simulink model "kinovaMicoSimscapeModel"  (R2021b)
(part 15 of 50)

Y2_9_1=(37*dq4*dqr3*sin(q5))/1000 - (37*dq4*dqr2*sin(q5))/1000 + dq5*dqr2*sin(q5)*((117*3^(1/2))/1250 - 37/2000) - dq5*dqr3*sin(q5)*((117*3^(1/2))/1250 - 37/2000) + (37*dq4*dqr2*cos(q4)^2*sin(q5))/500 - (37*dq4*dqr3*cos(q4)^2*sin(q5))/500 + (37*dq5*dqr2*cos(q4)^2*sin(q5))/2000 - (37*dq5*dqr3*cos(q4)^2*sin(q5))/2000 + (117*dq1*dqr1*cos(q4)*sin(q5))/625 - (234*dq1*dqr1*cos(q2)^2*cos(q4)*sin(q5))/625 - (234*dq1*dqr1*cos(q3)^2*cos(q4)*sin(q5))/625 - (29*3^(1/2)*dq1*dqr1*cos(q5)*sin(q3))/200 - (29*3^(1/2)*dq2*dqr3*cos(q5)*sin(q3))/200 - (29*3^(1/2)*dq3*dqr2*cos(q5)*sin(q3))/200 + (29*3^(1/2)*dq3*dqr3*cos(q5)*sin(q3))/200 - (29*3^(1/2)*dq5*dqr2*cos(q3)*sin(q5))/200 + (29*3^(1/2)*dq5*dqr3*cos(q3)*sin(q5))/200 + (29*dq1*dqr1*cos(q3)*cos(q4)*sin(q5))/100 + (29*dq1*dqr1*cos(q3)*cos(q5)*sin(q4))/200 - (37*dq1*dqr4*cos(q2)*cos(q5)*sin(q3))/1000 + (37*dq1*dqr4*cos(q3)*cos(q5)*sin(q2))/1000 - (37*dq4*dqr1*cos(q2)*cos(q5)*sin(q3))/1000 + (37*dq4*dqr1*cos(q3)*cos(q5)*sin(q2))/1000 - (29*dq1*dqr4*cos(q2)*cos(q5)*sin(q4))/200 - (29*dq4*dqr1*cos(q2)*cos(q4)*sin(q5))/100 - (29*dq4*dqr1*cos(q2)*cos(q5)*sin(q4))/200 - (37*dq5*dqr1*cos(q2)*cos(q5)*sin(q3))/1000 + (37*dq5*dqr1*cos(q3)*cos(q5)*sin(q2))/1000 + (29*dq2*dqr3*cos(q3)*cos(q4)*sin(q5))/100 + (29*dq2*dqr3*cos(q3)*cos(q5)*sin(q4))/200 + (29*dq3*dqr2*cos(q3)*cos(q4)*sin(q5))/100 + (29*dq3*dqr2*cos(q3)*cos(q5)*sin(q4))/200 - (29*dq5*dqr1*cos(q2)*cos(q4)*sin(q5))/200 - (29*dq5*dqr1*cos(q2)*cos(q5)*sin(q4))/100 + (29*dq2*dqr4*cos(q4)*cos(q5)*sin(q3))/200 - (29*dq3*dqr3*cos(q3)*cos(q4)*sin(q5))/100 - (29*dq3*dqr3*cos(q3)*cos(q5)*sin(q4))/200 + (29*dq4*dqr2*cos(q4)*cos(q5)*sin(q3))/200 - (29*dq3*dqr4*cos(q4)*cos(q5)*sin(q3))/200 + (37*dq4*dqr2*cos(q4)*cos(q5)*sin(q4))/1000 - (29*dq4*dqr3*cos(q4)*cos(q5)*sin(q3))/200 + (29*dq5*dqr2*cos(q4)*cos(q5)*sin(q3))/100 - (37*dq4*dqr3*cos(q4)*cos(q5)*sin(q4))/1000 + (37*dq5*dqr2*cos(q4)*cos(q5)*sin(q4))/1000 - (29*dq5*dqr3*cos(q4)*cos(q5)*sin(q3))/100 - (37*dq5*dqr3*cos(q4)*cos(q5)*sin(q4))/1000 - (29*dq2*dqr4*sin(q3)*sin(q4)*sin(q5))/100 - (29*dq4*dqr2*sin(q3)*sin(q4)*sin(q5))/100 + (29*dq3*dqr4*sin(q3)*sin(q4)*sin(q5))/100 + (29*dq4*dqr3*sin(q3)*sin(q4)*sin(q5))/100 - (29*dq5*dqr2*sin(q3)*sin(q4)*sin(q5))/200 + (29*dq5*dqr3*sin(q3)*sin(q4)*sin(q5))/200 - dq1*dqr1*cos(q5)*sin(q4)*((37*3^(1/2))/2000 - 117/1250) + dq1*dqr1*cos(q2)^2*cos(q5)*sin(q4)*((37*3^(1/2))/1000 - 117/625) + dq1*dqr1*cos(q3)^2*cos(q5)*sin(q4)*((37*3^(1/2))/1000 - 117/625) + (468*dq1*dqr1*cos(q2)^2*cos(q3)^2*cos(q4)*sin(q5))/625 + (29*3^(1/2)*dq1*dqr1*cos(q2)^2*cos(q5)*sin(q3))/100 + (117*dq4*dqr1*cos(q2)*cos(q3)*cos(q4)*sin(q5))/625 + (117*dq5*dqr1*cos(q2)*cos(q3)*cos(q4)*sin(q5))/1250 + (117*dq5*dqr1*cos(q2)*cos(q3)*cos(q5)*sin(q4))/625 + (117*dq1*dqr4*cos(q4)*sin(q2)*sin(q3)*sin(q5))/625 + (117*dq4*dqr1*cos(q4)*sin(q2)*sin(q3)*sin(q5))/625 + (117*dq5*dqr1*cos(q4)*sin(q2)*sin(q3)*sin(q5))/1250 + (117*dq5*dqr1*cos(q5)*sin(q2)*sin(q3)*sin(q4))/625 - dq1*dqr1*cos(q2)*cos(q5)*sin(q2)*((117*3^(1/2))/625 + 37/1000) + dq1*dqr1*cos(q3)*cos(q5)*sin(q3)*((117*3^(1/2))/625 + 37/1000) + (37*dq1*dqr1*cos(q2)*cos(q4)^2*cos(q5)*sin(q2))/1000 - (29*dq1*dqr1*cos(q2)^2*cos(q3)*cos(q4)*sin(q5))/50 - (29*dq1*dqr1*cos(q2)^2*cos(q3)*cos(q5)*sin(q4))/100 - (37*dq1*dqr1*cos(q3)*cos(q4)^2*cos(q5)*sin(q3))/1000 + (37*dq1*dqr4*cos(q2)*cos(q4)^2*cos(q5)*sin(q3))/1000 - (37*dq1*dqr4*cos(q3)*cos(q4)^2*cos(q5)*sin(q2))/1000 + (37*dq4*dqr1*cos(q2)*cos(q4)^2*cos(q5)*sin(q3))/1000 - (37*dq4*dqr1*cos(q3)*cos(q4)^2*cos(q5)*sin(q2))/1000 + (37*dq5*dqr1*cos(q2)*cos(q4)^2*cos(q5)*sin(q3))/1000 - (37*dq5*dqr1*cos(q3)*cos(q4)^2*cos(q5)*sin(q2))/1000 + dq1*dqr1*cos(q2)*cos(q3)^2*cos(q5)*sin(q2)*((234*3^(1/2))/625 + 37/500) - dq1*dqr1*cos(q2)^2*cos(q3)*cos(q5)*sin(q3)*((234*3^(1/2))/625 + 37/500) - (37*dq1*dqr1*cos(q2)*cos(q3)^2*cos(q4)^2*cos(q5)*sin(q2))/500 + (37*dq1*dqr1*cos(q2)^2*cos(q3)*cos(q4)^2*cos(q5)*sin(q3))/500 - dq1*dqr1*cos(q2)^2*cos(q3)^2*cos(q5)*sin(q4)*((37*3^(1/2))/500 - 234/625) - (29*dq1*dqr1*cos(q2)*cos(q4)*sin(q2)*sin(q3)*sin(q5))/50 - (29*dq1*dqr1*cos(q2)*cos(q5)*sin(q2)*sin(q3)*sin(q4))/100 - (37*dq1*dqr1*cos(q2)*cos(q4)*sin(q2)*sin(q4)*sin(q5))/500 + (37*dq1*dqr1*cos(q3)*cos(q4)*sin(q3)*sin(q4)*sin(q5))/500 - (37*dq1*dqr4*cos(q2)*cos(q4)*sin(q3)*sin(q4)*sin(q5))/500 + (37*dq1*dqr4*cos(q3)*cos(q4)*sin(q2)*sin(q4)*sin(q5))/500 - (37*dq4*dqr1*cos(q2)*cos(q4)*sin(q3)*sin(q4)*sin(q5))/500 + (37*dq4*dqr1*cos(q3)*cos(q4)*sin(q2)*sin(q4)*sin(q5))/500 - (37*dq5*dqr1*cos(q2)*cos(q4)*sin(q3)*sin(q4)*sin(q5))/2000 + (37*dq5*dqr1*cos(q3)*cos(q4)*sin(q2)*sin(q4)*sin(q5))/2000 - dq1*dqr4*cos(q2)*cos(q3)*cos(q5)*sin(q4)*((37*3^(1/2))/2000 - 117/1250) - dq4*dqr1*cos(q2)*cos(q3)*cos(q5)*sin(q4)*((37*3^(1/2))/2000 - 117/1250) - dq1*dqr4*cos(q5)*sin(q2)*sin(q3)*sin(q4)*((37*3^(1/2))/2000 - 117/1250) - dq4*dqr1*cos(q5)*sin(q2)*sin(q3)*sin(q4)*((37*3^(1/2))/2000 - 117/1250) - (29*3^(1/2)*dq1*dqr1*cos(q2)*cos(q3)*cos(q5)*sin(q2))/100 + (468*dq1*dqr1*cos(q2)*cos(q3)*cos(q4)*sin(q2)*sin(q3)*sin(q5))/625 + (37*dq1*dqr1*cos(q2)*cos(q3)^2*cos(q4)*sin(q2)*sin(q4)*sin(q5))/250 - (37*dq1*dqr1*cos(q2)^2*cos(q3)*cos(q4)*sin(q3)*sin(q4)*sin(q5))/250 - dq1*dqr1*cos(q2)*cos(q3)*cos(q5)*sin(q2)*sin(q3)*sin(q4)*((37*3^(1/2))/500 - 234/625);
Y2_9_2=(37*dq3*dqr4*sin(q5))/1000 - (37*dq2*dqr4*sin(q5))/1000 - (117*ddqr5*cos(q4)*cos(q5))/625 + (117*ddqr4*sin(q4)*sin(q5))/625 - ddqr2*cos(q5)*((117*3^(1/2))/625 - 37/1000) + ddqr3*cos(q5)*((117*3^(1/2))/625 - 37/1000) - (37*ddqr2*cos(q4)^2*cos(q5))/1000 + (37*ddqr3*cos(q4)^2*cos(q5))/1000 + dq2*dqr5*sin(q5)*((117*3^(1/2))/1250 - 37/2000) - dq3*dqr5*sin(q5)*((117*3^(1/2))/1250 - 37/2000) + (37*dq2*dqr4*cos(q4)^2*sin(q5))/500 + (37*dq2*dqr5*cos(q4)^2*sin(q5))/2000 - (37*dq3*dqr4*cos(q4)^2*sin(q5))/500 - (37*dq3*dqr5*cos(q4)^2*sin(q5))/2000 + (29*ddqr1*cos(q2)*cos(q4)*cos(q5))/200 + (29*ddqr4*cos(q3)*cos(q4)*cos(q5))/200 + (29*ddqr5*cos(q3)*cos(q4)*cos(q5))/100 - (37*ddqr1*cos(q2)*sin(q3)*sin(q5))/1000 + (37*ddqr1*cos(q3)*sin(q2)*sin(q5))/1000 - (29*ddqr1*cos(q2)*sin(q4)*sin(q5))/100 + (29*ddqr2*cos(q4)*sin(q3)*sin(q5))/50 + (29*ddqr2*cos(q5)*sin(q3)*sin(q4))/100 + (37*ddqr2*cos(q4)*sin(q4)*sin(q5))/500 - (29*ddqr3*cos(q4)*sin(q3)*sin(q5))/100 - (29*ddqr3*cos(q5)*sin(q3)*sin(q4))/200 - (37*ddqr3*cos(q4)*sin(q4)*sin(q5))/500 - (29*ddqr4*cos(q3)*sin(q4)*sin(q5))/100 - (29*ddqr5*cos(q3)*sin(q4)*sin(q5))/200 + ddqr4*cos(q4)*cos(q5)*((37*3^(1/2))/2000 - 117/1250) + ddqr5*sin(q4)*sin(q5)*((37*3^(1/2))/2000 + 117/1250) + (29*3^(1/2)*ddqr2*cos(q3)*cos(q5))/100 - (29*3^(1/2)*ddqr3*cos(q3)*cos(q5))/200 + (117*dq4*dqr4*cos(q4)*sin(q5))/625 + (117*dq4*dqr5*cos(q4)*sin(q5))/1250 + (117*dq4*dqr5*cos(q5)*sin(q4))/625 + (117*dq5*dqr4*cos(q4)*sin(q5))/1250 + (117*dq5*dqr4*cos(q5)*sin(q4))/625 + (117*dq5*dqr5*cos(q4)*sin(q5))/625 + (29*3^(1/2)*ddqr5*sin(q3)*sin(q5))/200 + (117*ddqr1*cos(q2)*cos(q3)*sin(q4)*sin(q5))/625 - (7*ddqr1*cos(q2)*cos(q4)*sin(q3)*sin(q5))/1000 - (7*ddqr1*cos(q2)*cos(q5)*sin(q3)*sin(q4))/2000 + (7*ddqr1*cos(q3)*cos(q4)*sin(q2)*sin(q5))/1000 + (7*ddqr1*cos(q3)*cos(q5)*sin(q2)*sin(q4))/2000 - (29*3^(1/2)*dq2*dqr5*cos(q3)*sin(q5))/200 + (29*3^(1/2)*dq3*dqr5*cos(q3)*sin(q5))/200 + (29*3^(1/2)*dq5*dqr5*cos(q5)*sin(q3))/200 + (117*ddqr1*sin(q2)*sin(q3)*sin(q4)*sin(q5))/625 + (37*ddqr1*cos(q2)*cos(q4)^2*sin(q3)*sin(q5))/500 - (37*ddqr1*cos(q3)*cos(q4)^2*sin(q2)*sin(q5))/500 - (7*3^(1/2)*ddqr1*cos(q2)*cos(q3)*cos(q5))/2000 - (29*dq1*dqr4*cos(q2)*cos(q4)*sin(q5))/100 - (37*dq1*dqr5*cos(q2)*cos(q5)*sin(q3))/1000 + (37*dq1*dqr5*cos(q3)*cos(q5)*sin(q2))/1000 - (29*dq1*dqr5*cos(q2)*cos(q4)*sin(q5))/200 - (29*dq1*dqr5*cos(q2)*cos(q5)*sin(q4))/100 + (37*dq2*dqr4*cos(q4)*cos(q5)*sin(q4))/1000 + (29*dq2*dqr5*cos(q4)*cos(q5)*sin(q3))/100 + (37*dq2*dqr5*cos(q4)*cos(q5)*sin(q4))/1000 - (37*dq3*dqr4*cos(q4)*cos(q5)*sin(q4))/1000 - (29*dq3*dqr5*cos(q4)*cos(q5)*sin(q3))/100 - (29*dq4*dqr4*cos(q3)*cos(q4)*sin(q5))/100 - (29*dq4*dqr4*cos(q3)*cos(q5)*sin(q4))/200 - (37*dq3*dqr5*cos(q4)*cos(q5)*sin(q4))/1000 - (29*dq4*dqr5*cos(q3)*cos(q4)*sin(q5))/200 - (29*dq4*dqr5*cos(q3)*cos(q5)*sin(q4))/100 - (29*dq5*dqr4*cos(q3)*cos(q4)*sin(q5))/200 - (29*dq5*dqr4*cos(q3)*cos(q5)*sin(q4))/100 - (29*dq5*dqr5*cos(q3)*cos(q4)*sin(q5))/100 - (29*dq5*dqr5*cos(q3)*cos(q5)*sin(q4))/200 - (7*3^(1/2)*ddqr1*cos(q5)*sin(q2)*sin(q3))/2000 - (29*dq2*dqr5*sin(q3)*sin(q4)*sin(q5))/200 + (29*dq3*dqr5*sin(q3)*sin(q4)*sin(q5))/200 - dq4*dqr4*cos(q5)*sin(q4)*((37*3^(1/2))/2000 - 117/1250) + dq5*dqr5*cos(q5)*sin(q4)*((37*3^(1/2))/2000 + 117/1250) + (37*ddqr1*cos(q2)*cos(q4)*cos(q5)*sin(q3)*sin(q4))/1000 - (37*ddqr1*cos(q3)*cos(q4)*cos(q5)*sin(q2)*sin(q4))/1000 + ddqr1*cos(q2)*cos(q3)*cos(q4)*cos(q5)*((37*3^(1/2))/2000 - 117/1250) + ddqr1*cos(q4)*cos(q5)*sin(q2)*sin(q3)*((37*3^(1/2))/2000 - 117/1250) + (117*dq1*dqr4*cos(q2)*cos(q3)*cos(q4)*sin(q5))/625 + (117*dq1*dqr5*cos(q2)*cos(q3)*cos(q4)*sin(q5))/1250 + (117*dq1*dqr5*cos(q2)*cos(q3)*cos(q5)*sin(q4))/625 + (117*dq1*dqr5*cos(q4)*sin(q2)*sin(q3)*sin(q5))/1250 + (117*dq1*dqr5*cos(q5)*sin(q2)*sin(q3)*sin(q4))/625 + (37*dq1*dqr5*cos(q2)*cos(q4)^2*cos(q5)*sin(q3))/1000 - (37*dq1*dqr5*cos(q3)*cos(q4)^2*cos(q5)*sin(q2))/1000 - (37*dq1*dqr5*cos(q2)*cos(q4)*sin(q3)*sin(q4)*sin(q5))/2000 + (37*dq1*dqr5*cos(q3)*cos(q4)*sin(q2)*sin(q4)*sin(q5))/2000;
Y2_10_1=dq1*dqr1*cos(q2)*cos(q3)^2*cos(q6)*sin(q2)*((1231*3^(1/2))/10000 - 111/1000) - (2631*dq6*dqr1*cos(q4)*sin(q2)*sin(q3)*sin(q6))/16000 - dq1*dqr1*cos(q2)*cos(q4)^2*cos(q6)*sin(q2)*((1923*3^(1/2))/40000 + 37/400) + (37*3^(1/2)*dq4*dqr1*cos(q4)*sin(q2)*sin(q3)*sin(q6))/2000 + (37*3^(1/2)*dq5*dqr1*cos(q4)*sin(q2)*sin(q3)*sin(q6))/4000 - (37*dq1*dqr1*cos(q2)*cos(q3)^2*cos(q5)^2*cos(q6)*sin(q2))/1000 + (37*dq1*dqr1*cos(q2)*cos(q4)^2*cos(q5)^2*cos(q6)*sin(q2))/800 + (87*dq1*dqr1*cos(q2)*cos(q6)*sin(q2)*sin(q3)*sin(q4))/200 + (37*dq1*dqr1*cos(q2)*cos(q4)*sin(q2)*sin(q4)*sin(q6))/1000 - (37*dq1*dqr1*cos(q2)*cos(q5)*sin(q2)*sin(q5)*sin(q6))/1000 - (37*dq4*dqr1*cos(q3)*cos(q4)*sin(q2)*sin(q4)*sin(q6))/1000 - (877*dq4*dqr1*cos(q4)*cos(q5)*sin(q2)*sin(q3)*sin(q6))/4000 - (1231*dq4*dqr1*cos(q5)*cos(q6)*sin(q2)*sin(q3)*sin(q4))/40000 - (37*dq5*dqr1*cos(q3)*cos(q4)*sin(q2)*sin(q4)*sin(q6))/800 - (37*dq4*dqr1*cos(q3)*cos(q5)*sin(q2)*sin(q5)*sin(q6))/2000 - (877*dq5*dqr1*cos(q4)*cos(q5)*sin(q2)*sin(q3)*sin(q6))/8000 - (37*dq5*dqr1*cos(q3)*cos(q5)*sin(q2)*sin(q5)*sin(q6))/1000 - (877*dq6*dqr1*cos(q4)*cos(q6)*sin(q2)*sin(q3)*sin(q5))/8000 - (877*dq6*dqr1*cos(q5)*cos(q6)*sin(q2)*sin(q3)*sin(q4))/4000 - (37*dq6*dqr1*cos(q3)*cos(q5)*sin(q2)*sin(q5)*sin(q6))/4000 + (877*dq5*dqr1*sin(q2)*sin(q3)*sin(q4)*sin(q5)*sin(q6))/4000 + (877*dq6*dqr1*sin(q2)*sin(q3)*sin(q4)*sin(q5)*sin(q6))/8000 - dq1*dqr1*cos(q2)*sin(q2)*sin(q5)*sin(q6)*((2513*3^(1/2))/10000 + 37/1000) + dq4*dqr1*cos(q3)*sin(q2)*sin(q5)*sin(q6)*((641*3^(1/2))/20000 + 37/1000) + dq5*dqr1*cos(q3)*sin(q2)*sin(q5)*sin(q6)*((641*3^(1/2))/20000 + 37/1000) + dq6*dqr1*cos(q3)*sin(q2)*sin(q5)*sin(q6)*((641*3^(1/2))/40000 + 37/2000) - dq4*dqr1*cos(q6)*sin(q2)*sin(q3)*sin(q4)*((37*3^(1/2))/4000 + 7539/40000) - (29*3^(1/2)*dq1*dqr1*cos(q2)*cos(q3)*cos(q6)*sin(q2))/200 + dq1*dqr1*cos(q2)*cos(q3)^2*cos(q4)^2*cos(q6)*sin(q2)*((1923*3^(1/2))/20000 + 37/200) - (37*3^(1/2)*dq4*dqr1*cos(q4)*cos(q5)^2*sin(q2)*sin(q3)*sin(q6))/1000 - (37*3^(1/2)*dq4*dqr1*cos(q5)^2*cos(q6)*sin(q2)*sin(q3)*sin(q4))/4000 - (37*3^(1/2)*dq5*dqr1*cos(q4)*cos(q5)^2*sin(q2)*sin(q3)*sin(q6))/2000 - (37*3^(1/2)*dq5*dqr1*cos(q5)^2*cos(q6)*sin(q2)*sin(q3)*sin(q4))/2000 - (37*3^(1/2)*dq6*dqr1*cos(q4)*cos(q5)^2*sin(q2)*sin(q3)*sin(q6))/8000 - (37*3^(1/2)*dq6*dqr1*cos(q5)^2*cos(q6)*sin(q2)*sin(q3)*sin(q4))/2000 - (37*dq1*dqr1*cos(q2)*cos(q3)^2*cos(q4)^2*cos(q5)^2*cos(q6)*sin(q2))/400 + (29*dq1*dqr1*cos(q2)*cos(q4)*cos(q5)*sin(q2)*sin(q3)*sin(q6))/50 + (29*dq1*dqr1*cos(q2)*cos(q4)*cos(q6)*sin(q2)*sin(q3)*sin(q5))/100 + (29*dq1*dqr1*cos(q2)*cos(q5)*cos(q6)*sin(q2)*sin(q3)*sin(q4))/200 - (29*dq1*dqr1*cos(q2)*sin(q2)*sin(q3)*sin(q4)*sin(q5)*sin(q6))/100 + dq4*dqr1*cos(q4)*cos(q6)*sin(q2)*sin(q3)*sin(q5)*((37*3^(1/2))/4000 - 877/8000) + dq5*dqr1*cos(q5)*cos(q6)*sin(q2)*sin(q3)*sin(q4)*((37*3^(1/2))/4000 - 877/8000) + dq5*dqr1*cos(q4)*cos(q6)*sin(q2)*sin(q3)*sin(q5)*((37*3^(1/2))/8000 - 877/16000) - dq6*dqr1*cos(q4)*cos(q5)*sin(q2)*sin(q3)*sin(q6)*((111*3^(1/2))/8000 + 877/16000) - dq6*dqr1*cos(q3)*cos(q4)*sin(q2)*sin(q4)*sin(q6)*((1923*3^(1/2))/80000 + 37/800) - (37*dq1*dqr1*cos(q2)*cos(q3)^2*cos(q4)*sin(q2)*sin(q4)*sin(q6))/500 - (37*dq1*dqr1*cos(q2)*cos(q4)*cos(q5)^2*sin(q2)*sin(q4)*sin(q6))/500 + (37*dq1*dqr1*cos(q2)*cos(q3)^2*cos(q5)*sin(q2)*sin(q5)*sin(q6))/500 - (37*dq1*dqr1*cos(q2)*cos(q4)^2*cos(q5)*sin(q2)*sin(q5)*sin(q6))/400 + (37*dq4*dqr1*cos(q3)*cos(q4)*cos(q5)^2*sin(q2)*sin(q4)*sin(q6))/500 + (37*dq4*dqr1*cos(q3)*cos(q4)^2*cos(q5)*sin(q2)*sin(q5)*sin(q6))/400 + (37*dq5*dqr1*cos(q3)*cos(q4)*cos(q5)^2*sin(q2)*sin(q4)*sin(q6))/400 + (37*dq5*dqr1*cos(q3)*cos(q4)^2*cos(q5)*sin(q2)*sin(q5)*sin(q6))/500 + (37*dq6*dqr1*cos(q3)*cos(q4)*cos(q5)^2*sin(q2)*sin(q4)*sin(q6))/1600 + (37*dq6*dqr1*cos(q3)*cos(q4)^2*cos(q5)*sin(q2)*sin(q5)*sin(q6))/2000 - dq4*dqr1*sin(q2)*sin(q3)*sin(q4)*sin(q5)*sin(q6)*((37*3^(1/2))/2000 - 1231/20000) + (29*3^(1/2)*dq1*dqr1*cos(q2)*cos(q3)*cos(q5)*cos(q6)*sin(q2))/200 - dq1*dqr1*cos(q2)*cos(q3)^2*cos(q5)*cos(q6)*sin(q2)*((2513*3^(1/2))/10000 - 37/500) - dq1*dqr1*cos(q2)*cos(q4)^2*cos(q5)*cos(q6)*sin(q2)*((641*3^(1/2))/40000 - 37/4000) - (29*3^(1/2)*dq1*dqr1*cos(q2)*cos(q3)*sin(q2)*sin(q5)*sin(q6))/100 + dq1*dqr1*cos(q2)*cos(q3)^2*sin(q2)*sin(q5)*sin(q6)*((2513*3^(1/2))/5000 + 37/500) + dq1*dqr1*cos(q2)*cos(q4)^2*sin(q2)*sin(q5)*sin(q6)*((641*3^(1/2))/20000 + 37/1000) - dq4*dqr1*cos(q3)*cos(q4)^2*sin(q2)*sin(q5)*sin(q6)*((641*3^(1/2))/20000 + 37/1000) - dq5*dqr1*cos(q3)*cos(q4)^2*sin(q2)*sin(q5)*sin(q6)*((641*3^(1/2))/20000 + 37/1000) - dq6*dqr1*cos(q3)*cos(q4)^2*sin(q2)*sin(q5)*sin(q6)*((641*3^(1/2))/40000 - 37/4000) + dq1*dqr1*cos(q2)*cos(q3)^2*cos(q4)^2*cos(q5)*cos(q6)*sin(q2)*((641*3^(1/2))/20000 - 37/2000) - (877*dq1*dqr1*cos(q2)*cos(q3)*cos(q4)*cos(q5)*sin(q2)*sin(q3)*sin(q6))/1000 - (1231*dq1*dqr1*cos(q2)*cos(q3)*cos(q5)*cos(q6)*sin(q2)*sin(q3)*sin(q4))/10000 - (37*dq1*dqr1*cos(q2)*cos(q4)*cos(q5)*cos(q6)*sin(q2)*sin(q4)*sin(q5))/1000 + (37*dq4*dqr1*cos(q3)*cos(q4)*cos(q5)*cos(q6)*sin(q2)*sin(q4)*sin(q5))/1000 + (37*dq5*dqr1*cos(q3)*cos(q4)*cos(q5)*cos(q6)*sin(q2)*sin(q4)*sin(q5))/800 + (37*dq6*dqr1*cos(q3)*cos(q4)*cos(q5)*cos(q6)*sin(q2)*sin(q4)*sin(q5))/800 - dq1*dqr1*cos(q2)*cos(q3)^2*cos(q4)^2*sin(q2)*sin(q5)*sin(q6)*((641*3^(1/2))/10000 + 37/500) + dq1*dqr1*cos(q2)*cos(q4)*cos(q5)*sin(q2)*sin(q4)*sin(q6)*((641*3^(1/2))/10000 + 37/500) - dq4*dqr1*cos(q3)*cos(q4)*cos(q5)*sin(q2)*sin(q4)*sin(q6)*((641*3^(1/2))/10000 + 37/500) - dq1*dqr1*cos(q2)*cos(q3)*cos(q6)*sin(q2)*sin(q3)*sin(q4)*((37*3^(1/2))/1000 + 7539/10000) + dq1*dqr1*cos(q2)*cos(q4)*cos(q6)*sin(q2)*sin(q4)*sin(q5)*((641*3^(1/2))/20000 - 37/2000) - dq4*dqr1*cos(q3)*cos(q4)*cos(q6)*sin(q2)*sin(q4)*sin(q5)*((641*3^(1/2))/20000 - 37/2000) - dq5*dqr1*cos(q3)*cos(q4)*cos(q5)*sin(q2)*sin(q4)*sin(q6)*((641*3^(1/2))/40000 + 37/2000) - dq6*dqr1*cos(q3)*cos(q4)*cos(q6)*sin(q2)*sin(q4)*sin(q5)*((641*3^(1/2))/40000 + 37/2000) - dq5*dqr1*cos(q3)*cos(q4)*cos(q6)*sin(q2)*sin(q4)*sin(q5)*((641*3^(1/2))/80000 - 37/8000) - dq6*dqr1*cos(q3)*cos(q4)*cos(q5)*sin(q2)*sin(q4)*sin(q6)*((641*3^(1/2))/80000 - 37/8000) + (37*3^(1/2)*dq1*dqr1*cos(q2)*cos(q3)*cos(q4)*sin(q2)*sin(q3)*sin(q6))/500 - (37*3^(1/2)*dq4*dqr1*cos(q4)*cos(q5)*cos(q6)*sin(q2)*sin(q3)*sin(q5))/2000 - (37*3^(1/2)*dq5*dqr1*cos(q4)*cos(q5)*cos(q6)*sin(q2)*sin(q3)*sin(q5))/4000 - (37*3^(1/2)*dq6*dqr1*cos(q4)*cos(q5)*cos(q6)*sin(q2)*sin(q3)*sin(q5))/4000 + (37*3^(1/2)*dq4*dqr1*cos(q5)*sin(q2)*sin(q3)*sin(q4)*sin(q5)*sin(q6))/2000 + (37*3^(1/2)*dq5*dqr1*cos(q5)*sin(q2)*sin(q3)*sin(q4)*sin(q5)*sin(q6))/1000 + (37*3^(1/2)*dq6*dqr1*cos(q5)*sin(q2)*sin(q3)*sin(q4)*sin(q5)*sin(q6))/4000 + (37*dq1*dqr1*cos(q2)*cos(q3)^2*cos(q4)*cos(q5)^2*sin(q2)*sin(q4)*sin(q6))/250 + (37*dq1*dqr1*cos(q2)*cos(q3)^2*cos(q4)^2*cos(q5)*sin(q2)*sin(q5)*sin(q6))/200 + dq1*dqr1*cos(q2)*cos(q3)*cos(q4)*cos(q6)*sin(q2)*sin(q3)*sin(q5)*((37*3^(1/2))/1000 - 877/2000) + (37*dq1*dqr1*cos(q2)*cos(q3)^2*cos(q4)*cos(q5)*cos(q6)*sin(q2)*sin(q4)*sin(q5))/500 - dq1*dqr1*cos(q2)*cos(q3)*sin(q2)*sin(q3)*sin(q4)*sin(q5)*sin(q6)*((37*3^(1/2))/500 - 1231/5000) - dq1*dqr1*cos(q2)*cos(q3)^2*cos(q4)*cos(q5)*sin(q2)*sin(q4)*sin(q6)*((641*3^(1/2))/5000 + 37/250) - dq1*dqr1*cos(q2)*cos(q3)^2*cos(q4)*cos(q6)*sin(q2)*sin(q4)*sin(q5)*((641*3^(1/2))/10000 - 37/1000) - (37*3^(1/2)*dq1*dqr1*cos(q2)*cos(q3)*cos(q4)*cos(q5)^2*sin(q2)*sin(q3)*sin(q6))/250 - (37*3^(1/2)*dq1*dqr1*cos(q2)*cos(q3)*cos(q5)^2*cos(q6)*sin(q2)*sin(q3)*sin(q4))/1000 - (37*3^(1/2)*dq1*dqr1*cos(q2)*cos(q3)*cos(q4)*cos(q5)*cos(q6)*sin(q2)*sin(q3)*sin(q5))/500 + (37*3^(1/2)*dq1*dqr1*cos(q2)*cos(q3)*cos(q5)*sin(q2)*sin(q3)*sin(q4)*sin(q5)*sin(q6))/500;
Y2_10_2=(29*3^(1/2)*dq1*dqr1*cos(q5)*cos(q6)*sin(q3))/400 - (29*3^(1/2)*dq1*dqr1*cos(q6)*sin(q3))/400 - (29*3^(1/2)*dq1*dqr1*sin(q3)*sin(q5)*sin(q6))/200 + (29*3^(1/2)*dq1*dqr1*cos(q2)^2*cos(q6)*sin(q3))/200 - dq1*dqr1*cos(q2)*cos(q6)*sin(q2)*((1231*3^(1/2))/20000 - 111/2000) + dq1*dqr1*cos(q3)*cos(q6)*sin(q3)*((1231*3^(1/2))/20000 - 111/2000) + dq4*dqr1*cos(q2)*cos(q6)*sin(q3)*((1923*3^(1/2))/40000 + 111/2000) - dq4*dqr1*cos(q3)*cos(q6)*sin(q2)*((1923*3^(1/2))/40000 + 111/2000) + (37*dq1*dqr1*cos(q2)*cos(q5)^2*cos(q6)*sin(q2))/2000 - (37*dq1*dqr1*cos(q3)*cos(q5)^2*cos(q6)*sin(q3))/2000 - (37*dq4*dqr1*cos(q2)*cos(q5)^2*cos(q6)*sin(q3))/4000 + (37*dq4*dqr1*cos(q3)*cos(q5)^2*cos(q6)*sin(q2))/4000 - (37*dq5*dqr1*cos(q2)*cos(q4)^2*cos(q6)*sin(q3))/2000 + (37*dq5*dqr1*cos(q3)*cos(q4)^2*cos(q6)*sin(q2))/2000 - (37*dq5*dqr1*cos(q2)*cos(q5)^2*cos(q6)*sin(q3))/2000 + (37*dq5*dqr1*cos(q3)*cos(q5)^2*cos(q6)*sin(q2))/2000 - (37*dq6*dqr1*cos(q2)*cos(q4)^2*cos(q6)*sin(q3))/2000 + (37*dq6*dqr1*cos(q3)*cos(q4)^2*cos(q6)*sin(q2))/2000 - (37*dq6*dqr1*cos(q2)*cos(q5)^2*cos(q6)*sin(q3))/2000 + (37*dq6*dqr1*cos(q3)*cos(q5)^2*cos(q6)*sin(q2))/2000 - dq1*dqr1*cos(q2)^2*cos(q3)*cos(q6)*sin(q3)*((1231*3^(1/2))/10000 - 111/1000) + dq1*dqr1*cos(q3)*cos(q4)^2*cos(q6)*sin(q3)*((1923*3^(1/2))/40000 + 37/400) - dq4*dqr1*cos(q2)*cos(q4)^2*cos(q6)*sin(q3)*((1923*3^(1/2))/40000 + 37/400) + dq4*dqr1*cos(q3)*cos(q4)^2*cos(q6)*sin(q2)*((1923*3^(1/2))/40000 + 37/400) + (37*dq1*dqr1*cos(q2)^2*cos(q3)*cos(q5)^2*cos(q6)*sin(q3))/1000 - (37*dq1*dqr1*cos(q3)*cos(q4)^2*cos(q5)^2*cos(q6)*sin(q3))/800 + (37*dq4*dqr1*cos(q2)*cos(q4)^2*cos(q5)^2*cos(q6)*sin(q3))/800 - (37*dq4*dqr1*cos(q3)*cos(q4)^2*cos(q5)^2*cos(q6)*sin(q2))/800 + (37*dq5*dqr1*cos(q2)*cos(q4)^2*cos(q5)^2*cos(q6)*sin(q3))/1000 - (37*dq5*dqr1*cos(q3)*cos(q4)^2*cos(q5)^2*cos(q6)*sin(q2))/1000 + (37*dq6*dqr1*cos(q2)*cos(q4)^2*cos(q5)^2*cos(q6)*sin(q3))/1000 - (37*dq6*dqr1*cos(q3)*cos(q4)^2*cos(q5)^2*cos(q6)*sin(q2))/1000 - (29*3^(1/2)*dq1*dqr1*cos(q2)^2*cos(q5)*cos(q6)*sin(q3))/200 + (29*3^(1/2)*dq1*dqr1*cos(q2)^2*sin(q3)*sin(q5)*sin(q6))/100 - (37*dq1*dqr1*cos(q3)*cos(q4)*sin(q3)*sin(q4)*sin(q6))/1000 + (37*dq1*dqr1*cos(q3)*cos(q5)*sin(q3)*sin(q5)*sin(q6))/1000 + (37*dq4*dqr1*cos(q2)*cos(q4)*sin(q3)*sin(q4)*sin(q6))/1000 + (37*dq5*dqr1*cos(q2)*cos(q4)*sin(q3)*sin(q4)*sin(q6))/800 + (37*dq4*dqr1*cos(q2)*cos(q5)*sin(q3)*sin(q5)*sin(q6))/2000 + (37*dq5*dqr1*cos(q2)*cos(q5)*sin(q3)*sin(q5)*sin(q6))/1000 + (37*dq6*dqr1*cos(q2)*cos(q5)*sin(q3)*sin(q5)*sin(q6))/4000 + dq6*dqr1*cos(q2)*cos(q5)*cos(q6)*sin(q3)*((641*3^(1/2))/20000 + 37/1000) - dq6*dqr1*cos(q3)*cos(q5)*cos(q6)*sin(q2)*((641*3^(1/2))/20000 + 37/1000) + dq1*dqr1*cos(q2)*cos(q5)*cos(q6)*sin(q2)*((2513*3^(1/2))/20000 - 37/1000) - dq1*dqr1*cos(q3)*cos(q5)*cos(q6)*sin(q3)*((2513*3^(1/2))/20000 - 37/1000) + dq4*dqr1*cos(q2)*cos(q5)*cos(q6)*sin(q3)*((641*3^(1/2))/40000 - 37/4000) - dq4*dqr1*cos(q3)*cos(q5)*cos(q6)*sin(q2)*((641*3^(1/2))/40000 - 37/4000) + dq5*dqr1*cos(q2)*cos(q5)*cos(q6)*sin(q3)*((641*3^(1/2))/40000 - 37/4000) - dq5*dqr1*cos(q3)*cos(q5)*cos(q6)*sin(q2)*((641*3^(1/2))/40000 - 37/4000) + dq1*dqr1*cos(q3)*sin(q3)*sin(q5)*sin(q6)*((2513*3^(1/2))/10000 + 37/1000) - dq4*dqr1*cos(q2)*sin(q3)*sin(q5)*sin(q6)*((641*3^(1/2))/20000 + 37/1000) - dq5*dqr1*cos(q2)*sin(q3)*sin(q5)*sin(q6)*((641*3^(1/2))/20000 + 37/1000) - dq6*dqr1*cos(q2)*sin(q3)*sin(q5)*sin(q6)*((641*3^(1/2))/40000 + 37/2000) - dq1*dqr1*cos(q2)^2*cos(q3)*cos(q4)^2*cos(q6)*sin(q3)*((1923*3^(1/2))/20000 + 37/200) + (37*dq1*dqr1*cos(q2)^2*cos(q3)*cos(q4)^2*cos(q5)^2*cos(q6)*sin(q3))/400 - dq1*dqr1*cos(q2)^2*cos(q3)^2*sin(q4)*sin(q5)*sin(q6)*((37*3^(1/2))/500 - 1231/5000) + dq6*dqr1*cos(q2)*cos(q4)*sin(q3)*sin(q4)*sin(q6)*((1923*3^(1/2))/80000 + 37/800) + (37*dq1*dqr1*cos(q2)^2*cos(q3)*cos(q4)*sin(q3)*sin(q4)*sin(q6))/500 - (37*dq1*dqr1*cos(q2)^2*cos(q3)*cos(q5)*sin(q3)*sin(q5)*sin(q6))/500 + (37*dq1*dqr1*cos(q3)*cos(q4)*cos(q5)^2*sin(q3)*sin(q4)*sin(q6))/500 + (37*dq1*dqr1*cos(q3)*cos(q4)^2*cos(q5)*sin(q3)*sin(q5)*sin(q6))/400 - (37*dq4*dqr1*cos(q2)*cos(q4)*cos(q5)^2*sin(q3)*sin(q4)*sin(q6))/500 - (37*dq4*dqr1*cos(q2)*cos(q4)^2*cos(q5)*sin(q3)*sin(q5)*sin(q6))/400 - (37*dq5*dqr1*cos(q2)*cos(q4)*cos(q5)^2*sin(q3)*sin(q4)*sin(q6))/400 - (37*dq5*dqr1*cos(q2)*cos(q4)^2*cos(q5)*sin(q3)*sin(q5)*sin(q6))/500 - (37*dq6*dqr1*cos(q2)*cos(q4)*cos(q5)^2*sin(q3)*sin(q4)*sin(q6))/1600 - (37*dq6*dqr1*cos(q2)*cos(q4)^2*cos(q5)*sin(q3)*sin(q5)*sin(q6))/2000 + dq1*dqr1*cos(q2)^2*cos(q3)*cos(q5)*cos(q6)*sin(q3)*((2513*3^(1/2))/10000 - 37/500) - dq6*dqr1*cos(q2)*cos(q4)^2*cos(q5)*cos(q6)*sin(q3)*((641*3^(1/2))/20000 + 37/1000) + dq6*dqr1*cos(q3)*cos(q4)^2*cos(q5)*cos(q6)*sin(q2)*((641*3^(1/2))/20000 + 37/1000) + dq1*dqr1*cos(q3)*cos(q4)^2*cos(q5)*cos(q6)*sin(q3)*((641*3^(1/2))/40000 - 37/4000) - dq4*dqr1*cos(q2)*cos(q4)^2*cos(q5)*cos(q6)*sin(q3)*((641*3^(1/2))/40000 - 37/4000) + dq4*dqr1*cos(q3)*cos(q4)^2*cos(q5)*cos(q6)*sin(q2)*((641*3^(1/2))/40000 - 37/4000) - dq5*dqr1*cos(q2)*cos(q4)^2*cos(q5)*cos(q6)*sin(q3)*((641*3^(1/2))/40000 - 37/4000) + dq5*dqr1*cos(q3)*cos(q4)^2*cos(q5)*cos(q6)*sin(q2)*((641*3^(1/2))/40000 - 37/4000) - dq1*dqr1*cos(q2)^2*cos(q3)*sin(q3)*sin(q5)*sin(q6)*((2513*3^(1/2))/5000 + 37/500) - dq1*dqr1*cos(q3)*cos(q4)^2*sin(q3)*sin(q5)*sin(q6)*((641*3^(1/2))/20000 + 37/1000) + dq4*dqr1*cos(q2)*cos(q4)^2*sin(q3)*sin(q5)*sin(q6)*((641*3^(1/2))/20000 + 37/1000) + dq5*dqr1*cos(q2)*cos(q4)^2*sin(q3)*sin(q5)*sin(q6)*((641*3^(1/2))/20000 + 37/1000) + dq6*dqr1*cos(q2)*cos(q4)^2*sin(q3)*sin(q5)*sin(q6)*((641*3^(1/2))/40000 - 37/4000) - dq1*dqr1*cos(q2)^2*cos(q3)*cos(q4)^2*cos(q5)*cos(q6)*sin(q3)*((641*3^(1/2))/20000 - 37/2000) + (37*dq1*dqr1*cos(q3)*cos(q4)*cos(q5)*cos(q6)*sin(q3)*sin(q4)*sin(q5))/1000 - (37*dq4*dqr1*cos(q2)*cos(q4)*cos(q5)*cos(q6)*sin(q3)*sin(q4)*sin(q5))/1000 - (37*dq5*dqr1*cos(q2)*cos(q4)*cos(q5)*cos(q6)*sin(q3)*sin(q4)*sin(q5))/800 - (37*dq6*dqr1*cos(q2)*cos(q4)*cos(q5)*cos(q6)*sin(q3)*sin(q4)*sin(q5))/800 + dq1*dqr1*cos(q2)^2*cos(q3)*cos(q4)^2*sin(q3)*sin(q5)*sin(q6)*((641*3^(1/2))/10000 + 37/500) - dq1*dqr1*cos(q3)*cos(q4)*cos(q5)*sin(q3)*sin(q4)*sin(q6)*((641*3^(1/2))/10000 + 37/500) + dq4*dqr1*cos(q2)*cos(q4)*cos(q5)*sin(q3)*sin(q4)*sin(q6)*((641*3^(1/2))/10000 + 37/500) - dq1*dqr1*cos(q3)*cos(q4)*cos(q6)*sin(q3)*sin(q4)*sin(q5)*((641*3^(1/2))/20000 - 37/2000) + dq4*dqr1*cos(q2)*cos(q4)*cos(q6)*sin(q3)*sin(q4)*sin(q5)*((641*3^(1/2))/20000 - 37/2000) + dq5*dqr1*cos(q2)*cos(q4)*cos(q5)*sin(q3)*sin(q4)*sin(q6)*((641*3^(1/2))/40000 + 37/2000) + dq6*dqr1*cos(q2)*cos(q4)*cos(q6)*sin(q3)*sin(q4)*sin(q5)*((641*3^(1/2))/40000 + 37/2000) + dq5*dqr1*cos(q2)*cos(q4)*cos(q6)*sin(q3)*sin(q4)*sin(q5)*((641*3^(1/2))/80000 - 37/8000) + dq6*dqr1*cos(q2)*cos(q4)*cos(q5)*sin(q3)*sin(q4)*sin(q6)*((641*3^(1/2))/80000 - 37/8000) + (37*3^(1/2)*dq1*dqr1*cos(q2)^2*cos(q3)^2*cos(q5)*sin(q4)*sin(q5)*sin(q6))/500 - (37*dq1*dqr1*cos(q2)^2*cos(q3)*cos(q4)*cos(q5)^2*sin(q3)*sin(q4)*sin(q6))/250 - (37*dq1*dqr1*cos(q2)^2*cos(q3)*cos(q4)^2*cos(q5)*sin(q3)*sin(q5)*sin(q6))/200 - (37*dq1*dqr1*cos(q2)^2*cos(q3)*cos(q4)*cos(q5)*cos(q6)*sin(q3)*sin(q4)*sin(q5))/500 + dq1*dqr1*cos(q2)^2*cos(q3)*cos(q4)*cos(q5)*sin(q3)*sin(q4)*sin(q6)*((641*3^(1/2))/5000 + 37/250) + dq1*dqr1*cos(q2)^2*cos(q3)*cos(q4)*cos(q6)*sin(q3)*sin(q4)*sin(q5)*((641*3^(1/2))/10000 - 37/1000);
Y2_10_3=(37*3^(1/2)*dq1*dqr1*cos(q4)*sin(q6))/2000 - (87*dq1*dqr1*cos(q3)*cos(q6)*sin(q4))/400 - (877*dq1*dqr1*cos(q4)*cos(q5)*sin(q6))/4000 - (1231*dq1*dqr1*cos(q5)*cos(q6)*sin(q4))/40000 + (87*dq4*dqr1*cos(q2)*cos(q6)*sin(q4))/400 + (87*dq6*dqr1*cos(q2)*cos(q4)*sin(q6))/400 + (87*dq6*dqr2*sin(q3)*sin(q4)*sin(q6))/400 - dq1*dqr1*cos(q6)*sin(q4)*((37*3^(1/2))/4000 + 7539/40000) + dq1*dqr1*cos(q2)^2*cos(q6)*sin(q4)*((37*3^(1/2))/2000 + 7539/20000) + dq1*dqr1*cos(q3)^2*cos(q6)*sin(q4)*((37*3^(1/2))/2000 + 7539/20000) - (37*3^(1/2)*dq1*dqr1*cos(q2)^2*cos(q4)*sin(q6))/1000 - (37*3^(1/2)*dq1*dqr1*cos(q3)^2*cos(q4)*sin(q6))/1000 - (37*3^(1/2)*dq1*dqr1*cos(q4)*cos(q5)^2*sin(q6))/1000 - (37*3^(1/2)*dq1*dqr1*cos(q5)^2*cos(q6)*sin(q4))/4000 - (29*dq1*dqr1*cos(q3)*cos(q4)*cos(q5)*sin(q6))/100 - (29*dq1*dqr1*cos(q3)*cos(q4)*cos(q6)*sin(q5))/200 - (29*dq1*dqr1*cos(q3)*cos(q5)*cos(q6)*sin(q4))/400 + (29*dq4*dqr1*cos(q2)*cos(q4)*cos(q5)*sin(q6))/100 + (29*dq4*dqr1*cos(q2)*cos(q4)*cos(q6)*sin(q5))/200 + (29*dq4*dqr1*cos(q2)*cos(q5)*cos(q6)*sin(q4))/400 - (2631*dq6*dqr1*cos(q2)*cos(q3)*cos(q4)*sin(q6))/16000 + (29*dq5*dqr1*cos(q2)*cos(q4)*cos(q5)*sin(q6))/200 + (29*dq5*dqr1*cos(q2)*cos(q4)*cos(q6)*sin(q5))/400 + (29*dq5*dqr1*cos(q2)*cos(q5)*cos(q6)*sin(q4))/200 + (29*dq6*dqr1*cos(q2)*cos(q4)*cos(q5)*sin(q6))/400 + (29*dq6*dqr1*cos(q2)*cos(q4)*cos(q6)*sin(q5))/200 + (29*dq6*dqr1*cos(q2)*cos(q5)*cos(q6)*sin(q4))/100 + (29*dq1*dqr1*cos(q3)*sin(q4)*sin(q5)*sin(q6))/200 - (29*dq4*dqr1*cos(q2)*sin(q4)*sin(q5)*sin(q6))/200 - (29*dq5*dqr1*cos(q2)*sin(q4)*sin(q5)*sin(q6))/100 + (29*dq4*dqr2*cos(q4)*sin(q3)*sin(q5)*sin(q6))/200 + (29*dq4*dqr2*cos(q5)*sin(q3)*sin(q4)*sin(q6))/100 + (29*dq4*dqr2*cos(q6)*sin(q3)*sin(q4)*sin(q5))/200 - (29*dq6*dqr1*cos(q2)*sin(q4)*sin(q5)*sin(q6))/200 + (29*dq5*dqr2*cos(q4)*sin(q3)*sin(q5)*sin(q6))/100 + (29*dq5*dqr2*cos(q5)*sin(q3)*sin(q4)*sin(q6))/200 + (29*dq5*dqr2*cos(q6)*sin(q3)*sin(q4)*sin(q5))/400 + (29*dq6*dqr2*cos(q4)*sin(q3)*sin(q5)*sin(q6))/200 + (29*dq6*dqr2*cos(q5)*sin(q3)*sin(q4)*sin(q6))/400 + (29*dq6*dqr2*cos(q6)*sin(q3)*sin(q4)*sin(q5))/200 + dq1*dqr1*cos(q4)*cos(q6)*sin(q5)*((37*3^(1/2))/4000 - 877/8000) + (87*dq1*dqr1*cos(q2)^2*cos(q3)*cos(q6)*sin(q4))/200 + (877*dq1*dqr1*cos(q2)^2*cos(q4)*cos(q5)*sin(q6))/2000 + (1231*dq1*dqr1*cos(q2)^2*cos(q5)*cos(q6)*sin(q4))/20000 + (877*dq1*dqr1*cos(q3)^2*cos(q4)*cos(q5)*sin(q6))/2000 + (1231*dq1*dqr1*cos(q3)^2*cos(q5)*cos(q6)*sin(q4))/20000 - dq1*dqr1*sin(q4)*sin(q5)*sin(q6)*((37*3^(1/2))/2000 - 1231/20000) - dq1*dqr1*cos(q2)^2*cos(q4)*cos(q6)*sin(q5)*((37*3^(1/2))/2000 - 877/4000) - dq1*dqr1*cos(q3)^2*cos(q4)*cos(q6)*sin(q5)*((37*3^(1/2))/2000 - 877/4000) + (37*3^(1/2)*dq1*dqr1*cos(q5)*sin(q4)*sin(q5)*sin(q6))/2000 - (877*dq1*dqr1*cos(q2)^2*cos(q3)^2*cos(q4)*cos(q5)*sin(q6))/1000 - (1231*dq1*dqr1*cos(q2)^2*cos(q3)^2*cos(q5)*cos(q6)*sin(q4))/10000 + dq1*dqr1*cos(q2)^2*sin(q4)*sin(q5)*sin(q6)*((37*3^(1/2))/1000 - 1231/10000) + dq1*dqr1*cos(q3)^2*sin(q4)*sin(q5)*sin(q6)*((37*3^(1/2))/1000 - 1231/10000) - (877*dq4*dqr1*cos(q2)*cos(q3)*cos(q4)*cos(q5)*sin(q6))/4000 - (1231*dq4*dqr1*cos(q2)*cos(q3)*cos(q5)*cos(q6)*sin(q4))/40000 - (877*dq5*dqr1*cos(q2)*cos(q3)*cos(q4)*cos(q5)*sin(q6))/8000 - (877*dq6*dqr1*cos(q2)*cos(q3)*cos(q4)*cos(q6)*sin(q5))/8000 - (877*dq6*dqr1*cos(q2)*cos(q3)*cos(q5)*cos(q6)*sin(q4))/4000 - dq1*dqr1*cos(q2)^2*cos(q3)^2*cos(q6)*sin(q4)*((37*3^(1/2))/1000 + 7539/10000) + (877*dq5*dqr1*cos(q2)*cos(q3)*sin(q4)*sin(q5)*sin(q6))/4000 + (877*dq6*dqr1*cos(q2)*cos(q3)*sin(q4)*sin(q5)*sin(q6))/8000 - dq4*dqr1*cos(q2)*cos(q3)*cos(q6)*sin(q4)*((37*3^(1/2))/4000 + 7539/40000) + (37*3^(1/2)*dq1*dqr1*cos(q2)^2*cos(q3)^2*cos(q4)*sin(q6))/500 + (37*3^(1/2)*dq1*dqr1*cos(q2)^2*cos(q4)*cos(q5)^2*sin(q6))/500 + (37*3^(1/2)*dq1*dqr1*cos(q2)^2*cos(q5)^2*cos(q6)*sin(q4))/2000 + (37*3^(1/2)*dq1*dqr1*cos(q3)^2*cos(q4)*cos(q5)^2*sin(q6))/500 + (37*3^(1/2)*dq1*dqr1*cos(q3)^2*cos(q5)^2*cos(q6)*sin(q4))/2000 + (29*dq1*dqr1*cos(q2)^2*cos(q3)*cos(q4)*cos(q5)*sin(q6))/50 + (29*dq1*dqr1*cos(q2)^2*cos(q3)*cos(q4)*cos(q6)*sin(q5))/100 + (29*dq1*dqr1*cos(q2)^2*cos(q3)*cos(q5)*cos(q6)*sin(q4))/200 - (29*dq1*dqr1*cos(q2)^2*cos(q3)*sin(q4)*sin(q5)*sin(q6))/100 + (37*3^(1/2)*dq4*dqr1*cos(q2)*cos(q3)*cos(q4)*sin(q6))/2000 + (37*3^(1/2)*dq5*dqr1*cos(q2)*cos(q3)*cos(q4)*sin(q6))/4000 - (37*3^(1/2)*dq1*dqr1*cos(q4)*cos(q5)*cos(q6)*sin(q5))/2000 + (37*3^(1/2)*dq1*dqr1*cos(q2)^2*cos(q4)*cos(q5)*cos(q6)*sin(q5))/1000 + (37*3^(1/2)*dq1*dqr1*cos(q3)^2*cos(q4)*cos(q5)*cos(q6)*sin(q5))/1000 - (37*3^(1/2)*dq4*dqr1*cos(q2)*cos(q3)*cos(q4)*cos(q5)^2*sin(q6))/1000 - (37*3^(1/2)*dq4*dqr1*cos(q2)*cos(q3)*cos(q5)^2*cos(q6)*sin(q4))/4000 - (37*3^(1/2)*dq5*dqr1*cos(q2)*cos(q3)*cos(q4)*cos(q5)^2*sin(q6))/2000 - (37*3^(1/2)*dq5*dqr1*cos(q2)*cos(q3)*cos(q5)^2*cos(q6)*sin(q4))/2000 - (37*3^(1/2)*dq6*dqr1*cos(q2)*cos(q3)*cos(q4)*cos(q5)^2*sin(q6))/8000 - (37*3^(1/2)*dq6*dqr1*cos(q2)*cos(q3)*cos(q5)^2*cos(q6)*sin(q4))/2000 + dq1*dqr1*cos(q2)^2*cos(q3)^2*cos(q4)*cos(q6)*sin(q5)*((37*3^(1/2))/1000 - 877/2000) - (37*3^(1/2)*dq1*dqr1*cos(q2)^2*cos(q5)*sin(q4)*sin(q5)*sin(q6))/1000 - (37*3^(1/2)*dq1*dqr1*cos(q3)^2*cos(q5)*sin(q4)*sin(q5)*sin(q6))/1000 + dq4*dqr1*cos(q2)*cos(q3)*cos(q4)*cos(q6)*sin(q5)*((37*3^(1/2))/4000 - 877/8000) + dq5*dqr1*cos(q2)*cos(q3)*cos(q5)*cos(q6)*sin(q4)*((37*3^(1/2))/4000 - 877/8000) + dq5*dqr1*cos(q2)*cos(q3)*cos(q4)*cos(q6)*sin(q5)*((37*3^(1/2))/8000 - 877/16000) - dq6*dqr1*cos(q2)*cos(q3)*cos(q4)*cos(q5)*sin(q6)*((111*3^(1/2))/8000 + 877/16000) - dq4*dqr1*cos(q2)*cos(q3)*sin(q4)*sin(q5)*sin(q6)*((37*3^(1/2))/2000 - 1231/20000) - (37*3^(1/2)*dq1*dqr1*cos(q2)^2*cos(q3)^2*cos(q4)*cos(q5)^2*sin(q6))/250 - (37*3^(1/2)*dq1*dqr1*cos(q2)^2*cos(q3)^2*cos(q5)^2*cos(q6)*sin(q4))/1000 - (37*3^(1/2)*dq1*dqr1*cos(q2)^2*cos(q3)^2*cos(q4)*cos(q5)*cos(q6)*sin(q5))/500 - (37*3^(1/2)*dq4*dqr1*cos(q2)*cos(q3)*cos(q4)*cos(q5)*cos(q6)*sin(q5))/2000 - (37*3^(1/2)*dq5*dqr1*cos(q2)*cos(q3)*cos(q4)*cos(q5)*cos(q6)*sin(q5))/4000 - (37*3^(1/2)*dq6*dqr1*cos(q2)*cos(q3)*cos(q4)*cos(q5)*cos(q6)*sin(q5))/4000 + (37*3^(1/2)*dq4*dqr1*cos(q2)*cos(q3)*cos(q5)*sin(q4)*sin(q5)*sin(q6))/2000 + (37*3^(1/2)*dq5*dqr1*cos(q2)*cos(q3)*cos(q5)*sin(q4)*sin(q5)*sin(q6))/1000 + (37*3^(1/2)*dq6*dqr1*cos(q2)*cos(q3)*cos(q5)*sin(q4)*sin(q5)*sin(q6))/4000;
Y2_10_4=(37*dq4*dqr2*sin(q6))/2000 + (37*dq5*dqr2*sin(q6))/1000 + dq6*dqr2*sin(q6)*((1577*3^(1/2))/20000 + 111/4000) - (37*dq4*dqr2*cos(q4)^2*sin(q6))/1000 - (37*dq4*dqr2*cos(q5)^2*sin(q6))/1000 - (37*dq5*dqr2*cos(q4)^2*sin(q6))/800 - (37*dq5*dqr2*cos(q5)^2*sin(q6))/500 - (37*dq6*dqr2*cos(q5)^2*sin(q6))/2000 - (29*3^(1/2)*dq2*dqr3*cos(q6)*sin(q3))/400 - (29*3^(1/2)*dq3*dqr2*cos(q6)*sin(q3))/400 + (29*3^(1/2)*dq3*dqr3*cos(q6)*sin(q3))/400 - (29*3^(1/2)*dq6*dqr2*cos(q3)*sin(q6))/400 - dq6*dqr2*cos(q4)^2*sin(q6)*((1923*3^(1/2))/80000 + 37/800) + (37*dq4*dqr2*cos(q4)^2*cos(q5)^2*sin(q6))/500 + (37*dq5*dqr2*cos(q4)^2*cos(q5)^2*sin(q6))/400 + (37*dq6*dqr2*cos(q4)^2*cos(q5)^2*sin(q6))/1600 - (87*dq2*dqr3*cos(q3)*cos(q6)*sin(q4))/400 - (87*dq3*dqr2*cos(q3)*cos(q6)*sin(q4))/400 + (87*dq3*dqr3*cos(q3)*cos(q6)*sin(q4))/400 - (87*dq4*dqr2*cos(q4)*cos(q6)*sin(q3))/400 + (87*dq4*dqr3*cos(q4)*cos(q6)*sin(q3))/400 - (37*dq5*dqr2*cos(q4)*cos(q6)*sin(q4))/2000 - (37*dq4*dqr2*cos(q5)*cos(q6)*sin(q5))/2000 - (37*dq6*dqr2*cos(q4)*cos(q6)*sin(q4))/2000 - (37*dq5*dqr2*cos(q5)*cos(q6)*sin(q5))/1000 - (37*dq6*dqr2*cos(q5)*cos(q6)*sin(q5))/1000 - (87*dq6*dqr3*sin(q3)*sin(q4)*sin(q6))/400 - dq5*dqr2*cos(q5)*sin(q6)*((117*3^(1/2))/1250 - 37/2000) - dq6*dqr2*cos(q6)*sin(q5)*((117*3^(1/2))/1250 - 37/2000) - dq5*dqr2*cos(q6)*sin(q5)*((117*3^(1/2))/2500 - 37/4000) - dq6*dqr2*cos(q5)*sin(q6)*((117*3^(1/2))/2500 - 37/4000) + dq4*dqr2*cos(q5)*sin(q6)*((641*3^(1/2))/20000 + 37/1000) + dq4*dqr2*cos(q6)*sin(q5)*((641*3^(1/2))/40000 - 37/4000) + (29*3^(1/2)*dq2*dqr3*cos(q5)*cos(q6)*sin(q3))/400 + (29*3^(1/2)*dq3*dqr2*cos(q5)*cos(q6)*sin(q3))/400 - (29*3^(1/2)*dq3*dqr3*cos(q5)*cos(q6)*sin(q3))/400 + (29*3^(1/2)*dq5*dqr2*cos(q3)*cos(q5)*sin(q6))/200 + (29*3^(1/2)*dq5*dqr2*cos(q3)*cos(q6)*sin(q5))/400 + (29*3^(1/2)*dq6*dqr2*cos(q3)*cos(q5)*sin(q6))/400 + (29*3^(1/2)*dq6*dqr2*cos(q3)*cos(q6)*sin(q5))/200 - dq4*dqr2*cos(q4)^2*cos(q5)*sin(q6)*((641*3^(1/2))/10000 + 37/500) - dq4*dqr2*cos(q4)^2*cos(q6)*sin(q5)*((641*3^(1/2))/20000 - 37/2000) - dq5*dqr2*cos(q4)^2*cos(q5)*sin(q6)*((641*3^(1/2))/40000 + 37/2000) - dq6*dqr2*cos(q4)^2*cos(q6)*sin(q5)*((641*3^(1/2))/40000 + 37/2000) - dq5*dqr2*cos(q4)^2*cos(q6)*sin(q5)*((641*3^(1/2))/80000 - 37/8000) - dq6*dqr2*cos(q4)^2*cos(q5)*sin(q6)*((641*3^(1/2))/80000 - 37/8000) - (29*3^(1/2)*dq2*dqr3*sin(q3)*sin(q5)*sin(q6))/200 - (29*3^(1/2)*dq3*dqr2*sin(q3)*sin(q5)*sin(q6))/200 + (29*3^(1/2)*dq3*dqr3*sin(q3)*sin(q5)*sin(q6))/200 - (29*dq2*dqr3*cos(q3)*cos(q5)*cos(q6)*sin(q4))/400 - (29*dq3*dqr2*cos(q3)*cos(q4)*cos(q5)*sin(q6))/100 - (29*dq3*dqr2*cos(q3)*cos(q4)*cos(q6)*sin(q5))/200 - (29*dq3*dqr2*cos(q3)*cos(q5)*cos(q6)*sin(q4))/400 + (29*dq3*dqr3*cos(q3)*cos(q5)*cos(q6)*sin(q4))/400 - (29*dq4*dqr2*cos(q4)*cos(q5)*cos(q6)*sin(q3))/400 + (29*dq4*dqr3*cos(q4)*cos(q5)*cos(q6)*sin(q3))/400 - (29*dq5*dqr2*cos(q4)*cos(q5)*cos(q6)*sin(q3))/200 + (29*dq5*dqr3*cos(q4)*cos(q5)*cos(q6)*sin(q3))/200 - (29*dq6*dqr2*cos(q4)*cos(q5)*cos(q6)*sin(q3))/100 + (29*dq6*dqr3*cos(q4)*cos(q5)*cos(q6)*sin(q3))/100 + (29*dq2*dqr3*cos(q3)*sin(q4)*sin(q5)*sin(q6))/200 + (29*dq3*dqr2*cos(q3)*sin(q4)*sin(q5)*sin(q6))/200 - (29*dq3*dqr3*cos(q3)*sin(q4)*sin(q5)*sin(q6))/200 - (29*dq4*dqr3*cos(q4)*sin(q3)*sin(q5)*sin(q6))/200 - (29*dq4*dqr3*cos(q5)*sin(q3)*sin(q4)*sin(q6))/100 - (29*dq4*dqr3*cos(q6)*sin(q3)*sin(q4)*sin(q5))/200 - (29*dq5*dqr3*cos(q4)*sin(q3)*sin(q5)*sin(q6))/100 - (29*dq5*dqr3*cos(q5)*sin(q3)*sin(q4)*sin(q6))/200 - (29*dq5*dqr3*cos(q6)*sin(q3)*sin(q4)*sin(q5))/400 - (29*dq6*dqr3*cos(q4)*sin(q3)*sin(q5)*sin(q6))/200 - (29*dq6*dqr3*cos(q5)*sin(q3)*sin(q4)*sin(q6))/400 - (29*dq6*dqr3*cos(q6)*sin(q3)*sin(q4)*sin(q5))/200 - dq4*dqr2*cos(q4)*cos(q6)*sin(q4)*((1923*3^(1/2))/40000 + 37/400) + (37*dq4*dqr2*cos(q4)*cos(q5)^2*cos(q6)*sin(q4))/800 + (37*dq4*dqr2*cos(q4)^2*cos(q5)*cos(q6)*sin(q5))/1000 - (37*dq4*dqr3*cos(q4)*cos(q5)^2*cos(q6)*sin(q4))/800 + (37*dq5*dqr2*cos(q4)*cos(q5)^2*cos(q6)*sin(q4))/1000 + (37*dq5*dqr2*cos(q4)^2*cos(q5)*cos(q6)*sin(q5))/800 - (37*dq5*dqr3*cos(q4)*cos(q5)^2*cos(q6)*sin(q4))/1000 + (37*dq6*dqr2*cos(q4)*cos(q5)^2*cos(q6)*sin(q4))/1000 + (37*dq6*dqr2*cos(q4)^2*cos(q5)*cos(q6)*sin(q5))/800 - (37*dq6*dqr3*cos(q4)*cos(q5)^2*cos(q6)*sin(q4))/1000 - (37*dq4*dqr2*cos(q4)*cos(q5)*sin(q4)*sin(q5)*sin(q6))/400 + (37*dq4*dqr3*cos(q4)*cos(q5)*sin(q4)*sin(q5)*sin(q6))/400 - (37*dq5*dqr2*cos(q4)*cos(q5)*sin(q4)*sin(q5)*sin(q6))/500 + (37*dq5*dqr3*cos(q4)*cos(q5)*sin(q4)*sin(q5)*sin(q6))/500 - (37*dq6*dqr2*cos(q4)*cos(q5)*sin(q4)*sin(q5)*sin(q6))/2000 + (37*dq6*dqr3*cos(q4)*cos(q5)*sin(q4)*sin(q5)*sin(q6))/2000 - dq6*dqr2*cos(q4)*cos(q5)*cos(q6)*sin(q4)*((641*3^(1/2))/20000 + 37/1000) + dq6*dqr3*cos(q4)*cos(q5)*cos(q6)*sin(q4)*((641*3^(1/2))/20000 + 37/1000) - dq4*dqr2*cos(q4)*cos(q5)*cos(q6)*sin(q4)*((641*3^(1/2))/40000 - 37/4000) + dq4*dqr3*cos(q4)*cos(q5)*cos(q6)*sin(q4)*((641*3^(1/2))/40000 - 37/4000) - dq5*dqr2*cos(q4)*cos(q5)*cos(q6)*sin(q4)*((641*3^(1/2))/40000 - 37/4000) + dq5*dqr3*cos(q4)*cos(q5)*cos(q6)*sin(q4)*((641*3^(1/2))/40000 - 37/4000) + dq4*dqr2*cos(q4)*sin(q4)*sin(q5)*sin(q6)*((641*3^(1/2))/20000 + 37/1000) - dq4*dqr3*cos(q4)*sin(q4)*sin(q5)*sin(q6)*((641*3^(1/2))/20000 + 37/1000) + dq5*dqr2*cos(q4)*sin(q4)*sin(q5)*sin(q6)*((641*3^(1/2))/20000 + 37/1000) - dq5*dqr3*cos(q4)*sin(q4)*sin(q5)*sin(q6)*((641*3^(1/2))/20000 + 37/1000) + dq6*dqr2*cos(q4)*sin(q4)*sin(q5)*sin(q6)*((641*3^(1/2))/40000 - 37/4000) - dq6*dqr3*cos(q4)*sin(q4)*sin(q5)*sin(q6)*((641*3^(1/2))/40000 - 37/4000);
Y2_10_5=(37*dq4*dqr3*cos(q4)^2*sin(q6))/1000 - (37*dq5*dqr3*sin(q6))/1000 - dq6*dqr3*sin(q6)*((1577*3^(1/2))/20000 + 111/4000) - (37*dq4*dqr3*sin(q6))/2000 + (37*dq4*dqr3*cos(q5)^2*sin(q6))/1000 + (37*dq5*dqr3*cos(q4)^2*sin(q6))/800 + (37*dq5*dqr3*cos(q5)^2*sin(q6))/500 + (37*dq6*dqr3*cos(q5)^2*sin(q6))/2000 + (29*3^(1/2)*dq6*dqr3*cos(q3)*sin(q6))/400 + dq6*dqr3*cos(q4)^2*sin(q6)*((1923*3^(1/2))/80000 + 37/800) - (37*dq4*dqr3*cos(q4)^2*cos(q5)^2*sin(q6))/500 - (37*dq5*dqr3*cos(q4)^2*cos(q5)^2*sin(q6))/400 - (37*dq6*dqr3*cos(q4)^2*cos(q5)^2*sin(q6))/1600 - (87*dq2*dqr4*cos(q4)*cos(q6)*sin(q3))/400 + (87*dq3*dqr4*cos(q4)*cos(q6)*sin(q3))/400 + (37*dq5*dqr3*cos(q4)*cos(q6)*sin(q4))/2000 + (37*dq4*dqr3*cos(q5)*cos(q6)*sin(q5))/2000 + (37*dq6*dqr3*cos(q4)*cos(q6)*sin(q4))/2000 + (37*dq5*dqr3*cos(q5)*cos(q6)*sin(q5))/1000 + (37*dq6*dqr3*cos(q5)*cos(q6)*sin(q5))/1000 + dq5*dqr3*cos(q5)*sin(q6)*((117*3^(1/2))/1250 - 37/2000) + dq6*dqr3*cos(q6)*sin(q5)*((117*3^(1/2))/1250 - 37/2000) + dq5*dqr3*cos(q6)*sin(q5)*((117*3^(1/2))/2500 - 37/4000) + dq6*dqr3*cos(q5)*sin(q6)*((117*3^(1/2))/2500 - 37/4000) - dq4*dqr3*cos(q5)*sin(q6)*((641*3^(1/2))/20000 + 37/1000) - dq4*dqr3*cos(q6)*sin(q5)*((641*3^(1/2))/40000 - 37/4000) - (29*3^(1/2)*dq5*dqr3*cos(q3)*cos(q5)*sin(q6))/200 - (29*3^(1/2)*dq5*dqr3*cos(q3)*cos(q6)*sin(q5))/400 - (29*3^(1/2)*dq6*dqr3*cos(q3)*cos(q5)*sin(q6))/400 - (29*3^(1/2)*dq6*dqr3*cos(q3)*cos(q6)*sin(q5))/200 + dq4*dqr3*cos(q4)^2*cos(q5)*sin(q6)*((641*3^(1/2))/10000 + 37/500) + dq4*dqr3*cos(q4)^2*cos(q6)*sin(q5)*((641*3^(1/2))/20000 - 37/2000) + dq5*dqr3*cos(q4)^2*cos(q5)*sin(q6)*((641*3^(1/2))/40000 + 37/2000) + dq6*dqr3*cos(q4)^2*cos(q6)*sin(q5)*((641*3^(1/2))/40000 + 37/2000) + dq5*dqr3*cos(q4)^2*cos(q6)*sin(q5)*((641*3^(1/2))/80000 - 37/8000) + dq6*dqr3*cos(q4)^2*cos(q5)*sin(q6)*((641*3^(1/2))/80000 - 37/8000) - (29*dq2*dqr3*cos(q3)*cos(q4)*cos(q5)*sin(q6))/100 - (29*dq2*dqr3*cos(q3)*cos(q4)*cos(q6)*sin(q5))/200 - (29*dq2*dqr4*cos(q4)*cos(q5)*cos(q6)*sin(q3))/400 + (29*dq3*dqr3*cos(q3)*cos(q4)*cos(q5)*sin(q6))/100 + (29*dq3*dqr3*cos(q3)*cos(q4)*cos(q6)*sin(q5))/200 + (29*dq3*dqr4*cos(q4)*cos(q5)*cos(q6)*sin(q3))/400 - (29*dq1*dqr4*cos(q2)*sin(q4)*sin(q5)*sin(q6))/200 + (29*dq2*dqr4*cos(q4)*sin(q3)*sin(q5)*sin(q6))/200 + (29*dq2*dqr4*cos(q5)*sin(q3)*sin(q4)*sin(q6))/100 + (29*dq2*dqr4*cos(q6)*sin(q3)*sin(q4)*sin(q5))/200 - (29*dq3*dqr4*cos(q4)*sin(q3)*sin(q5)*sin(q6))/200 - (29*dq3*dqr4*cos(q5)*sin(q3)*sin(q4)*sin(q6))/100 - (29*dq3*dqr4*cos(q6)*sin(q3)*sin(q4)*sin(q5))/200 - (29*dq4*dqr4*cos(q3)*sin(q4)*sin(q5)*sin(q6))/200 - (29*dq5*dqr4*cos(q3)*sin(q4)*sin(q5)*sin(q6))/100 - (29*dq6*dqr4*cos(q3)*sin(q4)*sin(q5)*sin(q6))/200 + dq4*dqr3*cos(q4)*cos(q6)*sin(q4)*((1923*3^(1/2))/40000 + 37/400) + dq1*dqr4*cos(q2)*cos(q6)*sin(q3)*((1923*3^(1/2))/40000 + 111/2000) - dq1*dqr4*cos(q3)*cos(q6)*sin(q2)*((1923*3^(1/2))/40000 + 111/2000) - (37*dq1*dqr4*cos(q2)*cos(q5)^2*cos(q6)*sin(q3))/4000 + (37*dq1*dqr4*cos(q3)*cos(q5)^2*cos(q6)*sin(q2))/4000 - (37*dq4*dqr3*cos(q4)^2*cos(q5)*cos(q6)*sin(q5))/1000 - (37*dq5*dqr3*cos(q4)^2*cos(q5)*cos(q6)*sin(q5))/800 - (37*dq6*dqr3*cos(q4)^2*cos(q5)*cos(q6)*sin(q5))/800 - dq1*dqr4*cos(q2)*cos(q4)^2*cos(q6)*sin(q3)*((1923*3^(1/2))/40000 + 37/400) + dq1*dqr4*cos(q3)*cos(q4)^2*cos(q6)*sin(q2)*((1923*3^(1/2))/40000 + 37/400) + (37*3^(1/2)*dq1*dqr4*cos(q4)*sin(q2)*sin(q3)*sin(q6))/2000 + (37*dq1*dqr4*cos(q2)*cos(q4)^2*cos(q5)^2*cos(q6)*sin(q3))/800 - (37*dq1*dqr4*cos(q3)*cos(q4)^2*cos(q5)^2*cos(q6)*sin(q2))/800 + (37*dq1*dqr4*cos(q2)*cos(q4)*sin(q3)*sin(q4)*sin(q6))/1000 - (37*dq1*dqr4*cos(q3)*cos(q4)*sin(q2)*sin(q4)*sin(q6))/1000 - (877*dq1*dqr4*cos(q4)*cos(q5)*sin(q2)*sin(q3)*sin(q6))/4000 - (1231*dq1*dqr4*cos(q5)*cos(q6)*sin(q2)*sin(q3)*sin(q4))/40000 + (37*dq1*dqr4*cos(q2)*cos(q5)*sin(q3)*sin(q5)*sin(q6))/2000 - (37*dq1*dqr4*cos(q3)*cos(q5)*sin(q2)*sin(q5)*sin(q6))/2000 - (37*dq2*dqr4*cos(q4)*cos(q5)*sin(q4)*sin(q5)*sin(q6))/400 + (37*dq3*dqr4*cos(q4)*cos(q5)*sin(q4)*sin(q5)*sin(q6))/400 + dq1*dqr4*cos(q2)*cos(q5)*cos(q6)*sin(q3)*((641*3^(1/2))/40000 - 37/4000) - dq1*dqr4*cos(q3)*cos(q5)*cos(q6)*sin(q2)*((641*3^(1/2))/40000 - 37/4000) - dq1*dqr4*cos(q2)*sin(q3)*sin(q5)*sin(q6)*((641*3^(1/2))/20000 + 37/1000) + dq1*dqr4*cos(q3)*sin(q2)*sin(q5)*sin(q6)*((641*3^(1/2))/20000 + 37/1000) - dq1*dqr4*cos(q6)*sin(q2)*sin(q3)*sin(q4)*((37*3^(1/2))/4000 + 7539/40000) - (37*3^(1/2)*dq1*dqr4*cos(q4)*cos(q5)^2*sin(q2)*sin(q3)*sin(q6))/1000 - (37*3^(1/2)*dq1*dqr4*cos(q5)^2*cos(q6)*sin(q2)*sin(q3)*sin(q4))/4000 + dq1*dqr4*cos(q4)*cos(q6)*sin(q2)*sin(q3)*sin(q5)*((37*3^(1/2))/4000 - 877/8000) - dq1*dqr4*cos(q2)*cos(q3)*sin(q4)*sin(q5)*sin(q6)*((37*3^(1/2))/2000 - 1231/20000) - (37*dq1*dqr4*cos(q2)*cos(q4)*cos(q5)^2*sin(q3)*sin(q4)*sin(q6))/500 + (37*dq1*dqr4*cos(q3)*cos(q4)*cos(q5)^2*sin(q2)*sin(q4)*sin(q6))/500 - (37*dq1*dqr4*cos(q2)*cos(q4)^2*cos(q5)*sin(q3)*sin(q5)*sin(q6))/400 + (37*dq1*dqr4*cos(q3)*cos(q4)^2*cos(q5)*sin(q2)*sin(q5)*sin(q6))/400 - dq1*dqr4*sin(q2)*sin(q3)*sin(q4)*sin(q5)*sin(q6)*((37*3^(1/2))/2000 - 1231/20000) - dq1*dqr4*cos(q2)*cos(q4)^2*cos(q5)*cos(q6)*sin(q3)*((641*3^(1/2))/40000 - 37/4000) + dq1*dqr4*cos(q3)*cos(q4)^2*cos(q5)*cos(q6)*sin(q2)*((641*3^(1/2))/40000 - 37/4000) + dq1*dqr4*cos(q2)*cos(q4)^2*sin(q3)*sin(q5)*sin(q6)*((641*3^(1/2))/20000 + 37/1000) - dq1*dqr4*cos(q3)*cos(q4)^2*sin(q2)*sin(q5)*sin(q6)*((641*3^(1/2))/20000 + 37/1000) - (37*dq1*dqr4*cos(q2)*cos(q4)*cos(q5)*cos(q6)*sin(q3)*sin(q4)*sin(q5))/1000 + (37*dq1*dqr4*cos(q3)*cos(q4)*cos(q5)*cos(q6)*sin(q2)*sin(q4)*sin(q5))/1000 + dq1*dqr4*cos(q2)*cos(q4)*cos(q5)*sin(q3)*sin(q4)*sin(q6)*((641*3^(1/2))/10000 + 37/500) - dq1*dqr4*cos(q3)*cos(q4)*cos(q5)*sin(q2)*sin(q4)*sin(q6)*((641*3^(1/2))/10000 + 37/500) + dq1*dqr4*cos(q2)*cos(q4)*cos(q6)*sin(q3)*sin(q4)*sin(q5)*((641*3^(1/2))/20000 - 37/2000) - dq1*dqr4*cos(q3)*cos(q4)*cos(q6)*sin(q2)*sin(q4)*sin(q5)*((641*3^(1/2))/20000 - 37/2000) + (37*3^(1/2)*dq1*dqr4*cos(q2)*cos(q3)*cos(q5)*sin(q4)*sin(q5)*sin(q6))/2000 - (37*3^(1/2)*dq1*dqr4*cos(q4)*cos(q5)*cos(q6)*sin(q2)*sin(q3)*sin(q5))/2000 + (37*3^(1/2)*dq1*dqr4*cos(q5)*sin(q2)*sin(q3)*sin(q4)*sin(q5)*sin(q6))/2000;
Y2_10_6=(37*dq2*dqr4*sin(q6))/2000 - (37*dq3*dqr4*sin(q6))/2000 - (37*dq2*dqr4*cos(q4)^2*sin(q6))/1000 - (37*dq2*dqr4*cos(q5)^2*sin(q6))/1000 + (37*dq3*dqr4*cos(q4)^2*sin(q6))/1000 + (37*dq3*dqr4*cos(q5)^2*sin(q6))/1000 - (2631*dq6*dqr4*cos(q4)*sin(q6))/16000 + (37*3^(1/2)*dq4*dqr4*cos(q4)*sin(q6))/2000 + (37*3^(1/2)*dq5*dqr4*cos(q4)*sin(q6))/4000 + (37*dq2*dqr4*cos(q4)^2*cos(q5)^2*sin(q6))/500 - (37*dq3*dqr4*cos(q4)^2*cos(q5)^2*sin(q6))/500 + (87*dq1*dqr4*cos(q2)*cos(q6)*sin(q4))/400 + (87*dq4*dqr4*cos(q3)*cos(q6)*sin(q4))/400 - (37*dq2*dqr4*cos(q5)*cos(q6)*sin(q5))/2000 + (37*dq3*dqr4*cos(q5)*cos(q6)*sin(q5))/2000 - (877*dq4*dqr4*cos(q4)*cos(q5)*sin(q6))/4000 - (1231*dq4*dqr4*cos(q5)*cos(q6)*sin(q4))/40000 + (87*dq6*dqr4*cos(q3)*cos(q4)*sin(q6))/400 - (877*dq5*dqr4*cos(q4)*cos(q5)*sin(q6))/8000 - (877*dq6*dqr4*cos(q4)*cos(q6)*sin(q5))/8000 - (877*dq6*dqr4*cos(q5)*cos(q6)*sin(q4))/4000 + (877*dq5*dqr4*sin(q4)*sin(q5)*sin(q6))/4000 + (877*dq6*dqr4*sin(q4)*sin(q5)*sin(q6))/8000 + dq2*dqr4*cos(q5)*sin(q6)*((641*3^(1/2))/20000 + 37/1000) - dq3*dqr4*cos(q5)*sin(q6)*((641*3^(1/2))/20000 + 37/1000) + dq2*dqr4*cos(q6)*sin(q5)*((641*3^(1/2))/40000 - 37/4000) - dq3*dqr4*cos(q6)*sin(q5)*((641*3^(1/2))/40000 - 37/4000) - dq4*dqr4*cos(q6)*sin(q4)*((37*3^(1/2))/4000 + 7539/40000) - dq2*dqr4*cos(q4)^2*cos(q5)*sin(q6)*((641*3^(1/2))/10000 + 37/500) + dq3*dqr4*cos(q4)^2*cos(q5)*sin(q6)*((641*3^(1/2))/10000 + 37/500) - dq2*dqr4*cos(q4)^2*cos(q6)*sin(q5)*((641*3^(1/2))/20000 - 37/2000) + dq3*dqr4*cos(q4)^2*cos(q6)*sin(q5)*((641*3^(1/2))/20000 - 37/2000) - (37*3^(1/2)*dq4*dqr4*cos(q4)*cos(q5)^2*sin(q6))/1000 - (37*3^(1/2)*dq4*dqr4*cos(q5)^2*cos(q6)*sin(q4))/4000 - (37*3^(1/2)*dq5*dqr4*cos(q4)*cos(q5)^2*sin(q6))/2000 - (37*3^(1/2)*dq5*dqr4*cos(q5)^2*cos(q6)*sin(q4))/2000 - (37*3^(1/2)*dq6*dqr4*cos(q4)*cos(q5)^2*sin(q6))/8000 - (37*3^(1/2)*dq6*dqr4*cos(q5)^2*cos(q6)*sin(q4))/2000 + (29*dq1*dqr4*cos(q2)*cos(q4)*cos(q5)*sin(q6))/100 + (29*dq1*dqr4*cos(q2)*cos(q4)*cos(q6)*sin(q5))/200 + (29*dq1*dqr4*cos(q2)*cos(q5)*cos(q6)*sin(q4))/400 + (29*dq4*dqr4*cos(q3)*cos(q4)*cos(q5)*sin(q6))/100 + (29*dq4*dqr4*cos(q3)*cos(q4)*cos(q6)*sin(q5))/200 + (29*dq4*dqr4*cos(q3)*cos(q5)*cos(q6)*sin(q4))/400 + (29*dq5*dqr4*cos(q3)*cos(q4)*cos(q5)*sin(q6))/200 + (29*dq5*dqr4*cos(q3)*cos(q4)*cos(q6)*sin(q5))/400 + (29*dq5*dqr4*cos(q3)*cos(q5)*cos(q6)*sin(q4))/200 + (29*dq6*dqr4*cos(q3)*cos(q4)*cos(q5)*sin(q6))/400 + (29*dq6*dqr4*cos(q3)*cos(q4)*cos(q6)*sin(q5))/200 + (29*dq6*dqr4*cos(q3)*cos(q5)*cos(q6)*sin(q4))/100 + dq4*dqr4*cos(q4)*cos(q6)*sin(q5)*((37*3^(1/2))/4000 - 877/8000) + dq5*dqr4*cos(q5)*cos(q6)*sin(q4)*((37*3^(1/2))/4000 - 877/8000) + dq5*dqr4*cos(q4)*cos(q6)*sin(q5)*((37*3^(1/2))/8000 - 877/16000) - dq6*dqr4*cos(q4)*cos(q5)*sin(q6)*((111*3^(1/2))/8000 + 877/16000) - dq2*dqr4*cos(q4)*cos(q6)*sin(q4)*((1923*3^(1/2))/40000 + 37/400) + dq3*dqr4*cos(q4)*cos(q6)*sin(q4)*((1923*3^(1/2))/40000 + 37/400) + (37*dq1*dqr5*cos(q3)*cos(q4)^2*cos(q6)*sin(q2))/2000 + (37*dq2*dqr4*cos(q4)*cos(q5)^2*cos(q6)*sin(q4))/800 + (37*dq2*dqr4*cos(q4)^2*cos(q5)*cos(q6)*sin(q5))/1000 - (37*dq3*dqr4*cos(q4)*cos(q5)^2*cos(q6)*sin(q4))/800 - (37*dq3*dqr4*cos(q4)^2*cos(q5)*cos(q6)*sin(q5))/1000 - dq4*dqr4*sin(q4)*sin(q5)*sin(q6)*((37*3^(1/2))/2000 - 1231/20000) + (37*3^(1/2)*dq1*dqr5*cos(q4)*sin(q2)*sin(q3)*sin(q6))/4000 + (37*3^(1/2)*dq4*dqr4*cos(q5)*sin(q4)*sin(q5)*sin(q6))/2000 + (37*3^(1/2)*dq5*dqr4*cos(q5)*sin(q4)*sin(q5)*sin(q6))/1000 + (37*3^(1/2)*dq6*dqr4*cos(q5)*sin(q4)*sin(q5)*sin(q6))/4000 - (37*dq1*dqr5*cos(q3)*cos(q4)^2*cos(q5)^2*cos(q6)*sin(q2))/1000 - (877*dq1*dqr4*cos(q2)*cos(q3)*cos(q4)*cos(q5)*sin(q6))/4000 - (1231*dq1*dqr4*cos(q2)*cos(q3)*cos(q5)*cos(q6)*sin(q4))/40000 - (37*dq1*dqr5*cos(q3)*cos(q4)*sin(q2)*sin(q4)*sin(q6))/800 - (877*dq1*dqr5*cos(q4)*cos(q5)*sin(q2)*sin(q3)*sin(q6))/8000 - (37*dq1*dqr5*cos(q3)*cos(q5)*sin(q2)*sin(q5)*sin(q6))/1000 + (877*dq1*dqr5*sin(q2)*sin(q3)*sin(q4)*sin(q5)*sin(q6))/4000 - dq2*dqr4*cos(q4)*cos(q5)*cos(q6)*sin(q4)*((641*3^(1/2))/40000 - 37/4000) + dq3*dqr4*cos(q4)*cos(q5)*cos(q6)*sin(q4)*((641*3^(1/2))/40000 - 37/4000) - dq1*dqr4*cos(q2)*cos(q3)*cos(q6)*sin(q4)*((37*3^(1/2))/4000 + 7539/40000) + dq1*dqr5*cos(q3)*sin(q2)*sin(q5)*sin(q6)*((641*3^(1/2))/20000 + 37/1000) + dq2*dqr4*cos(q4)*sin(q4)*sin(q5)*sin(q6)*((641*3^(1/2))/20000 + 37/1000) - dq3*dqr4*cos(q4)*sin(q4)*sin(q5)*sin(q6)*((641*3^(1/2))/20000 + 37/1000) + (37*3^(1/2)*dq1*dqr4*cos(q2)*cos(q3)*cos(q4)*sin(q6))/2000 - (37*3^(1/2)*dq4*dqr4*cos(q4)*cos(q5)*cos(q6)*sin(q5))/2000 - (37*3^(1/2)*dq5*dqr4*cos(q4)*cos(q5)*cos(q6)*sin(q5))/4000 - (37*3^(1/2)*dq6*dqr4*cos(q4)*cos(q5)*cos(q6)*sin(q5))/4000 - (37*3^(1/2)*dq1*dqr4*cos(q2)*cos(q3)*cos(q4)*cos(q5)^2*sin(q6))/1000 - (37*3^(1/2)*dq1*dqr4*cos(q2)*cos(q3)*cos(q5)^2*cos(q6)*sin(q4))/4000 - (37*3^(1/2)*dq1*dqr5*cos(q4)*cos(q5)^2*sin(q2)*sin(q3)*sin(q6))/2000 - (37*3^(1/2)*dq1*dqr5*cos(q5)^2*cos(q6)*sin(q2)*sin(q3)*sin(q4))/2000 + dq1*dqr4*cos(q2)*cos(q3)*cos(q4)*cos(q6)*sin(q5)*((37*3^(1/2))/4000 - 877/8000) + dq1*dqr5*cos(q5)*cos(q6)*sin(q2)*sin(q3)*sin(q4)*((37*3^(1/2))/4000 - 877/8000) + dq1*dqr5*cos(q4)*cos(q6)*sin(q2)*sin(q3)*sin(q5)*((37*3^(1/2))/8000 - 877/16000) + (37*dq1*dqr5*cos(q3)*cos(q4)*cos(q5)^2*sin(q2)*sin(q4)*sin(q6))/400 + (37*dq1*dqr5*cos(q3)*cos(q4)^2*cos(q5)*sin(q2)*sin(q5)*sin(q6))/500 + dq1*dqr5*cos(q3)*cos(q4)^2*cos(q5)*cos(q6)*sin(q2)*((641*3^(1/2))/40000 - 37/4000) - dq1*dqr5*cos(q3)*cos(q4)^2*sin(q2)*sin(q5)*sin(q6)*((641*3^(1/2))/20000 + 37/1000) + (37*dq1*dqr5*cos(q3)*cos(q4)*cos(q5)*cos(q6)*sin(q2)*sin(q4)*sin(q5))/800 - dq1*dqr5*cos(q3)*cos(q4)*cos(q5)*sin(q2)*sin(q4)*sin(q6)*((641*3^(1/2))/40000 + 37/2000) - dq1*dqr5*cos(q3)*cos(q4)*cos(q6)*sin(q2)*sin(q4)*sin(q5)*((641*3^(1/2))/80000 - 37/8000) - (37*3^(1/2)*dq1*dqr4*cos(q2)*cos(q3)*cos(q4)*cos(q5)*cos(q6)*sin(q5))/2000 - (37*3^(1/2)*dq1*dqr5*cos(q4)*cos(q5)*cos(q6)*sin(q2)*sin(q3)*sin(q5))/4000 + (37*3^(1/2)*dq1*dqr5*cos(q5)*sin(q2)*sin(q3)*sin(q4)*sin(q5)*sin(q6))/1000;
Y2_10_7=(37*dq3*dqr5*cos(q4)^2*sin(q6))/800 - (37*dq2*dqr5*cos(q5)^2*sin(q6))/500 - (37*dq2*dqr5*cos(q4)^2*sin(q6))/800 + (37*3^(1/2)*dq4*dqr5*cos(q4)*sin(q6))/4000 - (37*3^(1/2)*dq6*dqr5*cos(q4)*sin(q6))/4000 + (37*dq2*dqr5*cos(q4)^2*cos(q5)^2*sin(q6))/400 - (37*dq3*dqr5*cos(q4)^2*cos(q5)^2*sin(q6))/400 - (37*dq2*dqr5*cos(q4)*cos(q6)*sin(q4))/2000 + (37*dq3*dqr5*cos(q4)*cos(q6)*sin(q4))/2000 - (37*dq2*dqr5*cos(q5)*cos(q6)*sin(q5))/1000 + (37*dq3*dqr5*cos(q5)*cos(q6)*sin(q5))/1000 - (877*dq4*dqr5*cos(q4)*cos(q5)*sin(q6))/8000 - (877*dq5*dqr5*cos(q4)*cos(q5)*sin(q6))/4000 - (877*dq6*dqr5*cos(q4)*cos(q5)*sin(q6))/8000 - (877*dq6*dqr5*cos(q4)*cos(q6)*sin(q5))/4000 + (877*dq4*dqr5*sin(q4)*sin(q5)*sin(q6))/4000 - dq2*dqr5*cos(q6)*sin(q5)*((117*3^(1/2))/2500 - 37/4000) + dq3*dqr5*cos(q6)*sin(q5)*((117*3^(1/2))/2500 - 37/4000) + (29*3^(1/2)*dq2*dqr5*cos(q3)*cos(q5)*sin(q6))/200 + (29*3^(1/2)*dq2*dqr5*cos(q3)*cos(q6)*sin(q5))/400 - (29*3^(1/2)*dq3*dqr5*cos(q3)*cos(q5)*sin(q6))/200 - (29*3^(1/2)*dq3*dqr5*cos(q3)*cos(q6)*sin(q5))/400 - (29*3^(1/2)*dq5*dqr5*cos(q5)*cos(q6)*sin(q3))/400 - (29*3^(1/2)*dq6*dqr5*cos(q5)*cos(q6)*sin(q3))/200 - dq2*dqr5*cos(q4)^2*cos(q5)*sin(q6)*((641*3^(1/2))/40000 + 37/2000) + dq3*dqr5*cos(q4)^2*cos(q5)*sin(q6)*((641*3^(1/2))/40000 + 37/2000) - dq2*dqr5*cos(q4)^2*cos(q6)*sin(q5)*((641*3^(1/2))/80000 - 37/8000) + dq3*dqr5*cos(q4)^2*cos(q6)*sin(q5)*((641*3^(1/2))/80000 - 37/8000) + (29*3^(1/2)*dq5*dqr5*sin(q3)*sin(q5)*sin(q6))/200 + (29*3^(1/2)*dq6*dqr5*sin(q3)*sin(q5)*sin(q6))/400 - (37*3^(1/2)*dq4*dqr5*cos(q4)*cos(q5)^2*sin(q6))/2000 - (37*3^(1/2)*dq4*dqr5*cos(q5)^2*cos(q6)*sin(q4))/2000 + (29*dq1*dqr5*cos(q2)*cos(q4)*cos(q5)*sin(q6))/200 + (29*dq1*dqr5*cos(q2)*cos(q4)*cos(q6)*sin(q5))/400 + (29*dq1*dqr5*cos(q2)*cos(q5)*cos(q6)*sin(q4))/200 - (29*dq2*dqr5*cos(q4)*cos(q5)*cos(q6)*sin(q3))/200 + (29*dq3*dqr5*cos(q4)*cos(q5)*cos(q6)*sin(q3))/200 + (29*dq4*dqr5*cos(q3)*cos(q4)*cos(q5)*sin(q6))/200 + (29*dq4*dqr5*cos(q3)*cos(q4)*cos(q6)*sin(q5))/400 + (29*dq4*dqr5*cos(q3)*cos(q5)*cos(q6)*sin(q4))/200 + (29*dq5*dqr5*cos(q3)*cos(q4)*cos(q5)*sin(q6))/100 + (29*dq5*dqr5*cos(q3)*cos(q4)*cos(q6)*sin(q5))/200 + (29*dq5*dqr5*cos(q3)*cos(q5)*cos(q6)*sin(q4))/400 + (29*dq6*dqr5*cos(q3)*cos(q4)*cos(q5)*sin(q6))/200 + (29*dq6*dqr5*cos(q3)*cos(q4)*cos(q6)*sin(q5))/100 + (29*dq6*dqr5*cos(q3)*cos(q5)*cos(q6)*sin(q4))/200 - (29*dq1*dqr5*cos(q2)*sin(q4)*sin(q5)*sin(q6))/100 + (29*dq2*dqr5*cos(q4)*sin(q3)*sin(q5)*sin(q6))/100 + (29*dq2*dqr5*cos(q5)*sin(q3)*sin(q4)*sin(q6))/200 + (29*dq2*dqr5*cos(q6)*sin(q3)*sin(q4)*sin(q5))/400 - (29*dq3*dqr5*cos(q4)*sin(q3)*sin(q5)*sin(q6))/100 - (29*dq3*dqr5*cos(q5)*sin(q3)*sin(q4)*sin(q6))/200 - (29*dq3*dqr5*cos(q6)*sin(q3)*sin(q4)*sin(q5))/400 - (29*dq4*dqr5*cos(q3)*sin(q4)*sin(q5)*sin(q6))/100 - (29*dq5*dqr5*cos(q3)*sin(q4)*sin(q5)*sin(q6))/200 - (29*dq6*dqr5*cos(q3)*sin(q4)*sin(q5)*sin(q6))/400 + dq4*dqr5*cos(q5)*cos(q6)*sin(q4)*((37*3^(1/2))/4000 - 877/8000) + dq5*dqr5*cos(q4)*cos(q6)*sin(q5)*((37*3^(1/2))/4000 - 877/8000) - dq6*dqr5*cos(q5)*cos(q6)*sin(q4)*((37*3^(1/2))/2000 + 1577/10000) + dq4*dqr5*cos(q4)*cos(q6)*sin(q5)*((37*3^(1/2))/8000 - 877/16000) + dq5*dqr5*cos(q5)*cos(q6)*sin(q4)*((37*3^(1/2))/4000 - 1577/20000) - (37*dq1*dqr5*cos(q2)*cos(q4)^2*cos(q6)*sin(q3))/2000 - (37*dq1*dqr5*cos(q2)*cos(q5)^2*cos(q6)*sin(q3))/2000 + (37*dq1*dqr5*cos(q3)*cos(q5)^2*cos(q6)*sin(q2))/2000 + (37*dq2*dqr5*cos(q4)*cos(q5)^2*cos(q6)*sin(q4))/1000 + (37*dq2*dqr5*cos(q4)^2*cos(q5)*cos(q6)*sin(q5))/800 - (37*dq3*dqr5*cos(q4)*cos(q5)^2*cos(q6)*sin(q4))/1000 - (37*dq3*dqr5*cos(q4)^2*cos(q5)*cos(q6)*sin(q5))/800 + dq5*dqr5*sin(q4)*sin(q5)*sin(q6)*((37*3^(1/2))/2000 + 1577/10000) + dq6*dqr5*sin(q4)*sin(q5)*sin(q6)*((37*3^(1/2))/4000 + 1577/20000) + (37*3^(1/2)*dq4*dqr5*cos(q5)*sin(q4)*sin(q5)*sin(q6))/1000 + (37*dq1*dqr5*cos(q2)*cos(q4)^2*cos(q5)^2*cos(q6)*sin(q3))/1000 - (877*dq1*dqr5*cos(q2)*cos(q3)*cos(q4)*cos(q5)*sin(q6))/8000 + (37*dq1*dqr5*cos(q2)*cos(q4)*sin(q3)*sin(q4)*sin(q6))/800 + (877*dq1*dqr5*cos(q2)*cos(q3)*sin(q4)*sin(q5)*sin(q6))/4000 + (37*dq1*dqr5*cos(q2)*cos(q5)*sin(q3)*sin(q5)*sin(q6))/1000 - (37*dq2*dqr5*cos(q4)*cos(q5)*sin(q4)*sin(q5)*sin(q6))/500 + (37*dq3*dqr5*cos(q4)*cos(q5)*sin(q4)*sin(q5)*sin(q6))/500 + dq1*dqr5*cos(q2)*cos(q5)*cos(q6)*sin(q3)*((641*3^(1/2))/40000 - 37/4000) - dq1*dqr5*cos(q3)*cos(q5)*cos(q6)*sin(q2)*((641*3^(1/2))/40000 - 37/4000) - dq2*dqr5*cos(q4)*cos(q5)*cos(q6)*sin(q4)*((641*3^(1/2))/40000 - 37/4000) + dq3*dqr5*cos(q4)*cos(q5)*cos(q6)*sin(q4)*((641*3^(1/2))/40000 - 37/4000) - dq1*dqr5*cos(q2)*sin(q3)*sin(q5)*sin(q6)*((641*3^(1/2))/20000 + 37/1000) + dq2*dqr5*cos(q4)*sin(q4)*sin(q5)*sin(q6)*((641*3^(1/2))/20000 + 37/1000) - dq3*dqr5*cos(q4)*sin(q4)*sin(q5)*sin(q6)*((641*3^(1/2))/20000 + 37/1000) + (37*3^(1/2)*dq1*dqr5*cos(q2)*cos(q3)*cos(q4)*sin(q6))/4000 - (37*3^(1/2)*dq4*dqr5*cos(q4)*cos(q5)*cos(q6)*sin(q5))/4000 - (37*3^(1/2)*dq1*dqr5*cos(q2)*cos(q3)*cos(q4)*cos(q5)^2*sin(q6))/2000 - (37*3^(1/2)*dq1*dqr5*cos(q2)*cos(q3)*cos(q5)^2*cos(q6)*sin(q4))/2000 + dq1*dqr5*cos(q2)*cos(q3)*cos(q5)*cos(q6)*sin(q4)*((37*3^(1/2))/4000 - 877/8000) + dq1*dqr5*cos(q2)*cos(q3)*cos(q4)*cos(q6)*sin(q5)*((37*3^(1/2))/8000 - 877/16000) - (37*dq1*dqr5*cos(q2)*cos(q4)*cos(q5)^2*sin(q3)*sin(q4)*sin(q6))/400 - (37*dq1*dqr5*cos(q2)*cos(q4)^2*cos(q5)*sin(q3)*sin(q5)*sin(q6))/500 - dq1*dqr5*cos(q2)*cos(q4)^2*cos(q5)*cos(q6)*sin(q3)*((641*3^(1/2))/40000 - 37/4000) + dq1*dqr5*cos(q2)*cos(q4)^2*sin(q3)*sin(q5)*sin(q6)*((641*3^(1/2))/20000 + 37/1000) - (37*dq1*dqr5*cos(q2)*cos(q4)*cos(q5)*cos(q6)*sin(q3)*sin(q4)*sin(q5))/800 + dq1*dqr5*cos(q2)*cos(q4)*cos(q5)*sin(q3)*sin(q4)*sin(q6)*((641*3^(1/2))/40000 + 37/2000) + dq1*dqr5*cos(q2)*cos(q4)*cos(q6)*sin(q3)*sin(q4)*sin(q5)*((641*3^(1/2))/80000 - 37/8000) - (37*3^(1/2)*dq1*dqr5*cos(q2)*cos(q3)*cos(q4)*cos(q5)*cos(q6)*sin(q5))/4000 + (37*3^(1/2)*dq1*dqr5*cos(q2)*cos(q3)*cos(q5)*sin(q4)*sin(q5)*sin(q6))/1000;
Y2_10_8=(37*dq2*dqr5*sin(q6))/1000 - (37*dq3*dqr5*sin(q6))/1000 + (37*dq3*dqr5*cos(q5)^2*sin(q6))/500 + (29*3^(1/2)*dq6*dqr6*cos(q6)*sin(q3))/400 - (37*dq2*dqr6*cos(q4)*cos(q6)*sin(q4))/2000 + (37*dq3*dqr6*cos(q4)*cos(q6)*sin(q4))/2000 - (877*dq4*dqr6*cos(q5)*cos(q6)*sin(q4))/4000 + (87*dq6*dqr6*cos(q3)*cos(q6)*sin(q4))/400 + (87*dq2*dqr6*sin(q3)*sin(q4)*sin(q6))/400 - (87*dq3*dqr6*sin(q3)*sin(q4)*sin(q6))/400 + (877*dq4*dqr6*sin(q4)*sin(q5)*sin(q6))/8000 - dq2*dqr5*cos(q5)*sin(q6)*((117*3^(1/2))/1250 - 37/2000) + dq3*dqr5*cos(q5)*sin(q6)*((117*3^(1/2))/1250 - 37/2000) + dq6*dqr6*cos(q6)*sin(q4)*((37*3^(1/2))/4000 - 351/2500) + (29*3^(1/2)*dq2*dqr6*cos(q3)*cos(q6)*sin(q5))/200 - (29*3^(1/2)*dq3*dqr6*cos(q3)*cos(q6)*sin(q5))/200 - (29*3^(1/2)*dq5*dqr6*cos(q5)*cos(q6)*sin(q3))/200 - (29*3^(1/2)*dq6*dqr6*cos(q5)*cos(q6)*sin(q3))/400 - dq2*dqr6*cos(q4)^2*cos(q6)*sin(q5)*((641*3^(1/2))/40000 + 37/2000) + (29*3^(1/2)*dq5*dqr6*sin(q3)*sin(q5)*sin(q6))/400 + (29*3^(1/2)*dq6*dqr6*sin(q3)*sin(q5)*sin(q6))/200 - (37*3^(1/2)*dq4*dqr6*cos(q5)^2*cos(q6)*sin(q4))/2000 + (29*dq1*dqr6*cos(q2)*cos(q4)*cos(q6)*sin(q5))/200 + (29*dq1*dqr6*cos(q2)*cos(q5)*cos(q6)*sin(q4))/100 - (29*dq2*dqr6*cos(q4)*cos(q5)*cos(q6)*sin(q3))/100 + (29*dq3*dqr6*cos(q4)*cos(q5)*cos(q6)*sin(q3))/100 + (29*dq4*dqr6*cos(q3)*cos(q4)*cos(q6)*sin(q5))/200 + (29*dq4*dqr6*cos(q3)*cos(q5)*cos(q6)*sin(q4))/100 + (29*dq5*dqr6*cos(q3)*cos(q4)*cos(q6)*sin(q5))/100 + (29*dq5*dqr6*cos(q3)*cos(q5)*cos(q6)*sin(q4))/200 + (29*dq6*dqr6*cos(q3)*cos(q4)*cos(q6)*sin(q5))/200 + (29*dq6*dqr6*cos(q3)*cos(q5)*cos(q6)*sin(q4))/400 - (2631*dq1*dqr6*cos(q4)*sin(q2)*sin(q3)*sin(q6))/16000 - (29*dq1*dqr6*cos(q2)*sin(q4)*sin(q5)*sin(q6))/200 + (29*dq2*dqr6*cos(q4)*sin(q3)*sin(q5)*sin(q6))/200 + (29*dq2*dqr6*cos(q5)*sin(q3)*sin(q4)*sin(q6))/400 + (29*dq2*dqr6*cos(q6)*sin(q3)*sin(q4)*sin(q5))/200 - (29*dq3*dqr6*cos(q4)*sin(q3)*sin(q5)*sin(q6))/200 - (29*dq3*dqr6*cos(q5)*sin(q3)*sin(q4)*sin(q6))/400 - (29*dq3*dqr6*cos(q6)*sin(q3)*sin(q4)*sin(q5))/200 - (29*dq4*dqr6*cos(q3)*sin(q4)*sin(q5)*sin(q6))/200 - (29*dq5*dqr6*cos(q3)*sin(q4)*sin(q5)*sin(q6))/400 - (29*dq6*dqr6*cos(q3)*sin(q4)*sin(q5)*sin(q6))/200 - dq5*dqr6*cos(q5)*cos(q6)*sin(q4)*((37*3^(1/2))/2000 + 1577/10000) - dq6*dqr6*cos(q5)*cos(q6)*sin(q4)*((111*3^(1/2))/4000 + 1577/20000) - (37*dq1*dqr6*cos(q2)*cos(q4)^2*cos(q6)*sin(q3))/2000 + (37*dq1*dqr6*cos(q3)*cos(q4)^2*cos(q6)*sin(q2))/2000 - (37*dq1*dqr6*cos(q2)*cos(q5)^2*cos(q6)*sin(q3))/2000 + (37*dq1*dqr6*cos(q3)*cos(q5)^2*cos(q6)*sin(q2))/2000 + (37*dq2*dqr6*cos(q4)*cos(q5)^2*cos(q6)*sin(q4))/1000 + (37*dq2*dqr6*cos(q4)^2*cos(q5)*cos(q6)*sin(q5))/800 - (37*dq3*dqr6*cos(q4)*cos(q5)^2*cos(q6)*sin(q4))/1000 - (37*dq3*dqr6*cos(q4)^2*cos(q5)*cos(q6)*sin(q5))/800 + dq6*dqr6*sin(q4)*sin(q5)*sin(q6)*((37*3^(1/2))/2000 + 1577/10000) + dq5*dqr6*sin(q4)*sin(q5)*sin(q6)*((37*3^(1/2))/4000 + 1577/20000) + (37*3^(1/2)*dq4*dqr6*cos(q5)*sin(q4)*sin(q5)*sin(q6))/4000 + (37*dq1*dqr6*cos(q2)*cos(q4)^2*cos(q5)^2*cos(q6)*sin(q3))/1000 - (37*dq1*dqr6*cos(q3)*cos(q4)^2*cos(q5)^2*cos(q6)*sin(q2))/1000 - (877*dq1*dqr6*cos(q2)*cos(q3)*cos(q4)*cos(q6)*sin(q5))/8000 - (877*dq1*dqr6*cos(q2)*cos(q3)*cos(q5)*cos(q6)*sin(q4))/4000 + (877*dq1*dqr6*cos(q2)*cos(q3)*sin(q4)*sin(q5)*sin(q6))/8000 - (877*dq1*dqr6*cos(q4)*cos(q6)*sin(q2)*sin(q3)*sin(q5))/8000 - (877*dq1*dqr6*cos(q5)*cos(q6)*sin(q2)*sin(q3)*sin(q4))/4000 + (37*dq1*dqr6*cos(q2)*cos(q5)*sin(q3)*sin(q5)*sin(q6))/4000 - (37*dq1*dqr6*cos(q3)*cos(q5)*sin(q2)*sin(q5)*sin(q6))/4000 - (37*dq2*dqr6*cos(q4)*cos(q5)*sin(q4)*sin(q5)*sin(q6))/2000 + (37*dq3*dqr6*cos(q4)*cos(q5)*sin(q4)*sin(q5)*sin(q6))/2000 + (877*dq1*dqr6*sin(q2)*sin(q3)*sin(q4)*sin(q5)*sin(q6))/8000 + dq1*dqr6*cos(q2)*cos(q5)*cos(q6)*sin(q3)*((641*3^(1/2))/20000 + 37/1000) - dq1*dqr6*cos(q3)*cos(q5)*cos(q6)*sin(q2)*((641*3^(1/2))/20000 + 37/1000) - dq2*dqr6*cos(q4)*cos(q5)*cos(q6)*sin(q4)*((641*3^(1/2))/20000 + 37/1000) + dq3*dqr6*cos(q4)*cos(q5)*cos(q6)*sin(q4)*((641*3^(1/2))/20000 + 37/1000) - dq1*dqr6*cos(q2)*sin(q3)*sin(q5)*sin(q6)*((641*3^(1/2))/40000 + 37/2000) + dq1*dqr6*cos(q3)*sin(q2)*sin(q5)*sin(q6)*((641*3^(1/2))/40000 + 37/2000) + dq2*dqr6*cos(q4)*sin(q4)*sin(q5)*sin(q6)*((641*3^(1/2))/40000 - 37/4000) - dq3*dqr6*cos(q4)*sin(q4)*sin(q5)*sin(q6)*((641*3^(1/2))/40000 - 37/4000) - (37*3^(1/2)*dq1*dqr6*cos(q2)*cos(q3)*cos(q5)^2*cos(q6)*sin(q4))/2000 - (37*3^(1/2)*dq1*dqr6*cos(q4)*cos(q5)^2*sin(q2)*sin(q3)*sin(q6))/8000 - (37*3^(1/2)*dq1*dqr6*cos(q5)^2*cos(q6)*sin(q2)*sin(q3)*sin(q4))/2000 - dq1*dqr6*cos(q4)*cos(q5)*sin(q2)*sin(q3)*sin(q6)*((111*3^(1/2))/8000 + 877/16000) + dq1*dqr6*cos(q2)*cos(q4)*sin(q3)*sin(q4)*sin(q6)*((1923*3^(1/2))/80000 + 37/800) - dq1*dqr6*cos(q3)*cos(q4)*sin(q2)*sin(q4)*sin(q6)*((1923*3^(1/2))/80000 + 37/800) - (37*dq1*dqr6*cos(q2)*cos(q4)*cos(q5)^2*sin(q3)*sin(q4)*sin(q6))/1600 + (37*dq1*dqr6*cos(q3)*cos(q4)*cos(q5)^2*sin(q2)*sin(q4)*sin(q6))/1600 - (37*dq1*dqr6*cos(q2)*cos(q4)^2*cos(q5)*sin(q3)*sin(q5)*sin(q6))/2000 + (37*dq1*dqr6*cos(q3)*cos(q4)^2*cos(q5)*sin(q2)*sin(q5)*sin(q6))/2000 - dq1*dqr6*cos(q2)*cos(q4)^2*cos(q5)*cos(q6)*sin(q3)*((641*3^(1/2))/20000 + 37/1000) + dq1*dqr6*cos(q3)*cos(q4)^2*cos(q5)*cos(q6)*sin(q2)*((641*3^(1/2))/20000 + 37/1000) + dq1*dqr6*cos(q2)*cos(q4)^2*sin(q3)*sin(q5)*sin(q6)*((641*3^(1/2))/40000 - 37/4000) - dq1*dqr6*cos(q3)*cos(q4)^2*sin(q2)*sin(q5)*sin(q6)*((641*3^(1/2))/40000 - 37/4000) - (37*dq1*dqr6*cos(q2)*cos(q4)*cos(q5)*cos(q6)*sin(q3)*sin(q4)*sin(q5))/800 + (37*dq1*dqr6*cos(q3)*cos(q4)*cos(q5)*cos(q6)*sin(q2)*sin(q4)*sin(q5))/800 + dq1*dqr6*cos(q2)*cos(q4)*cos(q6)*sin(q3)*sin(q4)*sin(q5)*((641*3^(1/2))/40000 + 37/2000) - dq1*dqr6*cos(q3)*cos(q4)*cos(q6)*sin(q2)*sin(q4)*sin(q5)*((641*3^(1/2))/40000 + 37/2000) + dq1*dqr6*cos(q2)*cos(q4)*cos(q5)*sin(q3)*sin(q4)*sin(q6)*((641*3^(1/2))/80000 - 37/8000) - dq1*dqr6*cos(q3)*cos(q4)*cos(q5)*sin(q2)*sin(q4)*sin(q6)*((641*3^(1/2))/80000 - 37/8000) - (37*3^(1/2)*dq1*dqr6*cos(q2)*cos(q3)*cos(q4)*cos(q5)*cos(q6)*sin(q5))/4000 + (37*3^(1/2)*dq1*dqr6*cos(q2)*cos(q3)*cos(q5)*sin(q4)*sin(q5)*sin(q6))/4000 - (37*3^(1/2)*dq1*dqr6*cos(q4)*cos(q5)*cos(q6)*sin(q2)*sin(q3)*sin(q5))/4000 + (37*3^(1/2)*dq1*dqr6*cos(q5)*sin(q2)*sin(q3)*sin(q4)*sin(q5)*sin(q6))/4000;
Y2_10_9=dq2*dqr6*sin(q6)*((1577*3^(1/2))/20000 + 111/4000) - dq3*dqr6*sin(q6)*((1577*3^(1/2))/20000 + 111/4000) - (37*dq2*dqr6*cos(q5)^2*sin(q6))/2000 + (37*dq3*dqr6*cos(q5)^2*sin(q6))/2000 - (37*ddqr1*cos(q3)*sin(q2)*sin(q6))/2000 - (87*ddqr2*cos(q6)*sin(q3)*sin(q4))/200 + (87*ddqr3*cos(q6)*sin(q3)*sin(q4))/400 - (2631*dq4*dqr6*cos(q4)*sin(q6))/16000 + (21*ddqr1*cos(q2)*cos(q6)*sin(q3)*sin(q4))/4000 - (21*ddqr1*cos(q3)*cos(q6)*sin(q2)*sin(q4))/4000 - (29*ddqr2*cos(q4)*cos(q6)*sin(q3)*sin(q5))/100 - (29*ddqr2*cos(q5)*cos(q6)*sin(q3)*sin(q4))/200 + (29*ddqr3*cos(q4)*cos(q6)*sin(q3)*sin(q5))/200 + (29*ddqr3*cos(q5)*cos(q6)*sin(q3)*sin(q4))/400 - (29*3^(1/2)*dq2*dqr6*cos(q3)*sin(q6))/400 + (29*3^(1/2)*dq3*dqr6*cos(q3)*sin(q6))/400 - (37*3^(1/2)*dq5*dqr6*cos(q4)*sin(q6))/4000 - (37*3^(1/2)*dq6*dqr6*cos(q4)*sin(q6))/2000 + (29*ddqr2*sin(q3)*sin(q4)*sin(q5)*sin(q6))/100 - (29*ddqr3*sin(q3)*sin(q4)*sin(q5)*sin(q6))/200 - dq2*dqr6*cos(q4)^2*sin(q6)*((1923*3^(1/2))/80000 + 37/800) + dq3*dqr6*cos(q4)^2*sin(q6)*((1923*3^(1/2))/80000 + 37/800) + (37*dq2*dqr6*cos(q4)^2*cos(q5)^2*sin(q6))/1600 - (37*dq3*dqr6*cos(q4)^2*cos(q5)^2*sin(q6))/1600 - (37*ddqr1*cos(q2)*cos(q4)^2*sin(q3)*sin(q6))/1000 + (37*ddqr1*cos(q3)*cos(q4)^2*sin(q2)*sin(q6))/1000 + (37*ddqr1*cos(q3)*cos(q5)^2*sin(q2)*sin(q6))/1000 + (87*dq1*dqr6*cos(q2)*cos(q4)*sin(q6))/400 + (87*dq4*dqr6*cos(q3)*cos(q4)*sin(q6))/400 - (37*dq2*dqr6*cos(q5)*cos(q6)*sin(q5))/1000 + (37*dq3*dqr6*cos(q5)*cos(q6)*sin(q5))/1000 - (877*dq4*dqr6*cos(q4)*cos(q6)*sin(q5))/8000 - (877*dq5*dqr6*cos(q4)*cos(q5)*sin(q6))/8000 - (877*dq5*dqr6*cos(q4)*cos(q6)*sin(q5))/4000 - (877*dq6*dqr6*cos(q4)*cos(q5)*sin(q6))/4000 - (7*3^(1/2)*ddqr1*cos(q6)*sin(q2)*sin(q3))/4000 - (29*3^(1/2)*ddqr5*cos(q6)*sin(q3)*sin(q5))/400 - (29*3^(1/2)*ddqr6*cos(q6)*sin(q3)*sin(q5))/200 - dq2*dqr6*cos(q6)*sin(q5)*((117*3^(1/2))/1250 - 37/2000) + dq3*dqr6*cos(q6)*sin(q5)*((117*3^(1/2))/1250 - 37/2000) - dq2*dqr6*cos(q5)*sin(q6)*((117*3^(1/2))/2500 - 37/4000) + dq3*dqr6*cos(q5)*sin(q6)*((117*3^(1/2))/2500 - 37/4000) + (7*ddqr1*cos(q2)*cos(q4)*cos(q6)*sin(q3)*sin(q5))/2000 + (7*ddqr1*cos(q2)*cos(q5)*cos(q6)*sin(q3)*sin(q4))/4000 - (7*ddqr1*cos(q3)*cos(q4)*cos(q5)*sin(q2)*sin(q6))/1000 - (7*ddqr1*cos(q3)*cos(q4)*cos(q6)*sin(q2)*sin(q5))/2000 - (7*ddqr1*cos(q3)*cos(q5)*cos(q6)*sin(q2)*sin(q4))/4000 + (1231*ddqr1*cos(q4)*cos(q5)*cos(q6)*sin(q2)*sin(q3))/40000 - (37*ddqr1*cos(q2)*cos(q5)*cos(q6)*sin(q3)*sin(q5))/2000 + (37*ddqr1*cos(q3)*cos(q5)*cos(q6)*sin(q2)*sin(q5))/2000 + (29*3^(1/2)*dq2*dqr6*cos(q3)*cos(q5)*sin(q6))/400 - (29*3^(1/2)*dq3*dqr6*cos(q3)*cos(q5)*sin(q6))/400 - (7*ddqr1*cos(q2)*sin(q3)*sin(q4)*sin(q5)*sin(q6))/2000 + (7*ddqr1*cos(q3)*sin(q2)*sin(q4)*sin(q5)*sin(q6))/2000 - (877*ddqr1*cos(q5)*sin(q2)*sin(q3)*sin(q4)*sin(q6))/4000 + dq3*dqr6*cos(q4)^2*cos(q6)*sin(q5)*((641*3^(1/2))/40000 + 37/2000) - dq2*dqr6*cos(q4)^2*cos(q5)*sin(q6)*((641*3^(1/2))/80000 - 37/8000) + dq3*dqr6*cos(q4)^2*cos(q5)*sin(q6)*((641*3^(1/2))/80000 - 37/8000) - ddqr1*cos(q3)*cos(q5)*sin(q2)*sin(q6)*((641*3^(1/2))/20000 + 37/1000) + ddqr1*cos(q2)*cos(q6)*sin(q3)*sin(q5)*((641*3^(1/2))/40000 - 37/4000) - ddqr1*cos(q3)*cos(q6)*sin(q2)*sin(q5)*((641*3^(1/2))/40000 - 37/4000) + ddqr1*cos(q4)*cos(q6)*sin(q2)*sin(q3)*((37*3^(1/2))/4000 + 7539/40000) - (37*3^(1/2)*dq4*dqr6*cos(q4)*cos(q5)^2*sin(q6))/8000 - (2631*dq1*dqr6*cos(q2)*cos(q3)*cos(q4)*sin(q6))/16000 + (29*dq1*dqr6*cos(q2)*cos(q4)*cos(q5)*sin(q6))/400 + (29*dq4*dqr6*cos(q3)*cos(q4)*cos(q5)*sin(q6))/400 + (29*dq5*dqr6*cos(q3)*cos(q4)*cos(q5)*sin(q6))/200 + (29*dq6*dqr6*cos(q3)*cos(q4)*cos(q5)*sin(q6))/100 + (7*3^(1/2)*ddqr1*cos(q5)*cos(q6)*sin(q2)*sin(q3))/4000 + (37*3^(1/2)*ddqr1*sin(q2)*sin(q3)*sin(q4)*sin(q6))/2000 - (7*3^(1/2)*ddqr1*sin(q2)*sin(q3)*sin(q5)*sin(q6))/2000 + (37*ddqr1*cos(q2)*cos(q4)^2*cos(q5)^2*sin(q3)*sin(q6))/500 - (37*ddqr1*cos(q3)*cos(q4)^2*cos(q5)^2*sin(q2)*sin(q6))/500 - dq6*dqr6*cos(q4)*cos(q6)*sin(q5)*((37*3^(1/2))/4000 + 877/8000) - dq4*dqr6*cos(q4)*cos(q5)*sin(q6)*((111*3^(1/2))/8000 + 877/16000) - ddqr1*cos(q2)*cos(q4)*cos(q6)*sin(q3)*sin(q4)*((1923*3^(1/2))/40000 + 37/400) + ddqr1*cos(q3)*cos(q4)*cos(q6)*sin(q2)*sin(q4)*((1923*3^(1/2))/40000 + 37/400) + (37*ddqr1*cos(q2)*cos(q4)*cos(q5)^2*cos(q6)*sin(q3)*sin(q4))/800 - (37*ddqr1*cos(q3)*cos(q4)*cos(q5)^2*cos(q6)*sin(q2)*sin(q4))/800 + (37*ddqr1*cos(q2)*cos(q4)^2*cos(q5)*cos(q6)*sin(q3)*sin(q5))/1000 - (37*ddqr1*cos(q3)*cos(q4)^2*cos(q5)*cos(q6)*sin(q2)*sin(q5))/1000 + ddqr1*cos(q6)*sin(q2)*sin(q3)*sin(q4)*sin(q5)*((37*3^(1/2))/4000 - 877/8000) + ddqr1*cos(q4)*sin(q2)*sin(q3)*sin(q5)*sin(q6)*((37*3^(1/2))/2000 - 1231/20000) - ddqr1*cos(q2)*cos(q4)^2*cos(q5)*sin(q3)*sin(q6)*((641*3^(1/2))/10000 + 37/500) + ddqr1*cos(q3)*cos(q4)^2*cos(q5)*sin(q2)*sin(q6)*((641*3^(1/2))/10000 + 37/500) - ddqr1*cos(q2)*cos(q4)^2*cos(q6)*sin(q3)*sin(q5)*((641*3^(1/2))/20000 - 37/2000) + ddqr1*cos(q3)*cos(q4)^2*cos(q6)*sin(q2)*sin(q5)*((641*3^(1/2))/20000 - 37/2000) + (37*3^(1/2)*ddqr1*cos(q4)*cos(q5)^2*cos(q6)*sin(q2)*sin(q3))/4000 - (37*3^(1/2)*ddqr1*cos(q5)^2*sin(q2)*sin(q3)*sin(q4)*sin(q6))/1000 - (37*3^(1/2)*dq4*dqr6*cos(q4)*cos(q5)*cos(q6)*sin(q5))/4000 + ddqr1*cos(q2)*cos(q4)*sin(q3)*sin(q4)*sin(q5)*sin(q6)*((641*3^(1/2))/20000 + 37/1000) - ddqr1*cos(q3)*cos(q4)*sin(q2)*sin(q4)*sin(q5)*sin(q6)*((641*3^(1/2))/20000 + 37/1000) - (37*3^(1/2)*dq1*dqr6*cos(q2)*cos(q3)*cos(q4)*cos(q5)^2*sin(q6))/8000 - (37*3^(1/2)*ddqr1*cos(q4)*cos(q5)*sin(q2)*sin(q3)*sin(q5)*sin(q6))/2000 - (37*3^(1/2)*ddqr1*cos(q5)*cos(q6)*sin(q2)*sin(q3)*sin(q4)*sin(q5))/2000 - dq1*dqr6*cos(q2)*cos(q3)*cos(q4)*cos(q5)*sin(q6)*((111*3^(1/2))/8000 + 877/16000) - (37*ddqr1*cos(q2)*cos(q4)*cos(q5)*sin(q3)*sin(q4)*sin(q5)*sin(q6))/400 + (37*ddqr1*cos(q3)*cos(q4)*cos(q5)*sin(q2)*sin(q4)*sin(q5)*sin(q6))/400 - ddqr1*cos(q2)*cos(q4)*cos(q5)*cos(q6)*sin(q3)*sin(q4)*((641*3^(1/2))/40000 - 37/4000) + ddqr1*cos(q3)*cos(q4)*cos(q5)*cos(q6)*sin(q2)*sin(q4)*((641*3^(1/2))/40000 - 37/4000);
Y2_10_10=ddqr3*cos(q6)*((1577*3^(1/2))/10000 + 111/2000) - ddqr2*cos(q6)*((1577*3^(1/2))/10000 + 111/2000) + (37*ddqr2*cos(q5)^2*cos(q6))/1000 - (37*ddqr3*cos(q5)^2*cos(q6))/1000 - (37*ddqr2*cos(q4)^2*cos(q5)^2*cos(q6))/800 + (37*ddqr3*cos(q4)^2*cos(q5)^2*cos(q6))/800 - (87*ddqr1*cos(q2)*cos(q4)*cos(q6))/400 - (87*ddqr4*cos(q3)*cos(q4)*cos(q6))/400 + (1231*ddqr4*cos(q4)*cos(q5)*cos(q6))/40000 + (877*ddqr6*cos(q4)*cos(q5)*cos(q6))/4000 + (37*ddqr1*cos(q2)*sin(q3)*sin(q6))/2000 - (37*ddqr2*cos(q4)*sin(q4)*sin(q6))/1000 + (37*ddqr3*cos(q4)*sin(q4)*sin(q6))/1000 - (37*ddqr2*cos(q5)*sin(q5)*sin(q6))/500 + (37*ddqr3*cos(q5)*sin(q5)*sin(q6))/500 - (877*ddqr4*cos(q5)*sin(q4)*sin(q6))/4000 + (87*ddqr6*cos(q3)*sin(q4)*sin(q6))/400 - (877*ddqr5*cos(q4)*sin(q5)*sin(q6))/4000 + ddqr2*cos(q5)*cos(q6)*((117*3^(1/2))/1250 - 37/2000) - ddqr3*cos(q5)*cos(q6)*((117*3^(1/2))/1250 - 37/2000) + ddqr4*cos(q4)*cos(q6)*((37*3^(1/2))/4000 + 7539/40000) - ddqr2*sin(q5)*sin(q6)*((117*3^(1/2))/625 - 37/1000) + ddqr3*sin(q5)*sin(q6)*((117*3^(1/2))/625 - 37/1000) + ddqr6*sin(q4)*sin(q6)*((37*3^(1/2))/4000 - 351/2500) + (29*3^(1/2)*ddqr2*cos(q3)*cos(q6))/200 - (29*3^(1/2)*ddqr3*cos(q3)*cos(q6))/400 + (37*3^(1/2)*ddqr5*cos(q4)*cos(q6))/2000 + (37*3^(1/2)*ddqr6*cos(q4)*cos(q6))/2000 + ddqr2*cos(q4)^2*cos(q6)*((1923*3^(1/2))/40000 + 37/400) - ddqr3*cos(q4)^2*cos(q6)*((1923*3^(1/2))/40000 + 37/400) + (37*3^(1/2)*ddqr4*sin(q4)*sin(q6))/2000 + (29*3^(1/2)*ddqr6*sin(q3)*sin(q6))/400 + (37*3^(1/2)*ddqr4*cos(q4)*cos(q5)^2*cos(q6))/4000 - (29*ddqr1*cos(q2)*cos(q4)*cos(q5)*cos(q6))/400 - (29*ddqr4*cos(q3)*cos(q4)*cos(q5)*cos(q6))/400 - (29*ddqr5*cos(q3)*cos(q4)*cos(q5)*cos(q6))/200 - (29*ddqr6*cos(q3)*cos(q4)*cos(q5)*cos(q6))/100 - (37*3^(1/2)*ddqr4*cos(q5)^2*sin(q4)*sin(q6))/1000 + (29*ddqr1*cos(q2)*cos(q4)*sin(q5)*sin(q6))/200 + (29*ddqr1*cos(q2)*cos(q5)*sin(q4)*sin(q6))/100 + (29*ddqr1*cos(q2)*cos(q6)*sin(q4)*sin(q5))/200 - (29*ddqr2*cos(q4)*cos(q5)*sin(q3)*sin(q6))/50 + (29*ddqr3*cos(q4)*cos(q5)*sin(q3)*sin(q6))/100 + (29*ddqr4*cos(q3)*cos(q4)*sin(q5)*sin(q6))/200 + (29*ddqr4*cos(q3)*cos(q5)*sin(q4)*sin(q6))/100 + (29*ddqr4*cos(q3)*cos(q6)*sin(q4)*sin(q5))/200 + (29*ddqr5*cos(q3)*cos(q4)*sin(q5)*sin(q6))/100 + (29*ddqr5*cos(q3)*cos(q5)*sin(q4)*sin(q6))/200 + (29*ddqr5*cos(q3)*cos(q6)*sin(q4)*sin(q5))/400 + (29*ddqr6*cos(q3)*cos(q4)*sin(q5)*sin(q6))/200 + (29*ddqr6*cos(q3)*cos(q5)*sin(q4)*sin(q6))/400 + (29*ddqr6*cos(q3)*cos(q6)*sin(q4)*sin(q5))/200 - ddqr5*cos(q4)*cos(q5)*cos(q6)*((37*3^(1/2))/4000 - 877/8000) + ddqr4*cos(q6)*sin(q4)*sin(q5)*((37*3^(1/2))/4000 - 877/8000) - ddqr6*cos(q4)*sin(q5)*sin(q6)*((37*3^(1/2))/4000 + 877/8000) - ddqr5*cos(q5)*sin(q4)*sin(q6)*((37*3^(1/2))/2000 + 1577/10000) - ddqr6*cos(q6)*sin(q4)*sin(q5)*((37*3^(1/2))/2000 + 1577/10000) + ddqr4*cos(q4)*sin(q5)*sin(q6)*((37*3^(1/2))/2000 - 1231/20000) + ddqr5*cos(q6)*sin(q4)*sin(q5)*((37*3^(1/2))/4000 - 1577/20000) - ddqr6*cos(q5)*sin(q4)*sin(q6)*((111*3^(1/2))/4000 + 1577/20000) - (37*ddqr1*cos(q2)*cos(q5)^2*sin(q3)*sin(q6))/1000 + (37*ddqr2*cos(q4)*cos(q5)^2*sin(q4)*sin(q6))/500 + (37*ddqr2*cos(q4)^2*cos(q5)*sin(q5)*sin(q6))/400 - (37*ddqr3*cos(q4)*cos(q5)^2*sin(q4)*sin(q6))/500 - (37*ddqr3*cos(q4)^2*cos(q5)*sin(q5)*sin(q6))/400 - (7*3^(1/2)*ddqr1*cos(q2)*cos(q3)*cos(q6))/4000 - (29*3^(1/2)*ddqr2*cos(q3)*cos(q5)*cos(q6))/200 + (29*3^(1/2)*ddqr3*cos(q3)*cos(q5)*cos(q6))/400 + ddqr2*cos(q4)^2*cos(q5)*cos(q6)*((641*3^(1/2))/40000 - 37/4000) - ddqr3*cos(q4)^2*cos(q5)*cos(q6)*((641*3^(1/2))/40000 - 37/4000) + (29*3^(1/2)*ddqr2*cos(q3)*sin(q5)*sin(q6))/100 - (29*3^(1/2)*ddqr3*cos(q3)*sin(q5)*sin(q6))/200 - (29*3^(1/2)*ddqr5*cos(q5)*sin(q3)*sin(q6))/200 - (29*3^(1/2)*ddqr6*cos(q5)*sin(q3)*sin(q6))/400 - ddqr2*cos(q4)^2*sin(q5)*sin(q6)*((641*3^(1/2))/20000 + 37/1000) + ddqr3*cos(q4)^2*sin(q5)*sin(q6)*((641*3^(1/2))/20000 + 37/1000) - (877*ddqr1*cos(q2)*cos(q3)*cos(q5)*sin(q4)*sin(q6))/4000 + (7*ddqr1*cos(q2)*cos(q4)*cos(q5)*sin(q3)*sin(q6))/1000 + (37*ddqr2*cos(q4)*cos(q5)*cos(q6)*sin(q4)*sin(q5))/1000 - (37*ddqr3*cos(q4)*cos(q5)*cos(q6)*sin(q4)*sin(q5))/1000 + ddqr1*cos(q2)*cos(q3)*cos(q4)*cos(q6)*((37*3^(1/2))/4000 + 7539/40000) - ddqr2*cos(q4)*cos(q5)*sin(q4)*sin(q6)*((641*3^(1/2))/10000 + 37/500) + ddqr3*cos(q4)*cos(q5)*sin(q4)*sin(q6)*((641*3^(1/2))/10000 + 37/500) + ddqr1*cos(q2)*cos(q5)*sin(q3)*sin(q6)*((641*3^(1/2))/20000 + 37/1000) - ddqr2*cos(q4)*cos(q6)*sin(q4)*sin(q5)*((641*3^(1/2))/20000 - 37/2000) + ddqr3*cos(q4)*cos(q6)*sin(q4)*sin(q5)*((641*3^(1/2))/20000 - 37/2000) + (7*3^(1/2)*ddqr1*cos(q2)*cos(q3)*cos(q5)*cos(q6))/4000 + (37*3^(1/2)*ddqr1*cos(q2)*cos(q3)*sin(q4)*sin(q6))/2000 - (7*3^(1/2)*ddqr1*cos(q2)*cos(q3)*sin(q5)*sin(q6))/2000 - (37*3^(1/2)*ddqr4*cos(q4)*cos(q5)*sin(q5)*sin(q6))/2000 - (37*3^(1/2)*ddqr4*cos(q5)*cos(q6)*sin(q4)*sin(q5))/2000 + (1231*ddqr1*cos(q2)*cos(q3)*cos(q4)*cos(q5)*cos(q6))/40000 + ddqr1*cos(q2)*cos(q3)*cos(q6)*sin(q4)*sin(q5)*((37*3^(1/2))/4000 - 877/8000) + ddqr1*cos(q2)*cos(q3)*cos(q4)*sin(q5)*sin(q6)*((37*3^(1/2))/2000 - 1231/20000) + (37*3^(1/2)*ddqr1*cos(q2)*cos(q3)*cos(q4)*cos(q5)^2*cos(q6))/4000 - (37*3^(1/2)*ddqr1*cos(q2)*cos(q3)*cos(q5)^2*sin(q4)*sin(q6))/1000 - (37*3^(1/2)*ddqr1*cos(q2)*cos(q3)*cos(q4)*cos(q5)*sin(q5)*sin(q6))/2000 - (37*3^(1/2)*ddqr1*cos(q2)*cos(q3)*cos(q5)*cos(q6)*sin(q4)*sin(q5))/2000;
Y2_11_1=(29*sin(q2))/100;
Y2_12_1=(29*sin(q2))/100 + (1231*cos(q2)*sin(q3))/10000 - (1231*cos(q3)*sin(q2))/10000;
Y2_13_1=(29*sin(q2))/100 + (117*cos(q2)*sin(q3))/625 - (117*cos(q3)*sin(q2))/625 + (37*sin(q2)*sin(q3)*sin(q4))/1000 + (37*cos(q2)*cos(q3)*sin(q4))/1000;
Y2_14_1=(29*sin(q2))/100 + (877*cos(q2)*sin(q3))/4000 - (877*cos(q3)*sin(q2))/4000 + cos(q2)*cos(q3)*sin(q4)*((641*3^(1/2))/20000 + 37/1000) + sin(q2)*sin(q3)*sin(q4)*((641*3^(1/2))/20000 + 37/1000) + (37*3^(1/2)*cos(q2)*cos(q5)*sin(q3))/2000 - (37*3^(1/2)*cos(q3)*cos(q5)*sin(q2))/2000 - (37*cos(q2)*cos(q3)*cos(q4)*sin(q5))/1000 - (37*cos(q2)*cos(q3)*cos(q5)*sin(q4))/2000 - (37*cos(q4)*sin(q2)*sin(q3)*sin(q5))/1000 - (37*cos(q5)*sin(q2)*sin(q3)*sin(q4))/2000;
Y2_16_1=ddqr2 - (dq1*dqr1*sin(2*q2))/2;
Y2_17_1=ddqr2 - ddqr3 + (dq1*dqr1*sin(2*q2))/2 - (dq1*dqr1*sin(2*q3))/2 - 2*dq1*dqr1*cos(q2)*cos(q3)^2*sin(q2) + 2*dq1*dqr1*cos(q2)^2*cos(q3)*sin(q3);
Y2_18_1=ddqr2 - ddqr3 - ddqr2*cos(q4)^2 + ddqr3*cos(q4)^2 - (dq1*dqr1*sin(2*q2))/2 + (dq1*dqr1*sin(2*q3))/2 + (dq2*dqr4*sin(2*q4))/2 + (dq4*dqr2*sin(2*q4))/2 - (dq3*dqr4*sin(2*q4))/2 - (dq4*dqr3*sin(2*q4))/2 - dq1*dqr4*cos(q2)*sin(q3) + dq1*dqr4*cos(q3)*sin(q2) - dq4*dqr1*cos(q2)*sin(q3) + dq4*dqr1*cos(q3)*sin(q2) + 2*dq1*dqr1*cos(q2)*cos(q3)^2*sin(q2) + dq1*dqr1*cos(q2)*cos(q4)^2*sin(q2) - 2*dq1*dqr1*cos(q2)^2*cos(q3)*sin(q3) - dq1*dqr1*cos(q3)*cos(q4)^2*sin(q3) + dq1*dqr4*cos(q2)*cos(q4)^2*sin(q3) - dq1*dqr4*cos(q3)*cos(q4)^2*sin(q2) + dq4*dqr1*cos(q2)*cos(q4)^2*sin(q3) - dq4*dqr1*cos(q3)*cos(q4)^2*sin(q2) + ddqr1*cos(q2)*cos(q4)*sin(q3)*sin(q4) - ddqr1*cos(q3)*cos(q4)*sin(q2)*sin(q4) - 2*dq1*dqr1*cos(q2)*cos(q3)^2*cos(q4)^2*sin(q2) + 2*dq1*dqr1*cos(q2)^2*cos(q3)*cos(q4)^2*sin(q3);
Y2_19_1=(dq3*dqr4*sin(2*q4))/2 - (dq4*dqr2*sin(2*q4))/2 - (dq2*dqr4*sin(2*q5))/4 - (dq2*dqr4*sin(2*q4))/2 - (dq4*dqr2*sin(2*q5))/4 + (dq4*dqr3*sin(2*q4))/2 - (dq5*dqr2*sin(2*q4))/4 + (dq3*dqr4*sin(2*q5))/4 + (dq4*dqr3*sin(2*q5))/4 - (dq5*dqr2*sin(2*q5))/2 + (dq5*dqr3*sin(2*q4))/4 + (dq5*dqr3*sin(2*q5))/2 - dq1*dqr1*cos(q2)*cos(q4)^2*sin(q2) + (dq1*dqr1*cos(q2)*cos(q5)^2*sin(q2))/2 + dq1*dqr1*cos(q3)*cos(q4)^2*sin(q3) - (dq1*dqr1*cos(q3)*cos(q5)^2*sin(q3))/2 - dq1*dqr4*cos(q2)*cos(q4)^2*sin(q3) + dq1*dqr4*cos(q3)*cos(q4)^2*sin(q2) - dq4*dqr1*cos(q2)*cos(q4)^2*sin(q3) + dq4*dqr1*cos(q3)*cos(q4)^2*sin(q2) - (dq1*dqr4*cos(q2)*cos(q5)^2*sin(q3))/4 + (dq1*dqr4*cos(q3)*cos(q5)^2*sin(q2))/4 - (dq1*dqr5*cos(q2)*cos(q4)^2*sin(q3))/2 + (dq1*dqr5*cos(q3)*cos(q4)^2*sin(q2))/2 - (dq4*dqr1*cos(q2)*cos(q5)^2*sin(q3))/4 + (dq4*dqr1*cos(q3)*cos(q5)^2*sin(q2))/4 - (dq5*dqr1*cos(q2)*cos(q4)^2*sin(q3))/2 + (dq5*dqr1*cos(q3)*cos(q4)^2*sin(q2))/2 - (dq1*dqr5*cos(q2)*cos(q5)^2*sin(q3))/2 + (dq1*dqr5*cos(q3)*cos(q5)^2*sin(q2))/2 - (dq5*dqr1*cos(q2)*cos(q5)^2*sin(q3))/2 + (dq5*dqr1*cos(q3)*cos(q5)^2*sin(q2))/2 + (5*dq2*dqr4*cos(q4)*cos(q5)^2*sin(q4))/4 + (5*dq4*dqr2*cos(q4)*cos(q5)^2*sin(q4))/4 + dq2*dqr4*cos(q4)^2*cos(q5)*sin(q5) - (5*dq3*dqr4*cos(q4)*cos(q5)^2*sin(q4))/4 + dq4*dqr2*cos(q4)^2*cos(q5)*sin(q5) - (5*dq4*dqr3*cos(q4)*cos(q5)^2*sin(q4))/4 + dq5*dqr2*cos(q4)*cos(q5)^2*sin(q4) - dq3*dqr4*cos(q4)^2*cos(q5)*sin(q5) - dq4*dqr3*cos(q4)^2*cos(q5)*sin(q5) + (5*dq5*dqr2*cos(q4)^2*cos(q5)*sin(q5))/4 - dq5*dqr3*cos(q4)*cos(q5)^2*sin(q4) - (5*dq5*dqr3*cos(q4)^2*cos(q5)*sin(q5))/4 - (3^(1/2)*dq1*dqr1*cos(q5)^2*sin(q4))/4 - (3^(1/2)*dq4*dqr4*cos(q5)^2*sin(q4))/4 - (3^(1/2)*dq5*dqr4*cos(q5)^2*sin(q4))/2 - (3^(1/2)*dq1*dqr1*cos(q4)*cos(q5)*sin(q5))/2 - (3^(1/2)*dq4*dqr4*cos(q4)*cos(q5)*sin(q5))/2 - (3^(1/2)*dq5*dqr4*cos(q4)*cos(q5)*sin(q5))/4 + 2*dq1*dqr1*cos(q2)*cos(q3)^2*cos(q4)^2*sin(q2) - dq1*dqr1*cos(q2)*cos(q3)^2*cos(q5)^2*sin(q2) - 2*dq1*dqr1*cos(q2)^2*cos(q3)*cos(q4)^2*sin(q3) + (5*dq1*dqr1*cos(q2)*cos(q4)^2*cos(q5)^2*sin(q2))/4 + dq1*dqr1*cos(q2)^2*cos(q3)*cos(q5)^2*sin(q3) - (5*dq1*dqr1*cos(q3)*cos(q4)^2*cos(q5)^2*sin(q3))/4 + (5*dq1*dqr4*cos(q2)*cos(q4)^2*cos(q5)^2*sin(q3))/4 - (5*dq1*dqr4*cos(q3)*cos(q4)^2*cos(q5)^2*sin(q2))/4 + (5*dq4*dqr1*cos(q2)*cos(q4)^2*cos(q5)^2*sin(q3))/4 - (5*dq4*dqr1*cos(q3)*cos(q4)^2*cos(q5)^2*sin(q2))/4 + dq1*dqr5*cos(q2)*cos(q4)^2*cos(q5)^2*sin(q3) - dq1*dqr5*cos(q3)*cos(q4)^2*cos(q5)^2*sin(q2) + dq5*dqr1*cos(q2)*cos(q4)^2*cos(q5)^2*sin(q3) - dq5*dqr1*cos(q3)*cos(q4)^2*cos(q5)^2*sin(q2) + (3^(1/2)*dq1*dqr1*cos(q2)^2*cos(q5)^2*sin(q4))/2 + (3^(1/2)*dq1*dqr1*cos(q3)^2*cos(q5)^2*sin(q4))/2 - 3^(1/2)*dq1*dqr1*cos(q2)^2*cos(q3)^2*cos(q5)^2*sin(q4) + 3^(1/2)*dq1*dqr1*cos(q2)^2*cos(q4)*cos(q5)*sin(q5) + 3^(1/2)*dq1*dqr1*cos(q3)^2*cos(q4)*cos(q5)*sin(q5) - (3^(1/2)*dq1*dqr4*cos(q2)*cos(q3)*cos(q5)^2*sin(q4))/4 - (3^(1/2)*dq4*dqr1*cos(q2)*cos(q3)*cos(q5)^2*sin(q4))/4 - (3^(1/2)*dq5*dqr1*cos(q2)*cos(q3)*cos(q5)^2*sin(q4))/2 - (3^(1/2)*dq1*dqr4*cos(q5)^2*sin(q2)*sin(q3)*sin(q4))/4 - (3^(1/2)*dq4*dqr1*cos(q5)^2*sin(q2)*sin(q3)*sin(q4))/4 - (3^(1/2)*dq1*dqr5*cos(q5)^2*sin(q2)*sin(q3)*sin(q4))/2 - (3^(1/2)*dq5*dqr1*cos(q5)^2*sin(q2)*sin(q3)*sin(q4))/2 - (5*dq1*dqr1*cos(q2)*cos(q3)^2*cos(q4)^2*cos(q5)^2*sin(q2))/2 + (5*dq1*dqr1*cos(q2)^2*cos(q3)*cos(q4)^2*cos(q5)^2*sin(q3))/2 - dq1*dqr1*cos(q2)*cos(q4)*cos(q5)*sin(q2)*sin(q4)*sin(q5) + dq1*dqr1*cos(q3)*cos(q4)*cos(q5)*sin(q3)*sin(q4)*sin(q5) - dq1*dqr4*cos(q2)*cos(q4)*cos(q5)*sin(q3)*sin(q4)*sin(q5) + dq1*dqr4*cos(q3)*cos(q4)*cos(q5)*sin(q2)*sin(q4)*sin(q5) - dq4*dqr1*cos(q2)*cos(q4)*cos(q5)*sin(q3)*sin(q4)*sin(q5) + dq4*dqr1*cos(q3)*cos(q4)*cos(q5)*sin(q2)*sin(q4)*sin(q5) - (5*dq1*dqr5*cos(q2)*cos(q4)*cos(q5)*sin(q3)*sin(q4)*sin(q5))/4 + (5*dq1*dqr5*cos(q3)*cos(q4)*cos(q5)*sin(q2)*sin(q4)*sin(q5))/4 - (5*dq5*dqr1*cos(q2)*cos(q4)*cos(q5)*sin(q3)*sin(q4)*sin(q5))/4 + (5*dq5*dqr1*cos(q3)*cos(q4)*cos(q5)*sin(q2)*sin(q4)*sin(q5))/4 - 2*3^(1/2)*dq1*dqr1*cos(q2)^2*cos(q3)^2*cos(q4)*cos(q5)*sin(q5) - (3^(1/2)*dq1*dqr4*cos(q2)*cos(q3)*cos(q4)*cos(q5)*sin(q5))/2 - (3^(1/2)*dq4*dqr1*cos(q2)*cos(q3)*cos(q4)*cos(q5)*sin(q5))/2 - (3^(1/2)*dq5*dqr1*cos(q2)*cos(q3)*cos(q4)*cos(q5)*sin(q5))/4 - (3^(1/2)*dq1*dqr4*cos(q4)*cos(q5)*sin(q2)*sin(q3)*sin(q5))/2 - (3^(1/2)*dq4*dqr1*cos(q4)*cos(q5)*sin(q2)*sin(q3)*sin(q5))/2 - (3^(1/2)*dq1*dqr5*cos(q4)*cos(q5)*sin(q2)*sin(q3)*sin(q5))/4 - (3^(1/2)*dq5*dqr1*cos(q4)*cos(q5)*sin(q2)*sin(q3)*sin(q5))/4 - 3^(1/2)*dq1*dqr1*cos(q2)*cos(q3)*cos(q5)^2*sin(q2)*sin(q3)*sin(q4) + 2*dq1*dqr1*cos(q2)*cos(q3)^2*cos(q4)*cos(q5)*sin(q2)*sin(q4)*sin(q5) - 2*dq1*dqr1*cos(q2)^2*cos(q3)*cos(q4)*cos(q5)*sin(q3)*sin(q4)*sin(q5) - 2*3^(1/2)*dq1*dqr1*cos(q2)*cos(q3)*cos(q4)*cos(q5)*sin(q2)*sin(q3)*sin(q5);
Y2_19_2=ddqr2*cos(q4)^2 + ddqr2*cos(q5)^2 - ddqr3*cos(q4)^2 - ddqr3*cos(q5)^2 - (5*ddqr2*cos(q4)^2*cos(q5)^2)/4 + (5*ddqr3*cos(q4)^2*cos(q5)^2)/4 - (dq2*dqr5*sin(2*q4))/4 - (dq2*dqr5*sin(2*q5))/2 + (dq3*dqr5*sin(2*q4))/4 + (dq3*dqr5*sin(2*q5))/2 + (3^(1/2)*ddqr5*cos(q4))/2 + (3^(1/2)*ddqr4*cos(q4)*cos(q5)^2)/4 + dq2*dqr5*cos(q4)*cos(q5)^2*sin(q4) + (5*dq2*dqr5*cos(q4)^2*cos(q5)*sin(q5))/4 - dq3*dqr5*cos(q4)*cos(q5)^2*sin(q4) - (5*dq3*dqr5*cos(q4)^2*cos(q5)*sin(q5))/4 - ddqr1*cos(q2)*cos(q4)*sin(q3)*sin(q4) + ddqr1*cos(q3)*cos(q4)*sin(q2)*sin(q4) - (ddqr1*cos(q2)*cos(q5)*sin(q3)*sin(q5))/2 + (ddqr1*cos(q3)*cos(q5)*sin(q2)*sin(q5))/2 + ddqr2*cos(q4)*cos(q5)*sin(q4)*sin(q5) - ddqr3*cos(q4)*cos(q5)*sin(q4)*sin(q5) - (3^(1/2)*dq4*dqr5*cos(q5)^2*sin(q4))/2 - (3^(1/2)*ddqr4*cos(q5)*sin(q4)*sin(q5))/2 - (3^(1/2)*dq4*dqr5*cos(q4)*cos(q5)*sin(q5))/4 + (5*ddqr1*cos(q2)*cos(q4)*cos(q5)^2*sin(q3)*sin(q4))/4 - (5*ddqr1*cos(q3)*cos(q4)*cos(q5)^2*sin(q2)*sin(q4))/4 + ddqr1*cos(q2)*cos(q4)^2*cos(q5)*sin(q3)*sin(q5) - ddqr1*cos(q3)*cos(q4)^2*cos(q5)*sin(q2)*sin(q5) + (3^(1/2)*ddqr1*cos(q2)*cos(q3)*cos(q4)*cos(q5)^2)/4 + (3^(1/2)*ddqr1*cos(q4)*cos(q5)^2*sin(q2)*sin(q3))/4 - (3^(1/2)*dq1*dqr5*cos(q2)*cos(q3)*cos(q5)^2*sin(q4))/2 - (3^(1/2)*ddqr1*cos(q2)*cos(q3)*cos(q5)*sin(q4)*sin(q5))/2 - (3^(1/2)*ddqr1*cos(q5)*sin(q2)*sin(q3)*sin(q4)*sin(q5))/2 - (3^(1/2)*dq1*dqr5*cos(q2)*cos(q3)*cos(q4)*cos(q5)*sin(q5))/4;
Y2_20_1=(3*3^(1/2)*dq6*dqr1*cos(q4)*sin(q2)*sin(q3)*sin(q5))/8 - (3^(1/2)*dq5*dqr1*sin(q2)*sin(q3)*sin(q4))/2 - (3^(1/2)*dq6*dqr1*sin(q2)*sin(q3)*sin(q4))/4 - (3^(1/2)*dq4*dqr1*sin(q2)*sin(q3)*sin(q4))/4 + (3^(1/2)*dq4*dqr1*cos(q5)^2*sin(q2)*sin(q3)*sin(q4))/4 + (7*3^(1/2)*dq4*dqr1*cos(q6)^2*sin(q2)*sin(q3)*sin(q4))/16 + (3^(1/2)*dq5*dqr1*cos(q5)^2*sin(q2)*sin(q3)*sin(q4))/2 + (3^(1/2)*dq5*dqr1*cos(q6)^2*sin(q2)*sin(q3)*sin(q4))/2 + (3^(1/2)*dq6*dqr1*cos(q5)^2*sin(q2)*sin(q3)*sin(q4))/4 + (3^(1/2)*dq6*dqr1*cos(q6)^2*sin(q2)*sin(q3)*sin(q4))/4 + (3*dq1*dqr1*cos(q2)*cos(q6)*sin(q2)*sin(q5)*sin(q6))/2 - (3*dq6*dqr1*cos(q3)*cos(q4)*sin(q2)*sin(q4)*sin(q5))/8 + (3^(1/2)*dq4*dqr1*cos(q4)*cos(q6)^2*sin(q2)*sin(q3)*sin(q5))/8 - (3^(1/2)*dq4*dqr1*cos(q5)*cos(q6)^2*sin(q2)*sin(q3)*sin(q4))/8 + (3^(1/2)*dq5*dqr1*cos(q4)*cos(q6)^2*sin(q2)*sin(q3)*sin(q5))/16 + (3^(1/2)*dq5*dqr1*cos(q5)*cos(q6)^2*sin(q2)*sin(q3)*sin(q4))/8 - (3^(1/2)*dq6*dqr1*cos(q4)*cos(q6)^2*sin(q2)*sin(q3)*sin(q5))/4 + (3^(1/2)*dq6*dqr1*cos(q5)*cos(q6)^2*sin(q2)*sin(q3)*sin(q4))/4 + dq1*dqr1*cos(q2)*cos(q4)*cos(q5)*sin(q2)*sin(q4)*sin(q5) + (dq1*dqr1*cos(q2)*cos(q4)*cos(q6)*sin(q2)*sin(q4)*sin(q6))/2 - (dq1*dqr1*cos(q2)*cos(q5)*cos(q6)*sin(q2)*sin(q5)*sin(q6))/2 - dq4*dqr1*cos(q3)*cos(q4)*cos(q5)*sin(q2)*sin(q4)*sin(q5) - (5*dq5*dqr1*cos(q3)*cos(q4)*cos(q5)*sin(q2)*sin(q4)*sin(q5))/4 - (dq4*dqr1*cos(q3)*cos(q4)*cos(q6)*sin(q2)*sin(q4)*sin(q6))/2 - (5*dq6*dqr1*cos(q3)*cos(q4)*cos(q5)*sin(q2)*sin(q4)*sin(q5))/8 - (5*dq5*dqr1*cos(q3)*cos(q4)*cos(q6)*sin(q2)*sin(q4)*sin(q6))/8 - (dq4*dqr1*cos(q3)*cos(q5)*cos(q6)*sin(q2)*sin(q5)*sin(q6))/4 + (dq6*dqr1*cos(q3)*cos(q4)*cos(q6)*sin(q2)*sin(q4)*sin(q6))/16 - (dq5*dqr1*cos(q3)*cos(q5)*cos(q6)*sin(q2)*sin(q5)*sin(q6))/2 - (5*3^(1/2)*dq4*dqr1*cos(q5)^2*cos(q6)^2*sin(q2)*sin(q3)*sin(q4))/16 - (5*3^(1/2)*dq5*dqr1*cos(q5)^2*cos(q6)^2*sin(q2)*sin(q3)*sin(q4))/8 - (3^(1/2)*dq6*dqr1*cos(q5)^2*cos(q6)^2*sin(q2)*sin(q3)*sin(q4))/2 - (3*dq1*dqr1*cos(q2)*cos(q4)*cos(q6)^2*sin(q2)*sin(q4)*sin(q5))/4 - 3*dq1*dqr1*cos(q2)*cos(q3)^2*cos(q6)*sin(q2)*sin(q5)*sin(q6) - (3*dq1*dqr1*cos(q2)*cos(q4)^2*cos(q6)*sin(q2)*sin(q5)*sin(q6))/4 + (3*dq4*dqr1*cos(q3)*cos(q4)*cos(q6)^2*sin(q2)*sin(q4)*sin(q5))/4 + (3*dq5*dqr1*cos(q3)*cos(q4)*cos(q6)^2*sin(q2)*sin(q4)*sin(q5))/16 + (3*dq4*dqr1*cos(q3)*cos(q4)^2*cos(q6)*sin(q2)*sin(q5)*sin(q6))/4 + (3*dq6*dqr1*cos(q3)*cos(q4)*cos(q6)^2*sin(q2)*sin(q4)*sin(q5))/4 + (3*dq5*dqr1*cos(q3)*cos(q4)^2*cos(q6)*sin(q2)*sin(q5)*sin(q6))/4 + (3*dq6*dqr1*cos(q3)*cos(q4)^2*cos(q6)*sin(q2)*sin(q5)*sin(q6))/4 - 3^(1/2)*dq1*dqr1*cos(q2)*cos(q3)*sin(q2)*sin(q3)*sin(q4) + (3^(1/2)*dq4*dqr1*cos(q4)*cos(q5)*sin(q2)*sin(q3)*sin(q5))/2 + (3^(1/2)*dq5*dqr1*cos(q4)*cos(q5)*sin(q2)*sin(q3)*sin(q5))/4 + (3^(1/2)*dq4*dqr1*cos(q4)*cos(q6)*sin(q2)*sin(q3)*sin(q6))/4 + (3^(1/2)*dq6*dqr1*cos(q4)*cos(q5)*sin(q2)*sin(q3)*sin(q5))/8 + (3^(1/2)*dq5*dqr1*cos(q4)*cos(q6)*sin(q2)*sin(q3)*sin(q6))/8 + (7*3^(1/2)*dq6*dqr1*cos(q4)*cos(q6)*sin(q2)*sin(q3)*sin(q6))/16 + 3^(1/2)*dq1*dqr1*cos(q2)*cos(q3)*cos(q5)^2*sin(q2)*sin(q3)*sin(q4) + (7*3^(1/2)*dq1*dqr1*cos(q2)*cos(q3)*cos(q6)^2*sin(q2)*sin(q3)*sin(q4))/4 - (5*3^(1/2)*dq4*dqr1*cos(q4)*cos(q5)*cos(q6)^2*sin(q2)*sin(q3)*sin(q5))/8 - (3^(1/2)*dq4*dqr1*cos(q4)*cos(q5)^2*cos(q6)*sin(q2)*sin(q3)*sin(q6))/2 - (5*3^(1/2)*dq5*dqr1*cos(q4)*cos(q5)*cos(q6)^2*sin(q2)*sin(q3)*sin(q5))/16 - (3^(1/2)*dq5*dqr1*cos(q4)*cos(q5)^2*cos(q6)*sin(q2)*sin(q3)*sin(q6))/4 - (3^(1/2)*dq6*dqr1*cos(q4)*cos(q5)*cos(q6)^2*sin(q2)*sin(q3)*sin(q5))/4 - (5*3^(1/2)*dq6*dqr1*cos(q4)*cos(q5)^2*cos(q6)*sin(q2)*sin(q3)*sin(q6))/16 - (3*dq1*dqr1*cos(q2)*cos(q4)*cos(q5)*cos(q6)*sin(q2)*sin(q4)*sin(q6))/2 + (3*dq4*dqr1*cos(q3)*cos(q4)*cos(q5)*cos(q6)*sin(q2)*sin(q4)*sin(q6))/2 + (3*dq5*dqr1*cos(q3)*cos(q4)*cos(q5)*cos(q6)*sin(q2)*sin(q4)*sin(q6))/8 + (3*dq6*dqr1*cos(q3)*cos(q4)*cos(q5)*cos(q6)*sin(q2)*sin(q4)*sin(q6))/8 - 2*dq1*dqr1*cos(q2)*cos(q3)^2*cos(q4)*cos(q5)*sin(q2)*sin(q4)*sin(q5) - dq1*dqr1*cos(q2)*cos(q3)^2*cos(q4)*cos(q6)*sin(q2)*sin(q4)*sin(q6) - (5*dq1*dqr1*cos(q2)*cos(q4)*cos(q5)*cos(q6)^2*sin(q2)*sin(q4)*sin(q5))/4 - dq1*dqr1*cos(q2)*cos(q4)*cos(q5)^2*cos(q6)*sin(q2)*sin(q4)*sin(q6) + dq1*dqr1*cos(q2)*cos(q3)^2*cos(q5)*cos(q6)*sin(q2)*sin(q5)*sin(q6) - (5*dq1*dqr1*cos(q2)*cos(q4)^2*cos(q5)*cos(q6)*sin(q2)*sin(q5)*sin(q6))/4 + (5*dq4*dqr1*cos(q3)*cos(q4)*cos(q5)*cos(q6)^2*sin(q2)*sin(q4)*sin(q5))/4 + dq4*dqr1*cos(q3)*cos(q4)*cos(q5)^2*cos(q6)*sin(q2)*sin(q4)*sin(q6) + (25*dq5*dqr1*cos(q3)*cos(q4)*cos(q5)*cos(q6)^2*sin(q2)*sin(q4)*sin(q5))/16 + (5*dq4*dqr1*cos(q3)*cos(q4)^2*cos(q5)*cos(q6)*sin(q2)*sin(q5)*sin(q6))/4 + (5*dq5*dqr1*cos(q3)*cos(q4)*cos(q5)^2*cos(q6)*sin(q2)*sin(q4)*sin(q6))/4 + (5*dq6*dqr1*cos(q3)*cos(q4)*cos(q5)*cos(q6)^2*sin(q2)*sin(q4)*sin(q5))/4 + dq5*dqr1*cos(q3)*cos(q4)^2*cos(q5)*cos(q6)*sin(q2)*sin(q5)*sin(q6) + (25*dq6*dqr1*cos(q3)*cos(q4)*cos(q5)^2*cos(q6)*sin(q2)*sin(q4)*sin(q6))/16 + (5*dq6*dqr1*cos(q3)*cos(q4)^2*cos(q5)*cos(q6)*sin(q2)*sin(q5)*sin(q6))/4 + (3^(1/2)*dq4*dqr1*cos(q4)*cos(q5)*cos(q6)*sin(q2)*sin(q3)*sin(q6))/4 + (3^(1/2)*dq5*dqr1*cos(q4)*cos(q5)*cos(q6)*sin(q2)*sin(q3)*sin(q6))/8 - (3^(1/2)*dq6*dqr1*cos(q4)*cos(q5)*cos(q6)*sin(q2)*sin(q3)*sin(q6))/8 + (3^(1/2)*dq4*dqr1*cos(q6)*sin(q2)*sin(q3)*sin(q4)*sin(q5)*sin(q6))/4 - (3^(1/2)*dq5*dqr1*cos(q6)*sin(q2)*sin(q3)*sin(q4)*sin(q5)*sin(q6))/4 - (3^(1/2)*dq6*dqr1*cos(q6)*sin(q2)*sin(q3)*sin(q4)*sin(q5)*sin(q6))/8 + (3*dq1*dqr1*cos(q2)*cos(q3)^2*cos(q4)*cos(q6)^2*sin(q2)*sin(q4)*sin(q5))/2 + (3*dq1*dqr1*cos(q2)*cos(q3)^2*cos(q4)^2*cos(q6)*sin(q2)*sin(q5)*sin(q6))/2 - (5*3^(1/2)*dq1*dqr1*cos(q2)*cos(q3)*cos(q5)^2*cos(q6)^2*sin(q2)*sin(q3)*sin(q4))/4 + 3*dq1*dqr1*cos(q2)*cos(q3)^2*cos(q4)*cos(q5)*cos(q6)*sin(q2)*sin(q4)*sin(q6) + 2*3^(1/2)*dq1*dqr1*cos(q2)*cos(q3)*cos(q4)*cos(q5)*sin(q2)*sin(q3)*sin(q5) + 3^(1/2)*dq1*dqr1*cos(q2)*cos(q3)*cos(q4)*cos(q6)*sin(q2)*sin(q3)*sin(q6) + (3^(1/2)*dq4*dqr1*cos(q5)*cos(q6)*sin(q2)*sin(q3)*sin(q4)*sin(q5)*sin(q6))/4 + (3^(1/2)*dq5*dqr1*cos(q5)*cos(q6)*sin(q2)*sin(q3)*sin(q4)*sin(q5)*sin(q6))/2 + (5*3^(1/2)*dq6*dqr1*cos(q5)*cos(q6)*sin(q2)*sin(q3)*sin(q4)*sin(q5)*sin(q6))/8 + (5*dq1*dqr1*cos(q2)*cos(q3)^2*cos(q4)*cos(q5)*cos(q6)^2*sin(q2)*sin(q4)*sin(q5))/2 + 2*dq1*dqr1*cos(q2)*cos(q3)^2*cos(q4)*cos(q5)^2*cos(q6)*sin(q2)*sin(q4)*sin(q6) + (5*dq1*dqr1*cos(q2)*cos(q3)^2*cos(q4)^2*cos(q5)*cos(q6)*sin(q2)*sin(q5)*sin(q6))/2 + (3^(1/2)*dq1*dqr1*cos(q2)*cos(q3)*cos(q4)*cos(q6)^2*sin(q2)*sin(q3)*sin(q5))/2 - (3^(1/2)*dq1*dqr1*cos(q2)*cos(q3)*cos(q5)*cos(q6)^2*sin(q2)*sin(q3)*sin(q4))/2 + 3^(1/2)*dq1*dqr1*cos(q2)*cos(q3)*cos(q4)*cos(q5)*cos(q6)*sin(q2)*sin(q3)*sin(q6) + 3^(1/2)*dq1*dqr1*cos(q2)*cos(q3)*cos(q6)*sin(q2)*sin(q3)*sin(q4)*sin(q5)*sin(q6) - (5*3^(1/2)*dq1*dqr1*cos(q2)*cos(q3)*cos(q4)*cos(q5)*cos(q6)^2*sin(q2)*sin(q3)*sin(q5))/2 - 2*3^(1/2)*dq1*dqr1*cos(q2)*cos(q3)*cos(q4)*cos(q5)^2*cos(q6)*sin(q2)*sin(q3)*sin(q6) + 3^(1/2)*dq1*dqr1*cos(q2)*cos(q3)*cos(q5)*cos(q6)*sin(q2)*sin(q3)*sin(q4)*sin(q5)*sin(q6);
Y2_20_2=(dq4*dqr1*cos(q3)*sin(q2))/4 + (dq5*dqr1*cos(q3)*sin(q2))/2 + (dq6*dqr1*cos(q3)*sin(q2))/4 - dq1*dqr1*cos(q2)*cos(q3)^2*sin(q2) + (dq1*dqr1*cos(q2)*cos(q4)^2*sin(q2))/4 - (dq1*dqr1*cos(q2)*cos(q5)^2*sin(q2))/2 - (7*dq1*dqr1*cos(q2)*cos(q6)^2*sin(q2))/8 - (dq4*dqr1*cos(q3)*cos(q4)^2*sin(q2))/4 - (dq4*dqr1*cos(q3)*cos(q5)^2*sin(q2))/4 - (dq5*dqr1*cos(q3)*cos(q4)^2*sin(q2))/2 + (5*dq4*dqr1*cos(q3)*cos(q6)^2*sin(q2))/16 - (dq5*dqr1*cos(q3)*cos(q5)^2*sin(q2))/2 - (dq6*dqr1*cos(q3)*cos(q4)^2*sin(q2))/4 - (dq5*dqr1*cos(q3)*cos(q6)^2*sin(q2))/2 - (dq6*dqr1*cos(q3)*cos(q5)^2*sin(q2))/4 - (dq6*dqr1*cos(q3)*cos(q6)^2*sin(q2))/4 - (dq1*dqr1*cos(q2)*cos(q3)^2*cos(q4)^2*sin(q2))/2 + dq1*dqr1*cos(q2)*cos(q3)^2*cos(q5)^2*sin(q2) + (7*dq1*dqr1*cos(q2)*cos(q3)^2*cos(q6)^2*sin(q2))/4 - (5*dq1*dqr1*cos(q2)*cos(q4)^2*cos(q5)^2*sin(q2))/4 + (dq1*dqr1*cos(q2)*cos(q4)^2*cos(q6)^2*sin(q2))/16 + (5*dq1*dqr1*cos(q2)*cos(q5)^2*cos(q6)^2*sin(q2))/8 + (5*dq4*dqr1*cos(q3)*cos(q4)^2*cos(q5)^2*sin(q2))/4 - (dq4*dqr1*cos(q3)*cos(q4)^2*cos(q6)^2*sin(q2))/16 + dq5*dqr1*cos(q3)*cos(q4)^2*cos(q5)^2*sin(q2) + (5*dq4*dqr1*cos(q3)*cos(q5)^2*cos(q6)^2*sin(q2))/16 + (5*dq5*dqr1*cos(q3)*cos(q4)^2*cos(q6)^2*sin(q2))/8 + (dq6*dqr1*cos(q3)*cos(q4)^2*cos(q5)^2*sin(q2))/2 + (5*dq5*dqr1*cos(q3)*cos(q5)^2*cos(q6)^2*sin(q2))/8 + (dq6*dqr1*cos(q3)*cos(q4)^2*cos(q6)^2*sin(q2))/2 + (dq6*dqr1*cos(q3)*cos(q5)^2*cos(q6)^2*sin(q2))/2 - (3*dq1*dqr1*cos(q2)*cos(q5)*cos(q6)^2*sin(q2))/4 + (3*dq4*dqr1*cos(q3)*cos(q5)*cos(q6)^2*sin(q2))/8 + (3*dq6*dqr1*cos(q3)*cos(q4)^2*cos(q5)*sin(q2))/4 + (3*dq5*dqr1*cos(q3)*cos(q5)*cos(q6)^2*sin(q2))/8 + (3*dq6*dqr1*cos(q3)*cos(q5)*cos(q6)^2*sin(q2))/4 + (3*dq1*dqr1*cos(q2)*cos(q3)^2*cos(q5)*cos(q6)^2*sin(q2))/2 + (3*dq1*dqr1*cos(q2)*cos(q4)^2*cos(q5)*cos(q6)^2*sin(q2))/8 - (3*dq4*dqr1*cos(q3)*cos(q4)^2*cos(q5)*cos(q6)^2*sin(q2))/8 - (3*dq5*dqr1*cos(q3)*cos(q4)^2*cos(q5)*cos(q6)^2*sin(q2))/8 - (3*dq6*dqr1*cos(q3)*cos(q4)^2*cos(q5)*cos(q6)^2*sin(q2))/2 + (5*dq1*dqr1*cos(q2)*cos(q3)^2*cos(q4)^2*cos(q5)^2*sin(q2))/2 - (dq1*dqr1*cos(q2)*cos(q3)^2*cos(q4)^2*cos(q6)^2*sin(q2))/8 - (5*dq1*dqr1*cos(q2)*cos(q3)^2*cos(q5)^2*cos(q6)^2*sin(q2))/4 + (25*dq1*dqr1*cos(q2)*cos(q4)^2*cos(q5)^2*cos(q6)^2*sin(q2))/16 - (25*dq4*dqr1*cos(q3)*cos(q4)^2*cos(q5)^2*cos(q6)^2*sin(q2))/16 - (5*dq5*dqr1*cos(q3)*cos(q4)^2*cos(q5)^2*cos(q6)^2*sin(q2))/4 - dq6*dqr1*cos(q3)*cos(q4)^2*cos(q5)^2*cos(q6)^2*sin(q2) + (3*dq6*dqr1*cos(q2)*cos(q4)*sin(q3)*sin(q4)*sin(q5))/8 + (3*dq4*dqr1*cos(q2)*cos(q6)*sin(q3)*sin(q5)*sin(q6))/4 - (3*dq4*dqr1*cos(q3)*cos(q6)*sin(q2)*sin(q5)*sin(q6))/4 + (3*dq5*dqr1*cos(q2)*cos(q6)*sin(q3)*sin(q5)*sin(q6))/4 - (3*dq5*dqr1*cos(q3)*cos(q6)*sin(q2)*sin(q5)*sin(q6))/4 - (3*dq6*dqr1*cos(q3)*cos(q6)*sin(q2)*sin(q5)*sin(q6))/8 - (3*dq1*dqr1*cos(q2)*cos(q3)^2*cos(q4)^2*cos(q5)*cos(q6)^2*sin(q2))/4 - dq1*dqr1*cos(q3)*cos(q4)*cos(q5)*sin(q3)*sin(q4)*sin(q5) - (dq1*dqr1*cos(q3)*cos(q4)*cos(q6)*sin(q3)*sin(q4)*sin(q6))/2 + dq4*dqr1*cos(q2)*cos(q4)*cos(q5)*sin(q3)*sin(q4)*sin(q5) + (5*dq5*dqr1*cos(q2)*cos(q4)*cos(q5)*sin(q3)*sin(q4)*sin(q5))/4 + (dq4*dqr1*cos(q2)*cos(q4)*cos(q6)*sin(q3)*sin(q4)*sin(q6))/2 + (5*dq6*dqr1*cos(q2)*cos(q4)*cos(q5)*sin(q3)*sin(q4)*sin(q5))/8 + (5*dq5*dqr1*cos(q2)*cos(q4)*cos(q6)*sin(q3)*sin(q4)*sin(q6))/8 + (dq4*dqr1*cos(q2)*cos(q5)*cos(q6)*sin(q3)*sin(q5)*sin(q6))/4 - (dq6*dqr1*cos(q2)*cos(q4)*cos(q6)*sin(q3)*sin(q4)*sin(q6))/16 + (dq5*dqr1*cos(q2)*cos(q5)*cos(q6)*sin(q3)*sin(q5)*sin(q6))/2 + (5*dq6*dqr1*cos(q2)*cos(q5)*cos(q6)*sin(q3)*sin(q5)*sin(q6))/8 - (5*dq6*dqr1*cos(q3)*cos(q5)*cos(q6)*sin(q2)*sin(q5)*sin(q6))/8 - (25*dq1*dqr1*cos(q2)*cos(q3)^2*cos(q4)^2*cos(q5)^2*cos(q6)^2*sin(q2))/8 + (3*dq1*dqr1*cos(q3)*cos(q4)*cos(q6)^2*sin(q3)*sin(q4)*sin(q5))/4 + 3*dq1*dqr1*cos(q2)^2*cos(q3)*cos(q6)*sin(q3)*sin(q5)*sin(q6) - (3*dq4*dqr1*cos(q2)*cos(q4)*cos(q6)^2*sin(q3)*sin(q4)*sin(q5))/4 - (3*dq5*dqr1*cos(q2)*cos(q4)*cos(q6)^2*sin(q3)*sin(q4)*sin(q5))/16 - (3*dq4*dqr1*cos(q2)*cos(q4)^2*cos(q6)*sin(q3)*sin(q5)*sin(q6))/4 - (3*dq6*dqr1*cos(q2)*cos(q4)*cos(q6)^2*sin(q3)*sin(q4)*sin(q5))/4 - (3*dq5*dqr1*cos(q2)*cos(q4)^2*cos(q6)*sin(q3)*sin(q5)*sin(q6))/4 - (3*dq6*dqr1*cos(q2)*cos(q4)^2*cos(q6)*sin(q3)*sin(q5)*sin(q6))/4 + (3*dq1*dqr1*cos(q3)*cos(q4)*cos(q5)*cos(q6)*sin(q3)*sin(q4)*sin(q6))/2 - (3*dq4*dqr1*cos(q2)*cos(q4)*cos(q5)*cos(q6)*sin(q3)*sin(q4)*sin(q6))/2 - (3*dq5*dqr1*cos(q2)*cos(q4)*cos(q5)*cos(q6)*sin(q3)*sin(q4)*sin(q6))/8 - (3*dq6*dqr1*cos(q2)*cos(q4)*cos(q5)*cos(q6)*sin(q3)*sin(q4)*sin(q6))/8 + 2*dq1*dqr1*cos(q2)^2*cos(q3)*cos(q4)*cos(q5)*sin(q3)*sin(q4)*sin(q5) + dq1*dqr1*cos(q2)^2*cos(q3)*cos(q4)*cos(q6)*sin(q3)*sin(q4)*sin(q6) + (5*dq1*dqr1*cos(q3)*cos(q4)*cos(q5)*cos(q6)^2*sin(q3)*sin(q4)*sin(q5))/4 - dq1*dqr1*cos(q2)^2*cos(q3)*cos(q5)*cos(q6)*sin(q3)*sin(q5)*sin(q6) + dq1*dqr1*cos(q3)*cos(q4)*cos(q5)^2*cos(q6)*sin(q3)*sin(q4)*sin(q6) - (5*dq4*dqr1*cos(q2)*cos(q4)*cos(q5)*cos(q6)^2*sin(q3)*sin(q4)*sin(q5))/4 - dq4*dqr1*cos(q2)*cos(q4)*cos(q5)^2*cos(q6)*sin(q3)*sin(q4)*sin(q6) - (25*dq5*dqr1*cos(q2)*cos(q4)*cos(q5)*cos(q6)^2*sin(q3)*sin(q4)*sin(q5))/16 - (5*dq4*dqr1*cos(q2)*cos(q4)^2*cos(q5)*cos(q6)*sin(q3)*sin(q5)*sin(q6))/4 - (5*dq5*dqr1*cos(q2)*cos(q4)*cos(q5)^2*cos(q6)*sin(q3)*sin(q4)*sin(q6))/4 - (5*dq6*dqr1*cos(q2)*cos(q4)*cos(q5)*cos(q6)^2*sin(q3)*sin(q4)*sin(q5))/4 - dq5*dqr1*cos(q2)*cos(q4)^2*cos(q5)*cos(q6)*sin(q3)*sin(q5)*sin(q6) - (25*dq6*dqr1*cos(q2)*cos(q4)*cos(q5)^2*cos(q6)*sin(q3)*sin(q4)*sin(q6))/16 - (5*dq6*dqr1*cos(q2)*cos(q4)^2*cos(q5)*cos(q6)*sin(q3)*sin(q5)*sin(q6))/4 - (3*dq1*dqr1*cos(q2)^2*cos(q3)*cos(q4)*cos(q6)^2*sin(q3)*sin(q4)*sin(q5))/2 - (3*dq1*dqr1*cos(q2)^2*cos(q3)*cos(q4)^2*cos(q6)*sin(q3)*sin(q5)*sin(q6))/2 - 3*dq1*dqr1*cos(q2)^2*cos(q3)*cos(q4)*cos(q5)*cos(q6)*sin(q3)*sin(q4)*sin(q6) - (5*dq1*dqr1*cos(q2)^2*cos(q3)*cos(q4)*cos(q5)*cos(q6)^2*sin(q3)*sin(q4)*sin(q5))/2 - 2*dq1*dqr1*cos(q2)^2*cos(q3)*cos(q4)*cos(q5)^2*cos(q6)*sin(q3)*sin(q4)*sin(q6) - (5*dq1*dqr1*cos(q2)^2*cos(q3)*cos(q4)^2*cos(q5)*cos(q6)*sin(q3)*sin(q5)*sin(q6))/2;
Y2_20_3=dq1*dqr1*cos(q2)^2*cos(q3)*sin(q3) - (dq5*dqr1*cos(q2)*sin(q3))/2 - (dq6*dqr1*cos(q2)*sin(q3))/4 - (dq4*dqr1*cos(q2)*sin(q3))/4 - (dq1*dqr1*cos(q3)*cos(q4)^2*sin(q3))/4 + (dq1*dqr1*cos(q3)*cos(q5)^2*sin(q3))/2 + (7*dq1*dqr1*cos(q3)*cos(q6)^2*sin(q3))/8 + (dq4*dqr1*cos(q2)*cos(q4)^2*sin(q3))/4 + (dq4*dqr1*cos(q2)*cos(q5)^2*sin(q3))/4 + (dq5*dqr1*cos(q2)*cos(q4)^2*sin(q3))/2 - (5*dq4*dqr1*cos(q2)*cos(q6)^2*sin(q3))/16 + (dq5*dqr1*cos(q2)*cos(q5)^2*sin(q3))/2 + (dq6*dqr1*cos(q2)*cos(q4)^2*sin(q3))/4 + (dq5*dqr1*cos(q2)*cos(q6)^2*sin(q3))/2 + (dq6*dqr1*cos(q2)*cos(q5)^2*sin(q3))/4 + (dq6*dqr1*cos(q2)*cos(q6)^2*sin(q3))/4 + (3^(1/2)*dq1*dqr1*cos(q2)^2*sin(q4))/2 + (3^(1/2)*dq1*dqr1*cos(q3)^2*sin(q4))/2 - (3^(1/2)*dq4*dqr1*cos(q2)*cos(q3)*sin(q4))/4 - (3^(1/2)*dq5*dqr1*cos(q2)*cos(q3)*sin(q4))/2 - (3^(1/2)*dq6*dqr1*cos(q2)*cos(q3)*sin(q4))/4 + (dq1*dqr1*cos(q2)^2*cos(q3)*cos(q4)^2*sin(q3))/2 - dq1*dqr1*cos(q2)^2*cos(q3)*cos(q5)^2*sin(q3) - (7*dq1*dqr1*cos(q2)^2*cos(q3)*cos(q6)^2*sin(q3))/4 + (5*dq1*dqr1*cos(q3)*cos(q4)^2*cos(q5)^2*sin(q3))/4 - (dq1*dqr1*cos(q3)*cos(q4)^2*cos(q6)^2*sin(q3))/16 - (5*dq1*dqr1*cos(q3)*cos(q5)^2*cos(q6)^2*sin(q3))/8 - (5*dq4*dqr1*cos(q2)*cos(q4)^2*cos(q5)^2*sin(q3))/4 + (dq4*dqr1*cos(q2)*cos(q4)^2*cos(q6)^2*sin(q3))/16 - dq5*dqr1*cos(q2)*cos(q4)^2*cos(q5)^2*sin(q3) - (5*dq4*dqr1*cos(q2)*cos(q5)^2*cos(q6)^2*sin(q3))/16 - (5*dq5*dqr1*cos(q2)*cos(q4)^2*cos(q6)^2*sin(q3))/8 - (dq6*dqr1*cos(q2)*cos(q4)^2*cos(q5)^2*sin(q3))/2 - (5*dq5*dqr1*cos(q2)*cos(q5)^2*cos(q6)^2*sin(q3))/8 - (dq6*dqr1*cos(q2)*cos(q4)^2*cos(q6)^2*sin(q3))/2 - (dq6*dqr1*cos(q2)*cos(q5)^2*cos(q6)^2*sin(q3))/2 - 3^(1/2)*dq1*dqr1*cos(q2)^2*cos(q3)^2*sin(q4) - (3^(1/2)*dq1*dqr1*cos(q2)^2*cos(q5)^2*sin(q4))/2 - (7*3^(1/2)*dq1*dqr1*cos(q2)^2*cos(q6)^2*sin(q4))/8 - (3^(1/2)*dq1*dqr1*cos(q3)^2*cos(q5)^2*sin(q4))/2 - (7*3^(1/2)*dq1*dqr1*cos(q3)^2*cos(q6)^2*sin(q4))/8 - (5*3^(1/2)*dq1*dqr1*cos(q5)^2*cos(q6)^2*sin(q4))/16 + (3*dq1*dqr1*cos(q3)*cos(q5)*cos(q6)^2*sin(q3))/4 - (3*dq4*dqr1*cos(q2)*cos(q5)*cos(q6)^2*sin(q3))/8 - (3*dq6*dqr1*cos(q2)*cos(q4)^2*cos(q5)*sin(q3))/4 - (3*dq5*dqr1*cos(q2)*cos(q5)*cos(q6)^2*sin(q3))/8 - (3*dq6*dqr1*cos(q2)*cos(q5)*cos(q6)^2*sin(q3))/4 + 3^(1/2)*dq1*dqr1*cos(q2)^2*cos(q3)^2*cos(q5)^2*sin(q4) + (7*3^(1/2)*dq1*dqr1*cos(q2)^2*cos(q3)^2*cos(q6)^2*sin(q4))/4 + (5*3^(1/2)*dq1*dqr1*cos(q2)^2*cos(q5)^2*cos(q6)^2*sin(q4))/8 + (5*3^(1/2)*dq1*dqr1*cos(q3)^2*cos(q5)^2*cos(q6)^2*sin(q4))/8 + (3^(1/2)*dq1*dqr1*cos(q6)*sin(q4)*sin(q5)*sin(q6))/4 - (3*dq1*dqr1*cos(q2)^2*cos(q3)*cos(q5)*cos(q6)^2*sin(q3))/2 - (3*dq1*dqr1*cos(q3)*cos(q4)^2*cos(q5)*cos(q6)^2*sin(q3))/8 + (3*dq4*dqr1*cos(q2)*cos(q4)^2*cos(q5)*cos(q6)^2*sin(q3))/8 + (3*dq5*dqr1*cos(q2)*cos(q4)^2*cos(q5)*cos(q6)^2*sin(q3))/8 + (3*dq6*dqr1*cos(q2)*cos(q4)^2*cos(q5)*cos(q6)^2*sin(q3))/2 + (3^(1/2)*dq4*dqr1*cos(q2)*cos(q3)*cos(q5)^2*sin(q4))/4 + (7*3^(1/2)*dq4*dqr1*cos(q2)*cos(q3)*cos(q6)^2*sin(q4))/16 + (3^(1/2)*dq5*dqr1*cos(q2)*cos(q3)*cos(q5)^2*sin(q4))/2 + (3^(1/2)*dq5*dqr1*cos(q2)*cos(q3)*cos(q6)^2*sin(q4))/2 + (3^(1/2)*dq6*dqr1*cos(q2)*cos(q3)*cos(q5)^2*sin(q4))/4 + (3^(1/2)*dq6*dqr1*cos(q2)*cos(q3)*cos(q6)^2*sin(q4))/4 - (5*dq1*dqr1*cos(q2)^2*cos(q3)*cos(q4)^2*cos(q5)^2*sin(q3))/2 + (dq1*dqr1*cos(q2)^2*cos(q3)*cos(q4)^2*cos(q6)^2*sin(q3))/8 + (5*dq1*dqr1*cos(q2)^2*cos(q3)*cos(q5)^2*cos(q6)^2*sin(q3))/4 - (25*dq1*dqr1*cos(q3)*cos(q4)^2*cos(q5)^2*cos(q6)^2*sin(q3))/16 + (25*dq4*dqr1*cos(q2)*cos(q4)^2*cos(q5)^2*cos(q6)^2*sin(q3))/16 + (5*dq5*dqr1*cos(q2)*cos(q4)^2*cos(q5)^2*cos(q6)^2*sin(q3))/4 + dq6*dqr1*cos(q2)*cos(q4)^2*cos(q5)^2*cos(q6)^2*sin(q3) - (3*dq1*dqr1*cos(q3)*cos(q6)*sin(q3)*sin(q5)*sin(q6))/2 + (3*dq6*dqr1*cos(q2)*cos(q6)*sin(q3)*sin(q5)*sin(q6))/8 + (3^(1/2)*dq1*dqr1*cos(q2)^2*cos(q5)*cos(q6)^2*sin(q4))/4 + (3^(1/2)*dq1*dqr1*cos(q3)^2*cos(q5)*cos(q6)^2*sin(q4))/4 - (3^(1/2)*dq4*dqr1*cos(q2)*cos(q3)*cos(q5)*cos(q6)^2*sin(q4))/8 + (3^(1/2)*dq5*dqr1*cos(q2)*cos(q3)*cos(q5)*cos(q6)^2*sin(q4))/8 + (3^(1/2)*dq6*dqr1*cos(q2)*cos(q3)*cos(q5)*cos(q6)^2*sin(q4))/4 - (5*3^(1/2)*dq1*dqr1*cos(q2)^2*cos(q3)^2*cos(q5)^2*cos(q6)^2*sin(q4))/4 - (3^(1/2)*dq1*dqr1*cos(q2)^2*cos(q6)*sin(q4)*sin(q5)*sin(q6))/2 - (3^(1/2)*dq1*dqr1*cos(q3)^2*cos(q6)*sin(q4)*sin(q5)*sin(q6))/2 + (3*dq1*dqr1*cos(q2)^2*cos(q3)*cos(q4)^2*cos(q5)*cos(q6)^2*sin(q3))/4 + (dq1*dqr1*cos(q3)*cos(q5)*cos(q6)*sin(q3)*sin(q5)*sin(q6))/2 - (5*3^(1/2)*dq4*dqr1*cos(q2)*cos(q3)*cos(q5)^2*cos(q6)^2*sin(q4))/16 - (5*3^(1/2)*dq5*dqr1*cos(q2)*cos(q3)*cos(q5)^2*cos(q6)^2*sin(q4))/8 - (3^(1/2)*dq6*dqr1*cos(q2)*cos(q3)*cos(q5)^2*cos(q6)^2*sin(q4))/2 + (25*dq1*dqr1*cos(q2)^2*cos(q3)*cos(q4)^2*cos(q5)^2*cos(q6)^2*sin(q3))/8 + (3*dq1*dqr1*cos(q3)*cos(q4)^2*cos(q6)*sin(q3)*sin(q5)*sin(q6))/4 - (3^(1/2)*dq1*dqr1*cos(q2)^2*cos(q3)^2*cos(q5)*cos(q6)^2*sin(q4))/2 + (3^(1/2)*dq1*dqr1*cos(q5)*cos(q6)*sin(q4)*sin(q5)*sin(q6))/4 - (3^(1/2)*dq1*dqr1*cos(q2)^2*cos(q5)*cos(q6)*sin(q4)*sin(q5)*sin(q6))/2 - (3^(1/2)*dq1*dqr1*cos(q3)^2*cos(q5)*cos(q6)*sin(q4)*sin(q5)*sin(q6))/2 + 3^(1/2)*dq1*dqr1*cos(q2)^2*cos(q3)^2*cos(q6)*sin(q4)*sin(q5)*sin(q6) + (5*dq1*dqr1*cos(q3)*cos(q4)^2*cos(q5)*cos(q6)*sin(q3)*sin(q5)*sin(q6))/4 + (3^(1/2)*dq4*dqr1*cos(q2)*cos(q3)*cos(q6)*sin(q4)*sin(q5)*sin(q6))/4 - (3^(1/2)*dq5*dqr1*cos(q2)*cos(q3)*cos(q6)*sin(q4)*sin(q5)*sin(q6))/4 - (3^(1/2)*dq6*dqr1*cos(q2)*cos(q3)*cos(q6)*sin(q4)*sin(q5)*sin(q6))/8 + 3^(1/2)*dq1*dqr1*cos(q2)^2*cos(q3)^2*cos(q5)*cos(q6)*sin(q4)*sin(q5)*sin(q6) + (3^(1/2)*dq4*dqr1*cos(q2)*cos(q3)*cos(q5)*cos(q6)*sin(q4)*sin(q5)*sin(q6))/4 + (3^(1/2)*dq5*dqr1*cos(q2)*cos(q3)*cos(q5)*cos(q6)*sin(q4)*sin(q5)*sin(q6))/2 + (5*3^(1/2)*dq6*dqr1*cos(q2)*cos(q3)*cos(q5)*cos(q6)*sin(q4)*sin(q5)*sin(q6))/8;
Y2_20_4=(dq1*dqr1*sin(2*q2))/4 - (dq1*dqr1*sin(2*q3))/4 + (dq4*dqr2*sin(2*q4))/8 + (dq4*dqr2*sin(2*q5))/4 + (dq5*dqr2*sin(2*q4))/4 + (dq4*dqr2*sin(2*q6))/8 + (dq5*dqr2*sin(2*q5))/2 - (3*dq4*dqr2*cos(q6)^2*sin(q5))/8 - (3*dq6*dqr2*cos(q4)^2*sin(q5))/8 - (3^(1/2)*dq1*dqr1*sin(q4))/4 - (5*dq4*dqr2*cos(q4)*cos(q5)^2*sin(q4))/4 + (dq4*dqr2*cos(q4)*cos(q6)^2*sin(q4))/16 - dq4*dqr2*cos(q4)^2*cos(q5)*sin(q5) - dq5*dqr2*cos(q4)*cos(q5)^2*sin(q4) - (5*dq5*dqr2*cos(q4)*cos(q6)^2*sin(q4))/8 - (5*dq5*dqr2*cos(q4)^2*cos(q5)*sin(q5))/4 - (dq6*dqr2*cos(q4)*cos(q5)^2*sin(q4))/2 - (5*dq4*dqr2*cos(q5)*cos(q6)^2*sin(q5))/8 - (dq4*dqr2*cos(q4)^2*cos(q6)*sin(q6))/2 - (dq6*dqr2*cos(q4)*cos(q6)^2*sin(q4))/2 - (5*dq6*dqr2*cos(q4)^2*cos(q5)*sin(q5))/8 - (dq4*dqr2*cos(q5)^2*cos(q6)*sin(q6))/2 - (5*dq5*dqr2*cos(q5)*cos(q6)^2*sin(q5))/4 - (5*dq5*dqr2*cos(q4)^2*cos(q6)*sin(q6))/8 - dq5*dqr2*cos(q5)^2*cos(q6)*sin(q6) - dq6*dqr2*cos(q5)*cos(q6)^2*sin(q5) + (dq6*dqr2*cos(q4)^2*cos(q6)*sin(q6))/16 - (5*dq6*dqr2*cos(q5)^2*cos(q6)*sin(q6))/4 + (3*dq4*dqr2*cos(q4)^2*cos(q6)^2*sin(q5))/4 + (3*dq5*dqr2*cos(q4)^2*cos(q6)^2*sin(q5))/16 + (3*dq6*dqr2*cos(q4)^2*cos(q6)^2*sin(q5))/4 + (3^(1/2)*dq1*dqr1*cos(q5)^2*sin(q4))/4 + (7*3^(1/2)*dq1*dqr1*cos(q6)^2*sin(q4))/16 - (3*dq6*dqr2*cos(q4)*cos(q5)*sin(q4))/4 - (3*dq4*dqr2*cos(q5)*cos(q6)*sin(q6))/4 + (3^(1/2)*dq1*dqr1*cos(q4)*cos(q5)*sin(q5))/2 + (3^(1/2)*dq1*dqr1*cos(q4)*cos(q6)*sin(q6))/4 + (25*dq4*dqr2*cos(q4)*cos(q5)^2*cos(q6)^2*sin(q4))/16 + (5*dq4*dqr2*cos(q4)^2*cos(q5)*cos(q6)^2*sin(q5))/4 + (5*dq5*dqr2*cos(q4)*cos(q5)^2*cos(q6)^2*sin(q4))/4 + dq4*dqr2*cos(q4)^2*cos(q5)^2*cos(q6)*sin(q6) + (25*dq5*dqr2*cos(q4)^2*cos(q5)*cos(q6)^2*sin(q5))/16 + dq6*dqr2*cos(q4)*cos(q5)^2*cos(q6)^2*sin(q4) + (5*dq5*dqr2*cos(q4)^2*cos(q5)^2*cos(q6)*sin(q6))/4 + (5*dq6*dqr2*cos(q4)^2*cos(q5)*cos(q6)^2*sin(q5))/4 + (25*dq6*dqr2*cos(q4)^2*cos(q5)^2*cos(q6)*sin(q6))/16 + (3^(1/2)*dq1*dqr1*cos(q4)*cos(q6)^2*sin(q5))/8 - (3^(1/2)*dq1*dqr1*cos(q5)*cos(q6)^2*sin(q4))/8 + (3*dq4*dqr2*cos(q4)*cos(q5)*cos(q6)^2*sin(q4))/8 + (3*dq5*dqr2*cos(q4)*cos(q5)*cos(q6)^2*sin(q4))/8 + (3*dq4*dqr2*cos(q4)^2*cos(q5)*cos(q6)*sin(q6))/2 + (3*dq6*dqr2*cos(q4)*cos(q5)*cos(q6)^2*sin(q4))/2 + (3*dq5*dqr2*cos(q4)^2*cos(q5)*cos(q6)*sin(q6))/8 + (3*dq6*dqr2*cos(q4)^2*cos(q5)*cos(q6)*sin(q6))/8 - 3^(1/2)*dq1*dqr1*cos(q2)^2*cos(q4)*cos(q5)*sin(q5) - 3^(1/2)*dq1*dqr1*cos(q3)^2*cos(q4)*cos(q5)*sin(q5) - (3^(1/2)*dq1*dqr1*cos(q2)^2*cos(q4)*cos(q6)*sin(q6))/2 - (3^(1/2)*dq1*dqr1*cos(q3)^2*cos(q4)*cos(q6)*sin(q6))/2 - (5*3^(1/2)*dq1*dqr1*cos(q4)*cos(q5)*cos(q6)^2*sin(q5))/8 - (3^(1/2)*dq1*dqr1*cos(q4)*cos(q5)^2*cos(q6)*sin(q6))/2 - (3*dq4*dqr2*cos(q4)*cos(q6)*sin(q4)*sin(q5)*sin(q6))/4 - (3*dq5*dqr2*cos(q4)*cos(q6)*sin(q4)*sin(q5)*sin(q6))/4 - (3*dq6*dqr2*cos(q4)*cos(q6)*sin(q4)*sin(q5)*sin(q6))/4 - (3^(1/2)*dq1*dqr1*cos(q2)^2*cos(q4)*cos(q6)^2*sin(q5))/4 - (3^(1/2)*dq1*dqr1*cos(q3)^2*cos(q4)*cos(q6)^2*sin(q5))/4 + (3*3^(1/2)*dq6*dqr1*cos(q2)*cos(q3)*cos(q4)*sin(q5))/8 + (3^(1/2)*dq1*dqr1*cos(q4)*cos(q5)*cos(q6)*sin(q6))/4 - (3^(1/2)*dq1*dqr1*cos(q2)^2*cos(q4)*cos(q5)*cos(q6)*sin(q6))/2 + (3^(1/2)*dq4*dqr1*cos(q2)*cos(q3)*cos(q4)*cos(q6)^2*sin(q5))/8 - (3^(1/2)*dq1*dqr1*cos(q3)^2*cos(q4)*cos(q5)*cos(q6)*sin(q6))/2 + (3^(1/2)*dq5*dqr1*cos(q2)*cos(q3)*cos(q4)*cos(q6)^2*sin(q5))/16 - (3^(1/2)*dq6*dqr1*cos(q2)*cos(q3)*cos(q4)*cos(q6)^2*sin(q5))/4 - (5*dq4*dqr2*cos(q4)*cos(q5)*cos(q6)*sin(q4)*sin(q5)*sin(q6))/4 - dq5*dqr2*cos(q4)*cos(q5)*cos(q6)*sin(q4)*sin(q5)*sin(q6) - (5*dq6*dqr2*cos(q4)*cos(q5)*cos(q6)*sin(q4)*sin(q5)*sin(q6))/4 + 2*3^(1/2)*dq1*dqr1*cos(q2)^2*cos(q3)^2*cos(q4)*cos(q5)*sin(q5) + 3^(1/2)*dq1*dqr1*cos(q2)^2*cos(q3)^2*cos(q4)*cos(q6)*sin(q6) + (5*3^(1/2)*dq1*dqr1*cos(q2)^2*cos(q4)*cos(q5)*cos(q6)^2*sin(q5))/4 + 3^(1/2)*dq1*dqr1*cos(q2)^2*cos(q4)*cos(q5)^2*cos(q6)*sin(q6) + (5*3^(1/2)*dq1*dqr1*cos(q3)^2*cos(q4)*cos(q5)*cos(q6)^2*sin(q5))/4 + 3^(1/2)*dq1*dqr1*cos(q3)^2*cos(q4)*cos(q5)^2*cos(q6)*sin(q6) + (3^(1/2)*dq4*dqr1*cos(q2)*cos(q3)*cos(q4)*cos(q5)*sin(q5))/2 + (3^(1/2)*dq5*dqr1*cos(q2)*cos(q3)*cos(q4)*cos(q5)*sin(q5))/4 + (3^(1/2)*dq4*dqr1*cos(q2)*cos(q3)*cos(q4)*cos(q6)*sin(q6))/4 + (3^(1/2)*dq6*dqr1*cos(q2)*cos(q3)*cos(q4)*cos(q5)*sin(q5))/8 + (3^(1/2)*dq5*dqr1*cos(q2)*cos(q3)*cos(q4)*cos(q6)*sin(q6))/8 + (7*3^(1/2)*dq6*dqr1*cos(q2)*cos(q3)*cos(q4)*cos(q6)*sin(q6))/16 + (3^(1/2)*dq1*dqr1*cos(q2)^2*cos(q3)^2*cos(q4)*cos(q6)^2*sin(q5))/2 + 3^(1/2)*dq1*dqr1*cos(q2)^2*cos(q3)^2*cos(q4)*cos(q5)*cos(q6)*sin(q6) + (3^(1/2)*dq4*dqr1*cos(q2)*cos(q3)*cos(q4)*cos(q5)*cos(q6)*sin(q6))/4 + (3^(1/2)*dq5*dqr1*cos(q2)*cos(q3)*cos(q4)*cos(q5)*cos(q6)*sin(q6))/8 - (3^(1/2)*dq6*dqr1*cos(q2)*cos(q3)*cos(q4)*cos(q5)*cos(q6)*sin(q6))/8 - (5*3^(1/2)*dq1*dqr1*cos(q2)^2*cos(q3)^2*cos(q4)*cos(q5)*cos(q6)^2*sin(q5))/2 - 2*3^(1/2)*dq1*dqr1*cos(q2)^2*cos(q3)^2*cos(q4)*cos(q5)^2*cos(q6)*sin(q6) - (5*3^(1/2)*dq4*dqr1*cos(q2)*cos(q3)*cos(q4)*cos(q5)*cos(q6)^2*sin(q5))/8 - (3^(1/2)*dq4*dqr1*cos(q2)*cos(q3)*cos(q4)*cos(q5)^2*cos(q6)*sin(q6))/2 - (5*3^(1/2)*dq5*dqr1*cos(q2)*cos(q3)*cos(q4)*cos(q5)*cos(q6)^2*sin(q5))/16 - (3^(1/2)*dq5*dqr1*cos(q2)*cos(q3)*cos(q4)*cos(q5)^2*cos(q6)*sin(q6))/4 - (3^(1/2)*dq6*dqr1*cos(q2)*cos(q3)*cos(q4)*cos(q5)*cos(q6)^2*sin(q5))/4 - (5*3^(1/2)*dq6*dqr1*cos(q2)*cos(q3)*cos(q4)*cos(q5)^2*cos(q6)*sin(q6))/16;
Y2_20_5=(dq6*dqr2*sin(2*q4))/8 - (dq4*dqr3*sin(2*q5))/4 - (dq5*dqr3*sin(2*q4))/4 - (dq4*dqr3*sin(2*q4))/8 - (dq4*dqr3*sin(2*q6))/8 + (dq5*dqr2*sin(2*q6))/4 - (dq5*dqr3*sin(2*q5))/2 + (dq6*dqr2*sin(2*q5))/4 - (dq6*dqr3*sin(2*q4))/8 - (dq5*dqr3*sin(2*q6))/4 + (dq6*dqr2*sin(2*q6))/8 - (dq6*dqr3*sin(2*q5))/4 - (dq6*dqr3*sin(2*q6))/8 + (3*dq4*dqr3*cos(q6)^2*sin(q5))/8 + (3*dq6*dqr3*cos(q4)^2*sin(q5))/8 + (dq1*dqr4*cos(q3)*sin(q2))/4 - (dq1*dqr4*cos(q3)*cos(q4)^2*sin(q2))/4 - (dq1*dqr4*cos(q3)*cos(q5)^2*sin(q2))/4 + (5*dq1*dqr4*cos(q3)*cos(q6)^2*sin(q2))/16 + (5*dq4*dqr3*cos(q4)*cos(q5)^2*sin(q4))/4 - (dq4*dqr3*cos(q4)*cos(q6)^2*sin(q4))/16 + dq4*dqr3*cos(q4)^2*cos(q5)*sin(q5) + dq5*dqr3*cos(q4)*cos(q5)^2*sin(q4) + (5*dq5*dqr3*cos(q4)*cos(q6)^2*sin(q4))/8 + (5*dq5*dqr3*cos(q4)^2*cos(q5)*sin(q5))/4 + (dq6*dqr3*cos(q4)*cos(q5)^2*sin(q4))/2 + (5*dq4*dqr3*cos(q5)*cos(q6)^2*sin(q5))/8 + (dq4*dqr3*cos(q4)^2*cos(q6)*sin(q6))/2 + (dq6*dqr3*cos(q4)*cos(q6)^2*sin(q4))/2 + (5*dq6*dqr3*cos(q4)^2*cos(q5)*sin(q5))/8 + (dq4*dqr3*cos(q5)^2*cos(q6)*sin(q6))/2 + (5*dq5*dqr3*cos(q5)*cos(q6)^2*sin(q5))/4 + (5*dq5*dqr3*cos(q4)^2*cos(q6)*sin(q6))/8 + dq5*dqr3*cos(q5)^2*cos(q6)*sin(q6) + dq6*dqr3*cos(q5)*cos(q6)^2*sin(q5) - (dq6*dqr3*cos(q4)^2*cos(q6)*sin(q6))/16 + (5*dq6*dqr3*cos(q5)^2*cos(q6)*sin(q6))/4 - (3*dq4*dqr3*cos(q4)^2*cos(q6)^2*sin(q5))/4 - (3*dq5*dqr3*cos(q4)^2*cos(q6)^2*sin(q5))/16 - (3*dq6*dqr3*cos(q4)^2*cos(q6)^2*sin(q5))/4 + (3*dq6*dqr3*cos(q4)*cos(q5)*sin(q4))/4 + (3*dq4*dqr3*cos(q5)*cos(q6)*sin(q6))/4 - (3^(1/2)*dq1*dqr4*sin(q2)*sin(q3)*sin(q4))/4 + (5*dq1*dqr4*cos(q3)*cos(q4)^2*cos(q5)^2*sin(q2))/4 - (dq1*dqr4*cos(q3)*cos(q4)^2*cos(q6)^2*sin(q2))/16 + (5*dq1*dqr4*cos(q3)*cos(q5)^2*cos(q6)^2*sin(q2))/16 - (25*dq4*dqr3*cos(q4)*cos(q5)^2*cos(q6)^2*sin(q4))/16 - (5*dq4*dqr3*cos(q4)^2*cos(q5)*cos(q6)^2*sin(q5))/4 - (5*dq5*dqr3*cos(q4)*cos(q5)^2*cos(q6)^2*sin(q4))/4 - dq4*dqr3*cos(q4)^2*cos(q5)^2*cos(q6)*sin(q6) - (25*dq5*dqr3*cos(q4)^2*cos(q5)*cos(q6)^2*sin(q5))/16 - dq6*dqr3*cos(q4)*cos(q5)^2*cos(q6)^2*sin(q4) - (5*dq5*dqr3*cos(q4)^2*cos(q5)^2*cos(q6)*sin(q6))/4 - (5*dq6*dqr3*cos(q4)^2*cos(q5)*cos(q6)^2*sin(q5))/4 - (25*dq6*dqr3*cos(q4)^2*cos(q5)^2*cos(q6)*sin(q6))/16 + (3*dq1*dqr4*cos(q3)*cos(q5)*cos(q6)^2*sin(q2))/8 - (3*dq4*dqr3*cos(q4)*cos(q5)*cos(q6)^2*sin(q4))/8 - (3*dq5*dqr3*cos(q4)*cos(q5)*cos(q6)^2*sin(q4))/8 - (3*dq4*dqr3*cos(q4)^2*cos(q5)*cos(q6)*sin(q6))/2 - (3*dq6*dqr3*cos(q4)*cos(q5)*cos(q6)^2*sin(q4))/2 - (3*dq5*dqr3*cos(q4)^2*cos(q5)*cos(q6)*sin(q6))/8 - (3*dq6*dqr3*cos(q4)^2*cos(q5)*cos(q6)*sin(q6))/8 - (3*dq1*dqr4*cos(q3)*cos(q4)^2*cos(q5)*cos(q6)^2*sin(q2))/8 + (3^(1/2)*dq1*dqr4*cos(q5)^2*sin(q2)*sin(q3)*sin(q4))/4 + (7*3^(1/2)*dq1*dqr4*cos(q6)^2*sin(q2)*sin(q3)*sin(q4))/16 - (25*dq1*dqr4*cos(q3)*cos(q4)^2*cos(q5)^2*cos(q6)^2*sin(q2))/16 - (3*dq1*dqr4*cos(q3)*cos(q6)*sin(q2)*sin(q5)*sin(q6))/4 + (3*dq4*dqr3*cos(q4)*cos(q6)*sin(q4)*sin(q5)*sin(q6))/4 + (3*dq5*dqr3*cos(q4)*cos(q6)*sin(q4)*sin(q5)*sin(q6))/4 + (3*dq6*dqr3*cos(q4)*cos(q6)*sin(q4)*sin(q5)*sin(q6))/4 + (3^(1/2)*dq1*dqr4*cos(q4)*cos(q6)^2*sin(q2)*sin(q3)*sin(q5))/8 - (3^(1/2)*dq1*dqr4*cos(q5)*cos(q6)^2*sin(q2)*sin(q3)*sin(q4))/8 + dq1*dqr4*cos(q2)*cos(q4)*cos(q5)*sin(q3)*sin(q4)*sin(q5) - dq1*dqr4*cos(q3)*cos(q4)*cos(q5)*sin(q2)*sin(q4)*sin(q5) + (dq1*dqr4*cos(q2)*cos(q4)*cos(q6)*sin(q3)*sin(q4)*sin(q6))/2 - (dq1*dqr4*cos(q3)*cos(q4)*cos(q6)*sin(q2)*sin(q4)*sin(q6))/2 - (dq1*dqr4*cos(q3)*cos(q5)*cos(q6)*sin(q2)*sin(q5)*sin(q6))/4 + (5*dq4*dqr3*cos(q4)*cos(q5)*cos(q6)*sin(q4)*sin(q5)*sin(q6))/4 + dq5*dqr3*cos(q4)*cos(q5)*cos(q6)*sin(q4)*sin(q5)*sin(q6) + (5*dq6*dqr3*cos(q4)*cos(q5)*cos(q6)*sin(q4)*sin(q5)*sin(q6))/4 - (5*3^(1/2)*dq1*dqr4*cos(q5)^2*cos(q6)^2*sin(q2)*sin(q3)*sin(q4))/16 - (3*dq1*dqr4*cos(q2)*cos(q4)*cos(q6)^2*sin(q3)*sin(q4)*sin(q5))/4 + (3*dq1*dqr4*cos(q3)*cos(q4)*cos(q6)^2*sin(q2)*sin(q4)*sin(q5))/4 - (3*dq1*dqr4*cos(q2)*cos(q4)^2*cos(q6)*sin(q3)*sin(q5)*sin(q6))/4 + (3*dq1*dqr4*cos(q3)*cos(q4)^2*cos(q6)*sin(q2)*sin(q5)*sin(q6))/4 + (3^(1/2)*dq1*dqr4*cos(q4)*cos(q5)*sin(q2)*sin(q3)*sin(q5))/2 + (3^(1/2)*dq1*dqr4*cos(q4)*cos(q6)*sin(q2)*sin(q3)*sin(q6))/4 - (5*3^(1/2)*dq1*dqr4*cos(q4)*cos(q5)*cos(q6)^2*sin(q2)*sin(q3)*sin(q5))/8 - (3^(1/2)*dq1*dqr4*cos(q4)*cos(q5)^2*cos(q6)*sin(q2)*sin(q3)*sin(q6))/2 - (3*dq1*dqr4*cos(q2)*cos(q4)*cos(q5)*cos(q6)*sin(q3)*sin(q4)*sin(q6))/2 + (3*dq1*dqr4*cos(q3)*cos(q4)*cos(q5)*cos(q6)*sin(q2)*sin(q4)*sin(q6))/2 - (5*dq1*dqr4*cos(q2)*cos(q4)*cos(q5)*cos(q6)^2*sin(q3)*sin(q4)*sin(q5))/4 + (5*dq1*dqr4*cos(q3)*cos(q4)*cos(q5)*cos(q6)^2*sin(q2)*sin(q4)*sin(q5))/4 - dq1*dqr4*cos(q2)*cos(q4)*cos(q5)^2*cos(q6)*sin(q3)*sin(q4)*sin(q6) + dq1*dqr4*cos(q3)*cos(q4)*cos(q5)^2*cos(q6)*sin(q2)*sin(q4)*sin(q6) - (5*dq1*dqr4*cos(q2)*cos(q4)^2*cos(q5)*cos(q6)*sin(q3)*sin(q5)*sin(q6))/4 + (5*dq1*dqr4*cos(q3)*cos(q4)^2*cos(q5)*cos(q6)*sin(q2)*sin(q5)*sin(q6))/4 + (3^(1/2)*dq1*dqr4*cos(q4)*cos(q5)*cos(q6)*sin(q2)*sin(q3)*sin(q6))/4 + (3^(1/2)*dq1*dqr4*cos(q6)*sin(q2)*sin(q3)*sin(q4)*sin(q5)*sin(q6))/4 + (3^(1/2)*dq1*dqr4*cos(q5)*cos(q6)*sin(q2)*sin(q3)*sin(q4)*sin(q5)*sin(q6))/4;
Y2_20_6=(dq2*dqr4*sin(2*q4))/8 + (dq2*dqr4*sin(2*q5))/4 + (dq2*dqr4*sin(2*q6))/8 - (3*dq2*dqr4*cos(q6)^2*sin(q5))/8 + (3*dq3*dqr4*cos(q6)^2*sin(q5))/8 - (3^(1/2)*dq4*dqr4*sin(q4))/4 - (3^(1/2)*dq5*dqr4*sin(q4))/2 - (3^(1/2)*dq6*dqr4*sin(q4))/4 - (dq1*dqr4*cos(q2)*sin(q3))/4 + (dq1*dqr4*cos(q2)*cos(q4)^2*sin(q3))/4 + (dq1*dqr4*cos(q2)*cos(q5)^2*sin(q3))/4 - (5*dq1*dqr4*cos(q2)*cos(q6)^2*sin(q3))/16 - (5*dq2*dqr4*cos(q4)*cos(q5)^2*sin(q4))/4 + (dq2*dqr4*cos(q4)*cos(q6)^2*sin(q4))/16 - dq2*dqr4*cos(q4)^2*cos(q5)*sin(q5) + (5*dq3*dqr4*cos(q4)*cos(q5)^2*sin(q4))/4 - (dq3*dqr4*cos(q4)*cos(q6)^2*sin(q4))/16 + dq3*dqr4*cos(q4)^2*cos(q5)*sin(q5) - (5*dq2*dqr4*cos(q5)*cos(q6)^2*sin(q5))/8 - (dq2*dqr4*cos(q4)^2*cos(q6)*sin(q6))/2 - (dq2*dqr4*cos(q5)^2*cos(q6)*sin(q6))/2 + (5*dq3*dqr4*cos(q5)*cos(q6)^2*sin(q5))/8 + (dq3*dqr4*cos(q4)^2*cos(q6)*sin(q6))/2 + (dq3*dqr4*cos(q5)^2*cos(q6)*sin(q6))/2 + (3*3^(1/2)*dq6*dqr4*cos(q4)*sin(q5))/8 + (3*dq2*dqr4*cos(q4)^2*cos(q6)^2*sin(q5))/4 - (3*dq3*dqr4*cos(q4)^2*cos(q6)^2*sin(q5))/4 + (3^(1/2)*dq4*dqr4*cos(q5)^2*sin(q4))/4 + (7*3^(1/2)*dq4*dqr4*cos(q6)^2*sin(q4))/16 + (3^(1/2)*dq5*dqr4*cos(q5)^2*sin(q4))/2 + (3^(1/2)*dq5*dqr4*cos(q6)^2*sin(q4))/2 + (3^(1/2)*dq6*dqr4*cos(q5)^2*sin(q4))/4 + (3^(1/2)*dq6*dqr4*cos(q6)^2*sin(q4))/4 - (3*dq2*dqr4*cos(q5)*cos(q6)*sin(q6))/4 + (3*dq3*dqr4*cos(q5)*cos(q6)*sin(q6))/4 - (3^(1/2)*dq1*dqr4*cos(q2)*cos(q3)*sin(q4))/4 + (3^(1/2)*dq4*dqr4*cos(q4)*cos(q5)*sin(q5))/2 + (3^(1/2)*dq5*dqr4*cos(q4)*cos(q5)*sin(q5))/4 + (3^(1/2)*dq4*dqr4*cos(q4)*cos(q6)*sin(q6))/4 + (3^(1/2)*dq6*dqr4*cos(q4)*cos(q5)*sin(q5))/8 + (3^(1/2)*dq5*dqr4*cos(q4)*cos(q6)*sin(q6))/8 + (7*3^(1/2)*dq6*dqr4*cos(q4)*cos(q6)*sin(q6))/16 - (5*dq1*dqr4*cos(q2)*cos(q4)^2*cos(q5)^2*sin(q3))/4 + (dq1*dqr4*cos(q2)*cos(q4)^2*cos(q6)^2*sin(q3))/16 - (5*dq1*dqr4*cos(q2)*cos(q5)^2*cos(q6)^2*sin(q3))/16 + (25*dq2*dqr4*cos(q4)*cos(q5)^2*cos(q6)^2*sin(q4))/16 + (5*dq2*dqr4*cos(q4)^2*cos(q5)*cos(q6)^2*sin(q5))/4 - (25*dq3*dqr4*cos(q4)*cos(q5)^2*cos(q6)^2*sin(q4))/16 + dq2*dqr4*cos(q4)^2*cos(q5)^2*cos(q6)*sin(q6) - (5*dq3*dqr4*cos(q4)^2*cos(q5)*cos(q6)^2*sin(q5))/4 - dq3*dqr4*cos(q4)^2*cos(q5)^2*cos(q6)*sin(q6) + (3^(1/2)*dq4*dqr4*cos(q4)*cos(q6)^2*sin(q5))/8 - (3^(1/2)*dq4*dqr4*cos(q5)*cos(q6)^2*sin(q4))/8 + (3^(1/2)*dq5*dqr4*cos(q4)*cos(q6)^2*sin(q5))/16 + (3^(1/2)*dq5*dqr4*cos(q5)*cos(q6)^2*sin(q4))/8 - (3^(1/2)*dq6*dqr4*cos(q4)*cos(q6)^2*sin(q5))/4 + (3^(1/2)*dq6*dqr4*cos(q5)*cos(q6)^2*sin(q4))/4 - (5*3^(1/2)*dq4*dqr4*cos(q5)^2*cos(q6)^2*sin(q4))/16 - (5*3^(1/2)*dq5*dqr4*cos(q5)^2*cos(q6)^2*sin(q4))/8 - (3^(1/2)*dq6*dqr4*cos(q5)^2*cos(q6)^2*sin(q4))/2 - (3*dq1*dqr4*cos(q2)*cos(q5)*cos(q6)^2*sin(q3))/8 + (3*dq2*dqr4*cos(q4)*cos(q5)*cos(q6)^2*sin(q4))/8 - (3*dq3*dqr4*cos(q4)*cos(q5)*cos(q6)^2*sin(q4))/8 + (3*dq2*dqr4*cos(q4)^2*cos(q5)*cos(q6)*sin(q6))/2 - (3*dq3*dqr4*cos(q4)^2*cos(q5)*cos(q6)*sin(q6))/2 + (3^(1/2)*dq4*dqr4*cos(q6)*sin(q4)*sin(q5)*sin(q6))/4 - (3^(1/2)*dq5*dqr4*cos(q6)*sin(q4)*sin(q5)*sin(q6))/4 - (3^(1/2)*dq6*dqr4*cos(q6)*sin(q4)*sin(q5)*sin(q6))/8 + (3*dq1*dqr4*cos(q2)*cos(q4)^2*cos(q5)*cos(q6)^2*sin(q3))/8 + (3^(1/2)*dq1*dqr4*cos(q2)*cos(q3)*cos(q5)^2*sin(q4))/4 + (7*3^(1/2)*dq1*dqr4*cos(q2)*cos(q3)*cos(q6)^2*sin(q4))/16 - (5*3^(1/2)*dq4*dqr4*cos(q4)*cos(q5)*cos(q6)^2*sin(q5))/8 - (3^(1/2)*dq4*dqr4*cos(q4)*cos(q5)^2*cos(q6)*sin(q6))/2 - (5*3^(1/2)*dq5*dqr4*cos(q4)*cos(q5)*cos(q6)^2*sin(q5))/16 - (3^(1/2)*dq5*dqr4*cos(q4)*cos(q5)^2*cos(q6)*sin(q6))/4 - (3^(1/2)*dq6*dqr4*cos(q4)*cos(q5)*cos(q6)^2*sin(q5))/4 - (5*3^(1/2)*dq6*dqr4*cos(q4)*cos(q5)^2*cos(q6)*sin(q6))/16 + (25*dq1*dqr4*cos(q2)*cos(q4)^2*cos(q5)^2*cos(q6)^2*sin(q3))/16 + (3*dq1*dqr4*cos(q2)*cos(q6)*sin(q3)*sin(q5)*sin(q6))/4 - (3*dq2*dqr4*cos(q4)*cos(q6)*sin(q4)*sin(q5)*sin(q6))/4 + (3*dq3*dqr4*cos(q4)*cos(q6)*sin(q4)*sin(q5)*sin(q6))/4 + (3^(1/2)*dq4*dqr4*cos(q4)*cos(q5)*cos(q6)*sin(q6))/4 + (3^(1/2)*dq5*dqr4*cos(q4)*cos(q5)*cos(q6)*sin(q6))/8 - (3^(1/2)*dq6*dqr4*cos(q4)*cos(q5)*cos(q6)*sin(q6))/8 + (3^(1/2)*dq1*dqr4*cos(q2)*cos(q3)*cos(q4)*cos(q6)^2*sin(q5))/8 - (3^(1/2)*dq1*dqr4*cos(q2)*cos(q3)*cos(q5)*cos(q6)^2*sin(q4))/8 + (dq1*dqr4*cos(q2)*cos(q5)*cos(q6)*sin(q3)*sin(q5)*sin(q6))/4 - (5*dq2*dqr4*cos(q4)*cos(q5)*cos(q6)*sin(q4)*sin(q5)*sin(q6))/4 + (5*dq3*dqr4*cos(q4)*cos(q5)*cos(q6)*sin(q4)*sin(q5)*sin(q6))/4 - (5*3^(1/2)*dq1*dqr4*cos(q2)*cos(q3)*cos(q5)^2*cos(q6)^2*sin(q4))/16 + (3^(1/2)*dq1*dqr4*cos(q2)*cos(q3)*cos(q4)*cos(q5)*sin(q5))/2 + (3^(1/2)*dq1*dqr4*cos(q2)*cos(q3)*cos(q4)*cos(q6)*sin(q6))/4 + (3^(1/2)*dq4*dqr4*cos(q5)*cos(q6)*sin(q4)*sin(q5)*sin(q6))/4 + (3^(1/2)*dq5*dqr4*cos(q5)*cos(q6)*sin(q4)*sin(q5)*sin(q6))/2 + (5*3^(1/2)*dq6*dqr4*cos(q5)*cos(q6)*sin(q4)*sin(q5)*sin(q6))/8 + (3^(1/2)*dq1*dqr4*cos(q2)*cos(q3)*cos(q4)*cos(q5)*cos(q6)*sin(q6))/4 + (3^(1/2)*dq1*dqr4*cos(q2)*cos(q3)*cos(q6)*sin(q4)*sin(q5)*sin(q6))/4 - (5*3^(1/2)*dq1*dqr4*cos(q2)*cos(q3)*cos(q4)*cos(q5)*cos(q6)^2*sin(q5))/8 - (3^(1/2)*dq1*dqr4*cos(q2)*cos(q3)*cos(q4)*cos(q5)^2*cos(q6)*sin(q6))/2 + (3^(1/2)*dq1*dqr4*cos(q2)*cos(q3)*cos(q5)*cos(q6)*sin(q4)*sin(q5)*sin(q6))/4;
Y2_20_7=(dq1*dqr5*cos(q3)*sin(q2))/2 - (dq3*dqr4*sin(2*q5))/4 - (dq3*dqr4*sin(2*q6))/8 - (3^(1/2)*dq4*dqr5*sin(q4))/2 - (dq1*dqr5*cos(q2)*sin(q3))/2 - (dq3*dqr4*sin(2*q4))/8 + (dq1*dqr5*cos(q2)*cos(q4)^2*sin(q3))/2 - (dq1*dqr5*cos(q3)*cos(q4)^2*sin(q2))/2 + (dq1*dqr5*cos(q2)*cos(q5)^2*sin(q3))/2 - (dq1*dqr5*cos(q3)*cos(q5)^2*sin(q2))/2 + (dq1*dqr5*cos(q2)*cos(q6)^2*sin(q3))/2 - (dq1*dqr5*cos(q3)*cos(q6)^2*sin(q2))/2 - dq2*dqr5*cos(q4)*cos(q5)^2*sin(q4) - (5*dq2*dqr5*cos(q4)*cos(q6)^2*sin(q4))/8 - (5*dq2*dqr5*cos(q4)^2*cos(q5)*sin(q5))/4 + dq3*dqr5*cos(q4)*cos(q5)^2*sin(q4) + (5*dq3*dqr5*cos(q4)*cos(q6)^2*sin(q4))/8 + (5*dq3*dqr5*cos(q4)^2*cos(q5)*sin(q5))/4 + (3*dq2*dqr5*cos(q4)^2*cos(q6)^2*sin(q5))/16 - (3*dq3*dqr5*cos(q4)^2*cos(q6)^2*sin(q5))/16 + (3^(1/2)*dq4*dqr5*cos(q5)^2*sin(q4))/2 + (3^(1/2)*dq4*dqr5*cos(q6)^2*sin(q4))/2 - (3^(1/2)*dq1*dqr5*cos(q2)*cos(q3)*sin(q4))/2 + (3^(1/2)*dq4*dqr5*cos(q4)*cos(q5)*sin(q5))/4 - (3^(1/2)*dq1*dqr5*sin(q2)*sin(q3)*sin(q4))/2 - dq1*dqr5*cos(q2)*cos(q4)^2*cos(q5)^2*sin(q3) + dq1*dqr5*cos(q3)*cos(q4)^2*cos(q5)^2*sin(q2) - (5*dq1*dqr5*cos(q2)*cos(q4)^2*cos(q6)^2*sin(q3))/8 + (5*dq1*dqr5*cos(q3)*cos(q4)^2*cos(q6)^2*sin(q2))/8 - (5*dq1*dqr5*cos(q2)*cos(q5)^2*cos(q6)^2*sin(q3))/8 + (5*dq1*dqr5*cos(q3)*cos(q5)^2*cos(q6)^2*sin(q2))/8 + (5*dq2*dqr5*cos(q4)*cos(q5)^2*cos(q6)^2*sin(q4))/4 + (25*dq2*dqr5*cos(q4)^2*cos(q5)*cos(q6)^2*sin(q5))/16 - (5*dq3*dqr5*cos(q4)*cos(q5)^2*cos(q6)^2*sin(q4))/4 - (25*dq3*dqr5*cos(q4)^2*cos(q5)*cos(q6)^2*sin(q5))/16 + (3^(1/2)*dq4*dqr5*cos(q4)*cos(q6)^2*sin(q5))/16 + (3^(1/2)*dq4*dqr5*cos(q5)*cos(q6)^2*sin(q4))/8 + (3^(1/2)*dq5*dqr5*cos(q4)*cos(q6)^2*sin(q5))/8 + (3^(1/2)*dq5*dqr5*cos(q5)*cos(q6)^2*sin(q4))/4 + (3^(1/2)*dq6*dqr5*cos(q4)*cos(q6)^2*sin(q5))/4 + (3^(1/2)*dq6*dqr5*cos(q5)*cos(q6)^2*sin(q4))/2 - (5*3^(1/2)*dq4*dqr5*cos(q5)^2*cos(q6)^2*sin(q4))/8 - (3*dq1*dqr5*cos(q2)*cos(q5)*cos(q6)^2*sin(q3))/8 + (3*dq1*dqr5*cos(q3)*cos(q5)*cos(q6)^2*sin(q2))/8 + (3*dq2*dqr5*cos(q4)*cos(q5)*cos(q6)^2*sin(q4))/8 - (3*dq3*dqr5*cos(q4)*cos(q5)*cos(q6)^2*sin(q4))/8 - (3^(1/2)*dq4*dqr5*cos(q6)*sin(q4)*sin(q5)*sin(q6))/4 - (3^(1/2)*dq5*dqr5*cos(q6)*sin(q4)*sin(q5)*sin(q6))/2 - (3^(1/2)*dq6*dqr5*cos(q6)*sin(q4)*sin(q5)*sin(q6))/4 + (3*dq1*dqr5*cos(q2)*cos(q4)^2*cos(q5)*cos(q6)^2*sin(q3))/8 - (3*dq1*dqr5*cos(q3)*cos(q4)^2*cos(q5)*cos(q6)^2*sin(q2))/8 + (3^(1/2)*dq1*dqr5*cos(q2)*cos(q3)*cos(q5)^2*sin(q4))/2 + (3^(1/2)*dq1*dqr5*cos(q2)*cos(q3)*cos(q6)^2*sin(q4))/2 - (5*3^(1/2)*dq4*dqr5*cos(q4)*cos(q5)*cos(q6)^2*sin(q5))/16 + (3^(1/2)*dq1*dqr5*cos(q5)^2*sin(q2)*sin(q3)*sin(q4))/2 + (3^(1/2)*dq1*dqr5*cos(q6)^2*sin(q2)*sin(q3)*sin(q4))/2 + (5*dq1*dqr5*cos(q2)*cos(q4)^2*cos(q5)^2*cos(q6)^2*sin(q3))/4 - (5*dq1*dqr5*cos(q3)*cos(q4)^2*cos(q5)^2*cos(q6)^2*sin(q2))/4 + (3*dq1*dqr5*cos(q2)*cos(q6)*sin(q3)*sin(q5)*sin(q6))/4 - (3*dq1*dqr5*cos(q3)*cos(q6)*sin(q2)*sin(q5)*sin(q6))/4 - (3*dq2*dqr5*cos(q4)*cos(q6)*sin(q4)*sin(q5)*sin(q6))/4 + (3*dq3*dqr5*cos(q4)*cos(q6)*sin(q4)*sin(q5)*sin(q6))/4 + (3^(1/2)*dq1*dqr5*cos(q2)*cos(q3)*cos(q4)*cos(q6)^2*sin(q5))/16 + (3^(1/2)*dq1*dqr5*cos(q2)*cos(q3)*cos(q5)*cos(q6)^2*sin(q4))/8 + (3^(1/2)*dq1*dqr5*cos(q4)*cos(q6)^2*sin(q2)*sin(q3)*sin(q5))/16 + (3^(1/2)*dq1*dqr5*cos(q5)*cos(q6)^2*sin(q2)*sin(q3)*sin(q4))/8 + (5*dq1*dqr5*cos(q2)*cos(q4)*cos(q5)*sin(q3)*sin(q4)*sin(q5))/4 - (5*dq1*dqr5*cos(q3)*cos(q4)*cos(q5)*sin(q2)*sin(q4)*sin(q5))/4 + (5*dq1*dqr5*cos(q2)*cos(q4)*cos(q6)*sin(q3)*sin(q4)*sin(q6))/8 - (5*dq1*dqr5*cos(q3)*cos(q4)*cos(q6)*sin(q2)*sin(q4)*sin(q6))/8 + (dq1*dqr5*cos(q2)*cos(q5)*cos(q6)*sin(q3)*sin(q5)*sin(q6))/2 - (dq1*dqr5*cos(q3)*cos(q5)*cos(q6)*sin(q2)*sin(q5)*sin(q6))/2 - dq2*dqr5*cos(q4)*cos(q5)*cos(q6)*sin(q4)*sin(q5)*sin(q6) + dq3*dqr5*cos(q4)*cos(q5)*cos(q6)*sin(q4)*sin(q5)*sin(q6) - (5*3^(1/2)*dq1*dqr5*cos(q2)*cos(q3)*cos(q5)^2*cos(q6)^2*sin(q4))/8 - (5*3^(1/2)*dq1*dqr5*cos(q5)^2*cos(q6)^2*sin(q2)*sin(q3)*sin(q4))/8 - (3*dq1*dqr5*cos(q2)*cos(q4)*cos(q6)^2*sin(q3)*sin(q4)*sin(q5))/16 + (3*dq1*dqr5*cos(q3)*cos(q4)*cos(q6)^2*sin(q2)*sin(q4)*sin(q5))/16 - (3*dq1*dqr5*cos(q2)*cos(q4)^2*cos(q6)*sin(q3)*sin(q5)*sin(q6))/4 + (3*dq1*dqr5*cos(q3)*cos(q4)^2*cos(q6)*sin(q2)*sin(q5)*sin(q6))/4 + (3^(1/2)*dq1*dqr5*cos(q2)*cos(q3)*cos(q4)*cos(q5)*sin(q5))/4 + (3^(1/2)*dq1*dqr5*cos(q4)*cos(q5)*sin(q2)*sin(q3)*sin(q5))/4 + (3^(1/2)*dq1*dqr5*cos(q4)*cos(q6)*sin(q2)*sin(q3)*sin(q6))/8 + (3^(1/2)*dq4*dqr5*cos(q5)*cos(q6)*sin(q4)*sin(q5)*sin(q6))/2 - (5*3^(1/2)*dq1*dqr5*cos(q4)*cos(q5)*cos(q6)^2*sin(q2)*sin(q3)*sin(q5))/16 - (3^(1/2)*dq1*dqr5*cos(q4)*cos(q5)^2*cos(q6)*sin(q2)*sin(q3)*sin(q6))/4 - (3*dq1*dqr5*cos(q2)*cos(q4)*cos(q5)*cos(q6)*sin(q3)*sin(q4)*sin(q6))/8 + (3*dq1*dqr5*cos(q3)*cos(q4)*cos(q5)*cos(q6)*sin(q2)*sin(q4)*sin(q6))/8 - (25*dq1*dqr5*cos(q2)*cos(q4)*cos(q5)*cos(q6)^2*sin(q3)*sin(q4)*sin(q5))/16 + (25*dq1*dqr5*cos(q3)*cos(q4)*cos(q5)*cos(q6)^2*sin(q2)*sin(q4)*sin(q5))/16 - (5*dq1*dqr5*cos(q2)*cos(q4)*cos(q5)^2*cos(q6)*sin(q3)*sin(q4)*sin(q6))/4 + (5*dq1*dqr5*cos(q3)*cos(q4)*cos(q5)^2*cos(q6)*sin(q2)*sin(q4)*sin(q6))/4 - dq1*dqr5*cos(q2)*cos(q4)^2*cos(q5)*cos(q6)*sin(q3)*sin(q5)*sin(q6) + dq1*dqr5*cos(q3)*cos(q4)^2*cos(q5)*cos(q6)*sin(q2)*sin(q5)*sin(q6) - (3^(1/2)*dq1*dqr5*cos(q2)*cos(q3)*cos(q6)*sin(q4)*sin(q5)*sin(q6))/4 + (3^(1/2)*dq1*dqr5*cos(q4)*cos(q5)*cos(q6)*sin(q2)*sin(q3)*sin(q6))/8 - (3^(1/2)*dq1*dqr5*cos(q6)*sin(q2)*sin(q3)*sin(q4)*sin(q5)*sin(q6))/4 - (5*3^(1/2)*dq1*dqr5*cos(q2)*cos(q3)*cos(q4)*cos(q5)*cos(q6)^2*sin(q5))/16 + (3^(1/2)*dq1*dqr5*cos(q2)*cos(q3)*cos(q5)*cos(q6)*sin(q4)*sin(q5)*sin(q6))/2 + (3^(1/2)*dq1*dqr5*cos(q5)*cos(q6)*sin(q2)*sin(q3)*sin(q4)*sin(q5)*sin(q6))/2;
Y2_20_8=(dq2*dqr5*sin(2*q4))/4 + (dq2*dqr5*sin(2*q5))/2 - (dq3*dqr5*sin(2*q4))/4 + (dq2*dqr5*sin(2*q6))/4 - (dq3*dqr5*sin(2*q5))/2 - (dq3*dqr5*sin(2*q6))/4 - (dq1*dqr6*cos(q2)*sin(q3))/4 + (dq1*dqr6*cos(q3)*sin(q2))/4 + (dq1*dqr6*cos(q2)*cos(q4)^2*sin(q3))/4 - (dq1*dqr6*cos(q3)*cos(q4)^2*sin(q2))/4 + (dq1*dqr6*cos(q2)*cos(q5)^2*sin(q3))/4 - (dq1*dqr6*cos(q3)*cos(q5)^2*sin(q2))/4 + (dq1*dqr6*cos(q2)*cos(q6)^2*sin(q3))/4 - (dq1*dqr6*cos(q3)*cos(q6)^2*sin(q2))/4 - (dq2*dqr6*cos(q4)*cos(q5)^2*sin(q4))/2 - (5*dq2*dqr5*cos(q5)*cos(q6)^2*sin(q5))/4 - (5*dq2*dqr5*cos(q4)^2*cos(q6)*sin(q6))/8 - dq2*dqr5*cos(q5)^2*cos(q6)*sin(q6) + (5*dq3*dqr5*cos(q5)*cos(q6)^2*sin(q5))/4 + (5*dq3*dqr5*cos(q4)^2*cos(q6)*sin(q6))/8 + dq3*dqr5*cos(q5)^2*cos(q6)*sin(q6) - (3^(1/2)*dq1*dqr6*cos(q2)*cos(q3)*sin(q4))/4 + (3^(1/2)*dq4*dqr5*cos(q4)*cos(q6)*sin(q6))/8 + (3*3^(1/2)*dq6*dqr5*cos(q4)*cos(q6)*sin(q6))/8 - (3^(1/2)*dq1*dqr6*sin(q2)*sin(q3)*sin(q4))/4 - (dq1*dqr6*cos(q2)*cos(q4)^2*cos(q5)^2*sin(q3))/2 + (dq1*dqr6*cos(q3)*cos(q4)^2*cos(q5)^2*sin(q2))/2 - (dq1*dqr6*cos(q2)*cos(q4)^2*cos(q6)^2*sin(q3))/2 + (dq1*dqr6*cos(q3)*cos(q4)^2*cos(q6)^2*sin(q2))/2 - (dq1*dqr6*cos(q2)*cos(q5)^2*cos(q6)^2*sin(q3))/2 + (dq1*dqr6*cos(q3)*cos(q5)^2*cos(q6)^2*sin(q2))/2 + dq2*dqr6*cos(q4)*cos(q5)^2*cos(q6)^2*sin(q4) + (5*dq2*dqr5*cos(q4)^2*cos(q5)^2*cos(q6)*sin(q6))/4 - dq3*dqr6*cos(q4)*cos(q5)^2*cos(q6)^2*sin(q4) - (5*dq3*dqr5*cos(q4)^2*cos(q5)^2*cos(q6)*sin(q6))/4 - (3*dq1*dqr6*cos(q2)*cos(q4)^2*cos(q5)*sin(q3))/4 + (3*dq1*dqr6*cos(q3)*cos(q4)^2*cos(q5)*sin(q2))/4 - (3*dq1*dqr6*cos(q2)*cos(q5)*cos(q6)^2*sin(q3))/4 + (3*dq1*dqr6*cos(q3)*cos(q5)*cos(q6)^2*sin(q2))/4 + (3*dq2*dqr5*cos(q4)^2*cos(q5)*cos(q6)*sin(q6))/8 - (3*dq3*dqr5*cos(q4)^2*cos(q5)*cos(q6)*sin(q6))/8 + (3*3^(1/2)*dq1*dqr6*cos(q4)*sin(q2)*sin(q3)*sin(q5))/8 - (3^(1/2)*dq4*dqr6*cos(q6)*sin(q4)*sin(q5)*sin(q6))/8 - (3^(1/2)*dq5*dqr6*cos(q6)*sin(q4)*sin(q5)*sin(q6))/4 + (3*dq1*dqr6*cos(q2)*cos(q4)^2*cos(q5)*cos(q6)^2*sin(q3))/2 - (3*dq1*dqr6*cos(q3)*cos(q4)^2*cos(q5)*cos(q6)^2*sin(q2))/2 + (3^(1/2)*dq1*dqr6*cos(q2)*cos(q3)*cos(q5)^2*sin(q4))/4 + (3^(1/2)*dq1*dqr6*cos(q2)*cos(q3)*cos(q6)^2*sin(q4))/4 - (3^(1/2)*dq4*dqr5*cos(q4)*cos(q5)^2*cos(q6)*sin(q6))/4 + (3^(1/2)*dq1*dqr6*cos(q5)^2*sin(q2)*sin(q3)*sin(q4))/4 + (3^(1/2)*dq1*dqr6*cos(q6)^2*sin(q2)*sin(q3)*sin(q4))/4 + dq1*dqr6*cos(q2)*cos(q4)^2*cos(q5)^2*cos(q6)^2*sin(q3) - dq1*dqr6*cos(q3)*cos(q4)^2*cos(q5)^2*cos(q6)^2*sin(q2) + (3*dq1*dqr6*cos(q2)*cos(q4)*sin(q3)*sin(q4)*sin(q5))/8 - (3*dq1*dqr6*cos(q3)*cos(q4)*sin(q2)*sin(q4)*sin(q5))/8 + (3*dq1*dqr6*cos(q2)*cos(q6)*sin(q3)*sin(q5)*sin(q6))/8 - (3*dq1*dqr6*cos(q3)*cos(q6)*sin(q2)*sin(q5)*sin(q6))/8 - (3*dq2*dqr6*cos(q4)*cos(q6)*sin(q4)*sin(q5)*sin(q6))/4 + (3*dq3*dqr6*cos(q4)*cos(q6)*sin(q4)*sin(q5)*sin(q6))/4 + (3^(1/2)*dq4*dqr5*cos(q4)*cos(q5)*cos(q6)*sin(q6))/8 + (3^(1/2)*dq5*dqr5*cos(q4)*cos(q5)*cos(q6)*sin(q6))/4 + (3^(1/2)*dq6*dqr5*cos(q4)*cos(q5)*cos(q6)*sin(q6))/8 + (3^(1/2)*dq1*dqr6*cos(q2)*cos(q3)*cos(q5)*cos(q6)^2*sin(q4))/4 - (3^(1/2)*dq1*dqr6*cos(q4)*cos(q6)^2*sin(q2)*sin(q3)*sin(q5))/4 + (3^(1/2)*dq1*dqr6*cos(q5)*cos(q6)^2*sin(q2)*sin(q3)*sin(q4))/4 + (5*dq1*dqr6*cos(q2)*cos(q4)*cos(q5)*sin(q3)*sin(q4)*sin(q5))/8 - (5*dq1*dqr6*cos(q3)*cos(q4)*cos(q5)*sin(q2)*sin(q4)*sin(q5))/8 - (dq1*dqr6*cos(q2)*cos(q4)*cos(q6)*sin(q3)*sin(q4)*sin(q6))/16 + (dq1*dqr6*cos(q3)*cos(q4)*cos(q6)*sin(q2)*sin(q4)*sin(q6))/16 + (5*dq1*dqr6*cos(q2)*cos(q5)*cos(q6)*sin(q3)*sin(q5)*sin(q6))/8 - (5*dq1*dqr6*cos(q3)*cos(q5)*cos(q6)*sin(q2)*sin(q5)*sin(q6))/8 - (5*dq2*dqr6*cos(q4)*cos(q5)*cos(q6)*sin(q4)*sin(q5)*sin(q6))/4 + (5*dq3*dqr6*cos(q4)*cos(q5)*cos(q6)*sin(q4)*sin(q5)*sin(q6))/4 - (3^(1/2)*dq1*dqr6*cos(q2)*cos(q3)*cos(q5)^2*cos(q6)^2*sin(q4))/2 - (3^(1/2)*dq1*dqr6*cos(q5)^2*cos(q6)^2*sin(q2)*sin(q3)*sin(q4))/2 - (3*dq1*dqr6*cos(q2)*cos(q4)*cos(q6)^2*sin(q3)*sin(q4)*sin(q5))/4 + (3*dq1*dqr6*cos(q3)*cos(q4)*cos(q6)^2*sin(q2)*sin(q4)*sin(q5))/4 - (3*dq1*dqr6*cos(q2)*cos(q4)^2*cos(q6)*sin(q3)*sin(q5)*sin(q6))/4 + (3*dq1*dqr6*cos(q3)*cos(q4)^2*cos(q6)*sin(q2)*sin(q5)*sin(q6))/4 + (3^(1/2)*dq1*dqr5*cos(q2)*cos(q3)*cos(q4)*cos(q6)*sin(q6))/8 + (3^(1/2)*dq1*dqr6*cos(q4)*cos(q5)*sin(q2)*sin(q3)*sin(q5))/8 + (7*3^(1/2)*dq1*dqr6*cos(q4)*cos(q6)*sin(q2)*sin(q3)*sin(q6))/16 + (5*3^(1/2)*dq4*dqr6*cos(q5)*cos(q6)*sin(q4)*sin(q5)*sin(q6))/8 - (3^(1/2)*dq1*dqr6*cos(q4)*cos(q5)*cos(q6)^2*sin(q2)*sin(q3)*sin(q5))/4 - (5*3^(1/2)*dq1*dqr6*cos(q4)*cos(q5)^2*cos(q6)*sin(q2)*sin(q3)*sin(q6))/16 - (3*dq1*dqr6*cos(q2)*cos(q4)*cos(q5)*cos(q6)*sin(q3)*sin(q4)*sin(q6))/8 + (3*dq1*dqr6*cos(q3)*cos(q4)*cos(q5)*cos(q6)*sin(q2)*sin(q4)*sin(q6))/8 - (5*dq1*dqr6*cos(q2)*cos(q4)*cos(q5)*cos(q6)^2*sin(q3)*sin(q4)*sin(q5))/4 + (5*dq1*dqr6*cos(q3)*cos(q4)*cos(q5)*cos(q6)^2*sin(q2)*sin(q4)*sin(q5))/4 - (25*dq1*dqr6*cos(q2)*cos(q4)*cos(q5)^2*cos(q6)*sin(q3)*sin(q4)*sin(q6))/16 + (25*dq1*dqr6*cos(q3)*cos(q4)*cos(q5)^2*cos(q6)*sin(q2)*sin(q4)*sin(q6))/16 - (5*dq1*dqr6*cos(q2)*cos(q4)^2*cos(q5)*cos(q6)*sin(q3)*sin(q5)*sin(q6))/4 + (5*dq1*dqr6*cos(q3)*cos(q4)^2*cos(q5)*cos(q6)*sin(q2)*sin(q5)*sin(q6))/4 + (3^(1/2)*dq1*dqr5*cos(q2)*cos(q3)*cos(q4)*cos(q5)*cos(q6)*sin(q6))/8 - (3^(1/2)*dq1*dqr6*cos(q2)*cos(q3)*cos(q6)*sin(q4)*sin(q5)*sin(q6))/8 - (3^(1/2)*dq1*dqr6*cos(q4)*cos(q5)*cos(q6)*sin(q2)*sin(q3)*sin(q6))/8 - (3^(1/2)*dq1*dqr6*cos(q6)*sin(q2)*sin(q3)*sin(q4)*sin(q5)*sin(q6))/8 - (3^(1/2)*dq1*dqr5*cos(q2)*cos(q3)*cos(q4)*cos(q5)^2*cos(q6)*sin(q6))/4 + (5*3^(1/2)*dq1*dqr6*cos(q2)*cos(q3)*cos(q5)*cos(q6)*sin(q4)*sin(q5)*sin(q6))/8 + (5*3^(1/2)*dq1*dqr6*cos(q5)*cos(q6)*sin(q2)*sin(q3)*sin(q4)*sin(q5)*sin(q6))/8;
Y2_20_9=(dq2*dqr6*sin(2*q4))/8 + (dq2*dqr6*sin(2*q5))/4 - (dq3*dqr6*sin(2*q4))/8 + (dq2*dqr6*sin(2*q6))/8 - (dq3*dqr6*sin(2*q5))/4 - (dq3*dqr6*sin(2*q6))/8 - (3*dq2*dqr6*cos(q4)^2*sin(q5))/8 + (3*dq3*dqr6*cos(q4)^2*sin(q5))/8 - (3^(1/2)*dq4*dqr6*sin(q4))/4 - (dq2*dqr6*cos(q4)*cos(q6)^2*sin(q4))/2 - (5*dq2*dqr6*cos(q4)^2*cos(q5)*sin(q5))/8 + (dq3*dqr6*cos(q4)*cos(q5)^2*sin(q4))/2 + (dq3*dqr6*cos(q4)*cos(q6)^2*sin(q4))/2 + (5*dq3*dqr6*cos(q4)^2*cos(q5)*sin(q5))/8 - dq2*dqr6*cos(q5)*cos(q6)^2*sin(q5) + (dq2*dqr6*cos(q4)^2*cos(q6)*sin(q6))/16 - (5*dq2*dqr6*cos(q5)^2*cos(q6)*sin(q6))/4 + dq3*dqr6*cos(q5)*cos(q6)^2*sin(q5) - (dq3*dqr6*cos(q4)^2*cos(q6)*sin(q6))/16 + (5*dq3*dqr6*cos(q5)^2*cos(q6)*sin(q6))/4 + (ddqr1*cos(q2)*cos(q4)*sin(q3)*sin(q4))/4 - (ddqr1*cos(q3)*cos(q4)*sin(q2)*sin(q4))/4 + (ddqr1*cos(q2)*cos(q5)*sin(q3)*sin(q5))/2 - (ddqr1*cos(q3)*cos(q5)*sin(q2)*sin(q5))/2 - (ddqr1*cos(q3)*cos(q6)*sin(q2)*sin(q6))/4 + (3*3^(1/2)*dq4*dqr6*cos(q4)*sin(q5))/8 + (3*dq2*dqr6*cos(q4)^2*cos(q6)^2*sin(q5))/4 - (3*dq3*dqr6*cos(q4)^2*cos(q6)^2*sin(q5))/4 - (3*ddqr1*cos(q2)*cos(q6)^2*sin(q3)*sin(q5))/8 + (3*ddqr1*cos(q3)*cos(q6)^2*sin(q2)*sin(q5))/8 + (3^(1/2)*dq4*dqr6*cos(q5)^2*sin(q4))/4 + (3^(1/2)*dq4*dqr6*cos(q6)^2*sin(q4))/4 - (3*dq2*dqr6*cos(q4)*cos(q5)*sin(q4))/4 + (3*dq3*dqr6*cos(q4)*cos(q5)*sin(q4))/4 + (3^(1/2)*ddqr1*cos(q4)*sin(q2)*sin(q3))/4 + (3*ddqr1*cos(q3)*cos(q5)*cos(q6)*sin(q2)*sin(q6))/4 + (3^(1/2)*dq4*dqr6*cos(q4)*cos(q5)*sin(q5))/8 + (7*3^(1/2)*dq4*dqr6*cos(q4)*cos(q6)*sin(q6))/16 + (3*3^(1/2)*dq5*dqr6*cos(q4)*cos(q6)*sin(q6))/8 + (5*dq2*dqr6*cos(q4)^2*cos(q5)*cos(q6)^2*sin(q5))/4 + (25*dq2*dqr6*cos(q4)^2*cos(q5)^2*cos(q6)*sin(q6))/16 - (5*dq3*dqr6*cos(q4)^2*cos(q5)*cos(q6)^2*sin(q5))/4 - (25*dq3*dqr6*cos(q4)^2*cos(q5)^2*cos(q6)*sin(q6))/16 - (5*ddqr1*cos(q2)*cos(q4)*cos(q5)^2*sin(q3)*sin(q4))/4 + (5*ddqr1*cos(q3)*cos(q4)*cos(q5)^2*sin(q2)*sin(q4))/4 + (ddqr1*cos(q2)*cos(q4)*cos(q6)^2*sin(q3)*sin(q4))/16 - ddqr1*cos(q2)*cos(q4)^2*cos(q5)*sin(q3)*sin(q5) - (ddqr1*cos(q3)*cos(q4)*cos(q6)^2*sin(q2)*sin(q4))/16 + ddqr1*cos(q3)*cos(q4)^2*cos(q5)*sin(q2)*sin(q5) - (5*ddqr1*cos(q2)*cos(q5)*cos(q6)^2*sin(q3)*sin(q5))/8 + (5*ddqr1*cos(q3)*cos(q5)*cos(q6)^2*sin(q2)*sin(q5))/8 + (ddqr1*cos(q3)*cos(q4)^2*cos(q6)*sin(q2)*sin(q6))/2 + (ddqr1*cos(q3)*cos(q5)^2*cos(q6)*sin(q2)*sin(q6))/2 - (3^(1/2)*dq4*dqr6*cos(q4)*cos(q6)^2*sin(q5))/4 + (3^(1/2)*dq4*dqr6*cos(q5)*cos(q6)^2*sin(q4))/4 + (3^(1/2)*dq5*dqr6*cos(q4)*cos(q6)^2*sin(q5))/4 + (3^(1/2)*dq5*dqr6*cos(q5)*cos(q6)^2*sin(q4))/2 + (3*ddqr1*cos(q2)*cos(q4)^2*cos(q6)^2*sin(q3)*sin(q5))/4 - (3*ddqr1*cos(q3)*cos(q4)^2*cos(q6)^2*sin(q2)*sin(q5))/4 - (3^(1/2)*dq4*dqr6*cos(q5)^2*cos(q6)^2*sin(q4))/2 + (3*dq2*dqr6*cos(q4)*cos(q5)*cos(q6)^2*sin(q4))/2 - (3*dq3*dqr6*cos(q4)*cos(q5)*cos(q6)^2*sin(q4))/2 + (3*dq2*dqr6*cos(q4)^2*cos(q5)*cos(q6)*sin(q6))/8 - (3*dq3*dqr6*cos(q4)^2*cos(q5)*cos(q6)*sin(q6))/8 - (3^(1/2)*ddqr1*cos(q4)*cos(q5)^2*sin(q2)*sin(q3))/4 - (7*3^(1/2)*ddqr1*cos(q4)*cos(q6)^2*sin(q2)*sin(q3))/16 + (5*3^(1/2)*ddqr1*cos(q4)*cos(q5)^2*cos(q6)^2*sin(q2)*sin(q3))/16 + (3*ddqr1*cos(q2)*cos(q4)*cos(q5)*cos(q6)^2*sin(q3)*sin(q4))/8 - (3*ddqr1*cos(q3)*cos(q4)*cos(q5)*cos(q6)^2*sin(q2)*sin(q4))/8 - (3*ddqr1*cos(q3)*cos(q4)^2*cos(q5)*cos(q6)*sin(q2)*sin(q6))/2 - (3^(1/2)*dq4*dqr6*cos(q4)*cos(q5)*cos(q6)^2*sin(q5))/4 - (5*3^(1/2)*dq4*dqr6*cos(q4)*cos(q5)^2*cos(q6)*sin(q6))/16 + (3^(1/2)*ddqr1*cos(q5)*sin(q2)*sin(q3)*sin(q4)*sin(q5))/2 + (3^(1/2)*ddqr1*cos(q6)*sin(q2)*sin(q3)*sin(q4)*sin(q6))/4 + (25*ddqr1*cos(q2)*cos(q4)*cos(q5)^2*cos(q6)^2*sin(q3)*sin(q4))/16 - (25*ddqr1*cos(q3)*cos(q4)*cos(q5)^2*cos(q6)^2*sin(q2)*sin(q4))/16 + (5*ddqr1*cos(q2)*cos(q4)^2*cos(q5)*cos(q6)^2*sin(q3)*sin(q5))/4 - (5*ddqr1*cos(q3)*cos(q4)^2*cos(q5)*cos(q6)^2*sin(q2)*sin(q5))/4 + ddqr1*cos(q2)*cos(q4)^2*cos(q5)^2*cos(q6)*sin(q3)*sin(q6) - ddqr1*cos(q3)*cos(q4)^2*cos(q5)^2*cos(q6)*sin(q2)*sin(q6) + (3^(1/2)*ddqr1*cos(q4)*cos(q5)*cos(q6)^2*sin(q2)*sin(q3))/8 + (3^(1/2)*ddqr1*cos(q6)^2*sin(q2)*sin(q3)*sin(q4)*sin(q5))/8 + (3*3^(1/2)*dq1*dqr6*cos(q2)*cos(q3)*cos(q4)*sin(q5))/8 - (3^(1/2)*dq4*dqr6*cos(q4)*cos(q5)*cos(q6)*sin(q6))/8 + (3^(1/2)*dq5*dqr6*cos(q4)*cos(q5)*cos(q6)*sin(q6))/8 - (3^(1/2)*dq1*dqr6*cos(q2)*cos(q3)*cos(q4)*cos(q6)^2*sin(q5))/4 - (3^(1/2)*ddqr1*cos(q4)*cos(q6)*sin(q2)*sin(q3)*sin(q5)*sin(q6))/4 + (3^(1/2)*ddqr1*cos(q5)*cos(q6)*sin(q2)*sin(q3)*sin(q4)*sin(q6))/4 - (5*3^(1/2)*ddqr1*cos(q5)*cos(q6)^2*sin(q2)*sin(q3)*sin(q4)*sin(q5))/8 - (3^(1/2)*ddqr1*cos(q5)^2*cos(q6)*sin(q2)*sin(q3)*sin(q4)*sin(q6))/2 + (3^(1/2)*dq1*dqr6*cos(q2)*cos(q3)*cos(q4)*cos(q5)*sin(q5))/8 + (7*3^(1/2)*dq1*dqr6*cos(q2)*cos(q3)*cos(q4)*cos(q6)*sin(q6))/16 - (3*ddqr1*cos(q2)*cos(q4)*cos(q6)*sin(q3)*sin(q4)*sin(q5)*sin(q6))/4 + (3*ddqr1*cos(q3)*cos(q4)*cos(q6)*sin(q2)*sin(q4)*sin(q5)*sin(q6))/4 - (3^(1/2)*ddqr1*cos(q4)*cos(q5)*cos(q6)*sin(q2)*sin(q3)*sin(q5)*sin(q6))/4 - (3^(1/2)*dq1*dqr6*cos(q2)*cos(q3)*cos(q4)*cos(q5)*cos(q6)*sin(q6))/8 - (5*ddqr1*cos(q2)*cos(q4)*cos(q5)*cos(q6)*sin(q3)*sin(q4)*sin(q5)*sin(q6))/4 + (5*ddqr1*cos(q3)*cos(q4)*cos(q5)*cos(q6)*sin(q2)*sin(q4)*sin(q5)*sin(q6))/4 - (3^(1/2)*dq1*dqr6*cos(q2)*cos(q3)*cos(q4)*cos(q5)*cos(q6)^2*sin(q5))/4 - (5*3^(1/2)*dq1*dqr6*cos(q2)*cos(q3)*cos(q4)*cos(q5)^2*cos(q6)*sin(q6))/16;
Y2_20_10=ddqr2 - ddqr3 - (ddqr2*cos(q4)^2)/4 - ddqr2*cos(q5)^2 + (ddqr3*cos(q4)^2)/4 - (ddqr2*cos(q6)^2)/4 + ddqr3*cos(q5)^2 + (ddqr3*cos(q6)^2)/4 + (5*ddqr2*cos(q4)^2*cos(q5)^2)/4 - (ddqr2*cos(q4)^2*cos(q6)^2)/16 - (5*ddqr3*cos(q4)^2*cos(q5)^2)/4 + (5*ddqr2*cos(q5)^2*cos(q6)^2)/4 + (ddqr3*cos(q4)^2*cos(q6)^2)/16 - (5*ddqr3*cos(q5)^2*cos(q6)^2)/4 + (3^(1/2)*ddqr4*cos(q4))/4 + (3^(1/2)*ddqr5*cos(q4))/2 + (3^(1/2)*ddqr6*cos(q4))/4 - (3*ddqr2*cos(q4)^2*cos(q5)*cos(q6)^2)/8 + (3*ddqr3*cos(q4)^2*cos(q5)*cos(q6)^2)/8 - (3^(1/2)*ddqr4*cos(q4)*cos(q5)^2)/4 - (7*3^(1/2)*ddqr4*cos(q4)*cos(q6)^2)/16 - (3*3^(1/2)*ddqr5*cos(q4)*cos(q6)^2)/8 - (25*ddqr2*cos(q4)^2*cos(q5)^2*cos(q6)^2)/16 + (25*ddqr3*cos(q4)^2*cos(q5)^2*cos(q6)^2)/16 - (3^(1/2)*ddqr6*cos(q4)*cos(q5))/4 + (3^(1/2)*ddqr6*sin(q4)*sin(q5))/2 + (3^(1/2)*ddqr4*cos(q4)*cos(q5)*cos(q6)^2)/8 - (3^(1/2)*ddqr5*cos(q4)*cos(q5)*cos(q6)^2)/8 + (3^(1/2)*ddqr4*cos(q6)^2*sin(q4)*sin(q5))/8 + (3^(1/2)*ddqr5*cos(q6)^2*sin(q4)*sin(q5))/4 + (ddqr1*cos(q2)*cos(q6)*sin(q3)*sin(q6))/4 - ddqr2*cos(q4)*cos(q5)*sin(q4)*sin(q5) + ddqr3*cos(q4)*cos(q5)*sin(q4)*sin(q5) - (ddqr2*cos(q4)*cos(q6)*sin(q4)*sin(q6))/2 + (ddqr3*cos(q4)*cos(q6)*sin(q4)*sin(q6))/2 - ddqr2*cos(q5)*cos(q6)*sin(q5)*sin(q6) + ddqr3*cos(q5)*cos(q6)*sin(q5)*sin(q6) + (5*3^(1/2)*ddqr4*cos(q4)*cos(q5)^2*cos(q6)^2)/16 + (3*ddqr2*cos(q4)*cos(q6)^2*sin(q4)*sin(q5))/4 - (3*ddqr3*cos(q4)*cos(q6)^2*sin(q4)*sin(q5))/4 + (3*ddqr2*cos(q4)^2*cos(q6)*sin(q5)*sin(q6))/4 - (3*ddqr3*cos(q4)^2*cos(q6)*sin(q5)*sin(q6))/4 + (3^(1/2)*ddqr1*cos(q2)*cos(q3)*cos(q4))/4 + (3^(1/2)*ddqr4*cos(q5)*sin(q4)*sin(q5))/2 + (3^(1/2)*ddqr4*cos(q6)*sin(q4)*sin(q6))/4 - (3*ddqr1*cos(q2)*cos(q5)*cos(q6)*sin(q3)*sin(q6))/4 + (3*ddqr2*cos(q4)*cos(q5)*cos(q6)*sin(q4)*sin(q6))/2 - (3*ddqr3*cos(q4)*cos(q5)*cos(q6)*sin(q4)*sin(q6))/2 - (ddqr1*cos(q2)*cos(q4)^2*cos(q6)*sin(q3)*sin(q6))/2 - (ddqr1*cos(q2)*cos(q5)^2*cos(q6)*sin(q3)*sin(q6))/2 + (5*ddqr2*cos(q4)*cos(q5)*cos(q6)^2*sin(q4)*sin(q5))/4 + ddqr2*cos(q4)*cos(q5)^2*cos(q6)*sin(q4)*sin(q6) - (5*ddqr3*cos(q4)*cos(q5)*cos(q6)^2*sin(q4)*sin(q5))/4 + (5*ddqr2*cos(q4)^2*cos(q5)*cos(q6)*sin(q5)*sin(q6))/4 - ddqr3*cos(q4)*cos(q5)^2*cos(q6)*sin(q4)*sin(q6) - (5*ddqr3*cos(q4)^2*cos(q5)*cos(q6)*sin(q5)*sin(q6))/4 - (3^(1/2)*ddqr4*cos(q4)*cos(q6)*sin(q5)*sin(q6))/4 + (3^(1/2)*ddqr4*cos(q5)*cos(q6)*sin(q4)*sin(q6))/4 + (3^(1/2)*ddqr5*cos(q4)*cos(q6)*sin(q5)*sin(q6))/4 + (3^(1/2)*ddqr5*cos(q5)*cos(q6)*sin(q4)*sin(q6))/2 - (3^(1/2)*ddqr1*cos(q2)*cos(q3)*cos(q4)*cos(q5)^2)/4 - (7*3^(1/2)*ddqr1*cos(q2)*cos(q3)*cos(q4)*cos(q6)^2)/16 - (5*3^(1/2)*ddqr4*cos(q5)*cos(q6)^2*sin(q4)*sin(q5))/8 - (3^(1/2)*ddqr4*cos(q5)^2*cos(q6)*sin(q4)*sin(q6))/2 + (5*3^(1/2)*ddqr1*cos(q2)*cos(q3)*cos(q4)*cos(q5)^2*cos(q6)^2)/16 + (3*ddqr1*cos(q2)*cos(q4)^2*cos(q5)*cos(q6)*sin(q3)*sin(q6))/2 + (3^(1/2)*ddqr1*cos(q2)*cos(q3)*cos(q5)*sin(q4)*sin(q5))/2 + (3^(1/2)*ddqr1*cos(q2)*cos(q3)*cos(q6)*sin(q4)*sin(q6))/4 - (3^(1/2)*ddqr4*cos(q4)*cos(q5)*cos(q6)*sin(q5)*sin(q6))/4 + (3^(1/2)*ddqr1*cos(q2)*cos(q3)*cos(q4)*cos(q5)*cos(q6)^2)/8 + (3^(1/2)*ddqr1*cos(q2)*cos(q3)*cos(q6)^2*sin(q4)*sin(q5))/8 - (3^(1/2)*ddqr1*cos(q2)*cos(q3)*cos(q4)*cos(q6)*sin(q5)*sin(q6))/4 + (3^(1/2)*ddqr1*cos(q2)*cos(q3)*cos(q5)*cos(q6)*sin(q4)*sin(q6))/4 - (5*3^(1/2)*ddqr1*cos(q2)*cos(q3)*cos(q5)*cos(q6)^2*sin(q4)*sin(q5))/8 - (3^(1/2)*ddqr1*cos(q2)*cos(q3)*cos(q5)^2*cos(q6)*sin(q4)*sin(q6))/2 - (3^(1/2)*ddqr1*cos(q2)*cos(q3)*cos(q4)*cos(q5)*cos(q6)*sin(q5)*sin(q6))/4;
Y2_21_1=-sin(q2);
Y2_22_1=cos(q2)*sin(q3) - cos(q3)*sin(q2);
Y2_23_1=- sin(q2)*sin(q3)*sin(q4) - cos(q2)*cos(q3)*sin(q4);
Y2_24_1=(3^(1/2)*cos(q3)*cos(q5)*sin(q2))/2 - (3^(1/2)*cos(q2)*cos(q5)*sin(q3))/2 + cos(q2)*cos(q3)*cos(q4)*sin(q5) + (cos(q2)*cos(q3)*cos(q5)*sin(q4))/2 + cos(q4)*sin(q2)*sin(q3)*sin(q5) + (cos(q5)*sin(q2)*sin(q3)*sin(q4))/2;
Y2_25_1=(3^(1/2)*cos(q3)*cos(q6)*sin(q2))/4 - (3^(1/2)*cos(q2)*cos(q6)*sin(q3))/4 - (3*cos(q2)*cos(q3)*cos(q6)*sin(q4))/4 - (3*cos(q6)*sin(q2)*sin(q3)*sin(q4))/4 + (3^(1/2)*cos(q2)*cos(q5)*cos(q6)*sin(q3))/4 - (3^(1/2)*cos(q3)*cos(q5)*cos(q6)*sin(q2))/4 - (3^(1/2)*cos(q2)*sin(q3)*sin(q5)*sin(q6))/2 + (3^(1/2)*cos(q3)*sin(q2)*sin(q5)*sin(q6))/2 - cos(q2)*cos(q3)*cos(q4)*cos(q5)*sin(q6) - (cos(q2)*cos(q3)*cos(q4)*cos(q6)*sin(q5))/2 - (cos(q2)*cos(q3)*cos(q5)*cos(q6)*sin(q4))/4 + (cos(q2)*cos(q3)*sin(q4)*sin(q5)*sin(q6))/2 - cos(q4)*cos(q5)*sin(q2)*sin(q3)*sin(q6) - (cos(q4)*cos(q6)*sin(q2)*sin(q3)*sin(q5))/2 - (cos(q5)*cos(q6)*sin(q2)*sin(q3)*sin(q4))/4 + (sin(q2)*sin(q3)*sin(q4)*sin(q5)*sin(q6))/2;
Y3_3_1=(1515361*ddqr3)/100000000 - (1515361*ddqr2)/100000000 + (35699*ddqr2*cos(q3))/1000000 - (35699*dq1*dqr1*sin(q3))/2000000 - (35699*dq2*dqr2*sin(q3))/1000000 - (8617*ddqr1*cos(q2)*cos(q3))/10000000 - (8617*ddqr1*sin(q2)*sin(q3))/10000000 + (35699*dq1*dqr1*cos(2*q2)*sin(q3))/2000000 - (35699*dq1*dqr1*sin(2*q2)*cos(q3))/2000000 - (1515361*dq1*dqr1*cos(2*q2)*sin(2*q3))/200000000 + (1515361*dq1*dqr1*cos(2*q3)*sin(2*q2))/200000000;
Y3_4_1=(910321*ddqr3)/25000000 - (910321*ddqr2)/25000000 + (3393*ddqr2*cos(q3))/62500 + (4329*ddqr4*cos(q4))/625000 + (1369*ddqr2*cos(q4)^2)/1000000 - (1369*ddqr3*cos(q4)^2)/1000000 - (3393*dq1*dqr1*sin(q3))/125000 - (3393*dq2*dqr2*sin(q3))/62500 - (4329*dq4*dqr4*sin(q4))/625000 - (1369*dq2*dqr4*sin(2*q4))/2000000 - (1369*dq4*dqr2*sin(2*q4))/2000000 + (1369*dq3*dqr4*sin(2*q4))/2000000 + (1369*dq4*dqr3*sin(2*q4))/2000000 - (819*ddqr1*cos(q2)*cos(q3))/625000 - (819*ddqr1*sin(q2)*sin(q3))/625000 - (1073*ddqr2*sin(q3)*sin(q4))/100000 + (3393*dq1*dqr1*cos(2*q2)*sin(q3))/125000 - (3393*dq1*dqr1*sin(2*q2)*cos(q3))/125000 + (4329*ddqr1*cos(q2)*cos(q3)*cos(q4))/625000 + (259*ddqr1*cos(q2)*sin(q3)*sin(q4))/1000000 - (259*ddqr1*cos(q3)*sin(q2)*sin(q4))/1000000 + (4329*ddqr1*cos(q4)*sin(q2)*sin(q3))/625000 - (1717967*dq1*dqr1*cos(2*q2)*sin(2*q3))/100000000 + (1717967*dq1*dqr1*cos(2*q3)*sin(2*q2))/100000000 - (1073*dq1*dqr1*cos(q3)*sin(q4))/200000 + (1369*dq1*dqr4*cos(q2)*sin(q3))/2000000 - (1369*dq1*dqr4*cos(q3)*sin(q2))/2000000 + (1369*dq4*dqr1*cos(q2)*sin(q3))/2000000 - (1369*dq4*dqr1*cos(q3)*sin(q2))/2000000 - (1073*dq2*dqr2*cos(q3)*sin(q4))/100000 + (1073*dq1*dqr1*cos(2*q2)*cos(q3)*sin(q4))/200000 - (1369*dq1*dqr4*cos(2*q4)*cos(q2)*sin(q3))/2000000 + (1369*dq1*dqr4*cos(2*q4)*cos(q3)*sin(q2))/2000000 - (1369*dq4*dqr1*cos(2*q4)*cos(q2)*sin(q3))/2000000 + (1369*dq4*dqr1*cos(2*q4)*cos(q3)*sin(q2))/2000000 + (1073*dq1*dqr1*sin(2*q2)*sin(q3)*sin(q4))/200000 - (1369*ddqr1*cos(q2)*cos(q4)*sin(q3)*sin(q4))/1000000 + (1369*ddqr1*cos(q3)*cos(q4)*sin(q2)*sin(q4))/1000000 - (4329*dq1*dqr1*cos(2*q2)*cos(2*q3)*sin(q4))/625000 - (4329*dq1*dqr1*sin(2*q2)*sin(2*q3)*sin(q4))/625000 - (4329*dq1*dqr4*cos(q2)*cos(q3)*sin(q4))/625000 - (4329*dq4*dqr1*cos(q2)*cos(q3)*sin(q4))/625000 - (1369*dq1*dqr1*cos(2*q2)*cos(2*q4)*sin(2*q3))/4000000 + (1369*dq1*dqr1*cos(2*q3)*cos(2*q4)*sin(2*q2))/4000000 - (4329*dq1*dqr4*sin(q2)*sin(q3)*sin(q4))/625000 - (4329*dq4*dqr1*sin(q2)*sin(q3)*sin(q4))/625000;
